simulink model "COMPONENT_MDL_Lag_QUAD_and_PEND_with_spin_rotors"  (R2021b)
settings: Solver=ode23t  StartTime=0.0  StopTime=200  FixedStep=0.001  RelTol=1e-5  EnableMultiTasking=on
undefined symbols (not defined in the file or in its folder): P_pend, P_rot, P_veh_no_props
(part 2 of 10)

== matlab function COMPONENT_MDL_Lag_QUAD_and_PEND_with_spin_rotors/bh_6DOF_and_pend/MCKGQ ==
  data: I_xx input; M output; I_xy input; I_xz input; I_yy input; I_yz input; I_zz input; Iprop_xx input; Iprop_xy input; Iprop_xz input; Iprop_yy input; Iprop_yz input; Iprop_zz input; Lx_pend input; Ly_pend input; Lz_pend input; Mbz_1 input; Mbz_2 input; Mbz_3 input; Mbz_4 input; THE_Phi input; THE_Psi input; THE_Phi_D input; THE_Psi_D input; THE_Theta input; THE_Theta_D input; THE_Phi_pend input; THE_Psi_pend input; THE_Phi_pend_D input; THE_Psi_pend_D input; THE_Theta_pend input; THE_Theta_pend_D input; Tbz_1 input; Tbz_2 input; Tbz_3 input; Tbz_4 input; Tv_Z_pend input; cg_to_mot_H input; cg_to_mot_L input; g input; m input; m_pend input; mprop input; wMOT_1 input; wMOT_2 input; wMOT_3 input; wMOT_4 input; C output; K output; G output; Q output
function [M,C,K,G,Q] = MCKGQ(I_xx,I_xy,I_xz,I_yy,I_yz,I_zz,Iprop_xx,Iprop_xy,Iprop_xz,Iprop_yy,Iprop_yz,Iprop_zz,Lx_pend,Ly_pend,Lz_pend,Mbz_1,Mbz_2,Mbz_3,Mbz_4,THE_Phi,THE_Psi,THE_Phi_D,THE_Psi_D,THE_Theta,THE_Theta_D,THE_Phi_pend,THE_Psi_pend,THE_Phi_pend_D,THE_Psi_pend_D,THE_Theta_pend,THE_Theta_pend_D,Tbz_1,Tbz_2,Tbz_3,Tbz_4,Tv_Z_pend,cg_to_mot_H,cg_to_mot_L,g,m,m_pend,mprop,wMOT_1,wMOT_2,wMOT_3,wMOT_4)
%#codegen

%    This function was generated by the Symbolic Math Toolbox version 9.0.
%    29-Sep-2021 14:44:32

et1 = (Lx_pend.^2.*m_pend.*sin(THE_Theta).*sin(THE_Phi_pend))./1.2e+1+(Ly_pend.^2.*m_pend.*sin(THE_Theta).*sin(THE_Phi_pend))./1.2e+1-(Ly_pend.^2.*m_pend.*cos(THE_Psi_pend).^2.*sin(THE_Theta).*sin(THE_Phi_pend))./1.2e+1+(Lz_pend.^2.*m_pend.*cos(THE_Psi_pend).^2.*sin(THE_Theta).*sin(THE_Phi_pend))./3.0+(Lx_pend.^2.*m_pend.*cos(THE_Theta).*cos(THE_Phi_pend).*sin(THE_Psi))./1.2e+1+(Ly_pend.^2.*m_pend.*cos(THE_Theta).*cos(THE_Phi_pend).*sin(THE_Psi))./1.2e+1-(Ly_pend.^2.*m_pend.*cos(THE_Theta).*cos(THE_Phi_pend).*cos(THE_Psi_pend).^2.*sin(THE_Psi))./1.2e+1+(Lz_pend.^2.*m_pend.*cos(THE_Theta).*cos(THE_Phi_pend).*cos(THE_Psi_pend).^2.*sin(THE_Psi))./3.0-(Ly_pend.^2.*m_pend.*cos(THE_Psi).*cos(THE_Theta).*cos(THE_Psi_pend).*cos(THE_Theta_pend).*sin(THE_Psi_pend))./1.2e+1+(Lz_pend.^2.*m_pend.*cos(THE_Psi).*cos(THE_Theta).*cos(THE_Psi_pend).*cos(THE_Theta_pend).*sin(THE_Psi_pend))./3.0+(Ly_pend.^2.*m_pend.*cos(THE_Phi_pend).*cos(THE_Psi_pend).*sin(THE_Theta).*sin(THE_Psi_pend).*sin(THE_Theta_pend))./1.2e+1;
et2 = Lz_pend.^2.*m_pend.*cos(THE_Phi_pend).*cos(THE_Psi_pend).*sin(THE_Theta).*sin(THE_Psi_pend).*sin(THE_Theta_pend).*(-1.0./3.0)+(Lz_pend.*Tv_Z_pend.*m_pend.*cos(THE_Psi_pend).*cos(THE_Theta_pend).*sin(THE_Theta).*sin(THE_Phi_pend))./2.0-(Ly_pend.^2.*m_pend.*cos(THE_Theta).*cos(THE_Psi_pend).*sin(THE_Psi).*sin(THE_Phi_pend).*sin(THE_Psi_pend).*sin(THE_Theta_pend))./1.2e+1+(Lz_pend.^2.*m_pend.*cos(THE_Theta).*cos(THE_Psi_pend).*sin(THE_Psi).*sin(THE_Phi_pend).*sin(THE_Psi_pend).*sin(THE_Theta_pend))./3.0+(Lz_pend.*Tv_Z_pend.*m_pend.*cos(THE_Theta).*cos(THE_Phi_pend).*cos(THE_Psi_pend).*cos(THE_Theta_pend).*sin(THE_Psi))./2.0;
et3 = (Ly_pend.^2.*m_pend.*cos(THE_Psi).*cos(THE_Theta))./1.2e+1+(Lz_pend.^2.*m_pend.*cos(THE_Psi).*cos(THE_Theta))./3.0+(Lx_pend.^2.*m_pend.*cos(THE_Psi).*cos(THE_Theta).*cos(THE_Theta_pend).^2)./1.2e+1-(Ly_pend.^2.*m_pend.*cos(THE_Psi).*cos(THE_Theta).*cos(THE_Theta_pend).^2)./1.2e+1+(Ly_pend.^2.*m_pend.*cos(THE_Psi).*cos(THE_Theta).*cos(THE_Psi_pend).^2.*cos(THE_Theta_pend).^2)./1.2e+1-(Lz_pend.^2.*m_pend.*cos(THE_Psi).*cos(THE_Theta).*cos(THE_Psi_pend).^2.*cos(THE_Theta_pend).^2)./3.0-(Lx_pend.^2.*m_pend.*cos(THE_Phi_pend).*cos(THE_Theta_pend).*sin(THE_Theta).*sin(THE_Theta_pend))./1.2e+1+(Ly_pend.^2.*m_pend.*cos(THE_Phi_pend).*cos(THE_Theta_pend).*sin(THE_Theta).*sin(THE_Theta_pend))./1.2e+1+(Lz_pend.*Tv_Z_pend.*m_pend.*sin(THE_Theta).*sin(THE_Phi_pend).*sin(THE_Psi_pend))./2.0+(Lx_pend.^2.*m_pend.*cos(THE_Theta).*cos(THE_Theta_pend).*sin(THE_Psi).*sin(THE_Phi_pend).*sin(THE_Theta_pend))./1.2e+1-(Ly_pend.^2.*m_pend.*cos(THE_Theta).*cos(THE_Theta_pend).*sin(THE_Psi).*sin(THE_Phi_pend).*sin(THE_Theta_pend))./1.2e+1;
et4 = Ly_pend.^2.*m_pend.*cos(THE_Psi_pend).*cos(THE_Theta_pend).*sin(THE_Theta).*sin(THE_Phi_pend).*sin(THE_Psi_pend).*(-1.0./1.2e+1)+(Lz_pend.^2.*m_pend.*cos(THE_Psi_pend).*cos(THE_Theta_pend).*sin(THE_Theta).*sin(THE_Phi_pend).*sin(THE_Psi_pend))./3.0+(Lz_pend.*Tv_Z_pend.*m_pend.*cos(THE_Theta).*cos(THE_Phi_pend).*sin(THE_Psi).*sin(THE_Psi_pend))./2.0+(Lz_pend.*Tv_Z_pend.*m_pend.*cos(THE_Phi_pend).*cos(THE_Psi_pend).*sin(THE_Theta).*sin(THE_Theta_pend))./2.0-(Ly_pend.^2.*m_pend.*cos(THE_Phi_pend).*cos(THE_Psi_pend).^2.*cos(THE_Theta_pend).*sin(THE_Theta).*sin(THE_Theta_pend))./1.2e+1+(Lz_pend.^2.*m_pend.*cos(THE_Phi_pend).*cos(THE_Psi_pend).^2.*cos(THE_Theta_pend).*sin(THE_Theta).*sin(THE_Theta_pend))./3.0-(Lz_pend.*Tv_Z_pend.*m_pend.*cos(THE_Theta).*cos(THE_Psi_pend).*sin(THE_Psi).*sin(THE_Phi_pend).*sin(THE_Theta_pend))./2.0+(Ly_pend.^2.*m_pend.*cos(THE_Theta).*cos(THE_Psi_pend).^2.*cos(THE_Theta_pend).*sin(THE_Psi).*sin(THE_Phi_pend).*sin(THE_Theta_pend))./1.2e+1-(Lz_pend.^2.*m_pend.*cos(THE_Theta).*cos(THE_Psi_pend).^2.*cos(THE_Theta_pend).*sin(THE_Psi).*sin(THE_Phi_pend).*sin(THE_Theta_pend))./3.0-(Ly_pend.^2.*m_pend.*cos(THE_Theta).*cos(THE_Phi_pend).*cos(THE_Psi_pend).*cos(THE_Theta_pend).*sin(THE_Psi).*sin(THE_Psi_pend))./1.2e+1;
et5 = (Lz_pend.^2.*m_pend.*cos(THE_Theta).*cos(THE_Phi_pend).*cos(THE_Psi_pend).*cos(THE_Theta_pend).*sin(THE_Psi).*sin(THE_Psi_pend))./3.0;
et6 = -I_xx.*sin(THE_Theta)-Iprop_xx.*sin(THE_Theta).*4.0+I_xz.*cos(THE_Psi).*cos(THE_Theta)+Iprop_xz.*cos(THE_Psi).*cos(THE_Theta).*4.0+I_xy.*cos(THE_Theta).*sin(THE_Psi)+Iprop_xy.*cos(THE_Theta).*sin(THE_Psi).*4.0-(Lx_pend.^2.*m_pend.*sin(THE_Theta))./1.2e+1-(Ly_pend.^2.*m_pend.*sin(THE_Theta))./1.2e+1-Tv_Z_pend.^2.*m_pend.*sin(THE_Theta)-cg_to_mot_H.^2.*mprop.*sin(THE_Theta).*4.0-cg_to_mot_L.^2.*mprop.*sin(THE_Theta).*2.0+(Ly_pend.^2.*m_pend.*cos(THE_Phi_pend).^2.*sin(THE_Theta))./1.2e+1+(Ly_pend.^2.*m_pend.*cos(THE_Psi_pend).^2.*sin(THE_Theta))./1.2e+1-(Lz_pend.^2.*m_pend.*cos(THE_Phi_pend).^2.*sin(THE_Theta))./3.0-(Lz_pend.^2.*m_pend.*cos(THE_Psi_pend).^2.*sin(THE_Theta))./3.0+(Lx_pend.^2.*m_pend.*cos(THE_Phi_pend).^2.*cos(THE_Theta_pend).^2.*sin(THE_Theta))./1.2e+1-(Ly_pend.^2.*m_pend.*cos(THE_Phi_pend).^2.*cos(THE_Psi_pend).^2.*sin(THE_Theta))./6.0;
et7 = Ly_pend.^2.*m_pend.*cos(THE_Phi_pend).^2.*cos(THE_Theta_pend).^2.*sin(THE_Theta).*(-1.0./1.2e+1)+Lz_pend.^2.*m_pend.*cos(THE_Phi_pend).^2.*cos(THE_Psi_pend).^2.*sin(THE_Theta).*(2.0./3.0)-(Ly_pend.^2.*m_pend.*cos(THE_Theta).*cos(THE_Phi_pend).*sin(THE_Psi).*sin(THE_Phi_pend))./1.2e+1+(Lz_pend.^2.*m_pend.*cos(THE_Theta).*cos(THE_Phi_pend).*sin(THE_Psi).*sin(THE_Phi_pend))./3.0+(Ly_pend.^2.*m_pend.*cos(THE_Phi_pend).^2.*cos(THE_Psi_pend).^2.*cos(THE_Theta_pend).^2.*sin(THE_Theta))./1.2e+1-(Lz_pend.^2.*m_pend.*cos(THE_Phi_pend).^2.*cos(THE_Psi_pend).^2.*cos(THE_Theta_pend).^2.*sin(THE_Theta))./3.0-Lz_pend.*Tv_Z_pend.*m_pend.*cos(THE_Psi_pend).*cos(THE_Theta_pend).*sin(THE_Theta)+(Lx_pend.^2.*m_pend.*cos(THE_Psi).*cos(THE_Theta).*cos(THE_Phi_pend).*cos(THE_Theta_pend).*sin(THE_Theta_pend))./1.2e+1-(Ly_pend.^2.*m_pend.*cos(THE_Psi).*cos(THE_Theta).*cos(THE_Phi_pend).*cos(THE_Theta_pend).*sin(THE_Theta_pend))./1.2e+1+(Ly_pend.^2.*m_pend.*cos(THE_Theta).*cos(THE_Psi_pend).*sin(THE_Psi).*sin(THE_Psi_pend).*sin(THE_Theta_pend))./1.2e+1;
et8 = Lz_pend.^2.*m_pend.*cos(THE_Theta).*cos(THE_Psi_pend).*sin(THE_Psi).*sin(THE_Psi_pend).*sin(THE_Theta_pend).*(-1.0./3.0)-(Lz_pend.*Tv_Z_pend.*m_pend.*cos(THE_Psi).*cos(THE_Theta).*sin(THE_Phi_pend).*sin(THE_Psi_pend))./2.0-(Lx_pend.^2.*m_pend.*cos(THE_Theta).*cos(THE_Phi_pend).*cos(THE_Theta_pend).^2.*sin(THE_Psi).*sin(THE_Phi_pend))./1.2e+1+(Ly_pend.^2.*m_pend.*cos(THE_Theta).*cos(THE_Phi_pend).*cos(THE_Psi_pend).^2.*sin(THE_Psi).*sin(THE_Phi_pend))./6.0+(Ly_pend.^2.*m_pend.*cos(THE_Theta).*cos(THE_Phi_pend).*cos(THE_Theta_pend).^2.*sin(THE_Psi).*sin(THE_Phi_pend))./1.2e+1-Lz_pend.^2.*m_pend.*cos(THE_Theta).*cos(THE_Phi_pend).*cos(THE_Psi_pend).^2.*sin(THE_Psi).*sin(THE_Phi_pend).*(2.0./3.0)-(Ly_pend.^2.*m_pend.*cos(THE_Phi_pend).*cos(THE_Psi_pend).*sin(THE_Theta).*sin(THE_Phi_pend).*sin(THE_Psi_pend).*sin(THE_Theta_pend))./6.0+Lz_pend.^2.*m_pend.*cos(THE_Phi_pend).*cos(THE_Psi_pend).*sin(THE_Theta).*sin(THE_Phi_pend).*sin(THE_Psi_pend).*sin(THE_Theta_pend).*(2.0./3.0)-(Lz_pend.*Tv_Z_pend.*m_pend.*cos(THE_Psi).*cos(THE_Theta).*cos(THE_Phi_pend).*cos(THE_Psi_pend).*sin(THE_Theta_pend))./2.0;
et9 = (Ly_pend.^2.*m_pend.*cos(THE_Psi).*cos(THE_Theta).*cos(THE_Phi_pend).*cos(THE_Psi_pend).^2.*cos(THE_Theta_pend).*sin(THE_Theta_pend))./1.2e+1-(Lz_pend.^2.*m_pend.*cos(THE_Psi).*cos(THE_Theta).*cos(THE_Phi_pend).*cos(THE_Psi_pend).^2.*cos(THE_Theta_pend).*sin(THE_Theta_pend))./3.0-(Ly_pend.^2.*m_pend.*cos(THE_Theta).*cos(THE_Phi_pend).^2.*cos(THE_Psi_pend).*sin(THE_Psi).*sin(THE_Psi_pend).*sin(THE_Theta_pend))./6.0+Lz_pend.^2.*m_pend.*cos(THE_Theta).*cos(THE_Phi_pend).^2.*cos(THE_Psi_pend).*sin(THE_Psi).*sin(THE_Psi_pend).*sin(THE_Theta_pend).*(2.0./3.0)-(Ly_pend.^2.*m_pend.*cos(THE_Theta).*cos(THE_Phi_pend).*cos(THE_Psi_pend).^2.*cos(THE_Theta_pend).^2.*sin(THE_Psi).*sin(THE_Phi_pend))./1.2e+1+(Lz_pend.^2.*m_pend.*cos(THE_Theta).*cos(THE_Phi_pend).*cos(THE_Psi_pend).^2.*cos(THE_Theta_pend).^2.*sin(THE_Psi).*sin(THE_Phi_pend))./3.0+(Ly_pend.^2.*m_pend.*cos(THE_Psi).*cos(THE_Theta).*cos(THE_Psi_pend).*cos(THE_Theta_pend).*sin(THE_Phi_pend).*sin(THE_Psi_pend))./1.2e+1-(Lz_pend.^2.*m_pend.*cos(THE_Psi).*cos(THE_Theta).*cos(THE_Psi_pend).*cos(THE_Theta_pend).*sin(THE_Phi_pend).*sin(THE_Psi_pend))./3.0;
et10 = -I_yz.*cos(THE_Theta)-Iprop_yz.*cos(THE_Theta).*4.0-I_xy.*cos(THE_Psi).*sin(THE_Theta)-Iprop_xy.*cos(THE_Psi).*sin(THE_Theta).*4.0+I_xz.*sin(THE_Psi).*sin(THE_Theta)+Iprop_xz.*sin(THE_Psi).*sin(THE_Theta).*4.0+I_yz.*cos(THE_Psi).^2.*cos(THE_Theta).*2.0+Iprop_yz.*cos(THE_Psi).^2.*cos(THE_Theta).*8.0+I_yy.*cos(THE_Psi).*cos(THE_Theta).*sin(THE_Psi)-I_zz.*cos(THE_Psi).*cos(THE_Theta).*sin(THE_Psi)+Iprop_yy.*cos(THE_Psi).*cos(THE_Theta).*sin(THE_Psi).*4.0-Iprop_zz.*cos(THE_Psi).*cos(THE_Theta).*sin(THE_Psi).*4.0+(Lx_pend.^2.*m_pend.*cos(THE_Psi).*cos(THE_Theta).*sin(THE_Psi))./1.2e+1-(Ly_pend.^2.*m_pend.*cos(THE_Psi).*cos(THE_Theta).*sin(THE_Psi))./1.2e+1+Tv_Z_pend.^2.*m_pend.*cos(THE_Psi).*cos(THE_Theta).*sin(THE_Psi)+cg_to_mot_H.^2.*mprop.*cos(THE_Psi).*cos(THE_Theta).*sin(THE_Psi).*4.0-cg_to_mot_L.^2.*mprop.*cos(THE_Psi).*cos(THE_Theta).*sin(THE_Psi).*2.0-(Lx_pend.^2.*m_pend.*cos(THE_Theta).*cos(THE_Theta_pend).*sin(THE_Phi_pend).*sin(THE_Theta_pend))./1.2e+1+(Ly_pend.^2.*m_pend.*cos(THE_Psi).*cos(THE_Phi_pend).*sin(THE_Theta).*sin(THE_Phi_pend))./1.2e+1;
et11 = (Ly_pend.^2.*m_pend.*cos(THE_Theta).*cos(THE_Theta_pend).*sin(THE_Phi_pend).*sin(THE_Theta_pend))./1.2e+1-(Lz_pend.^2.*m_pend.*cos(THE_Psi).*cos(THE_Phi_pend).*sin(THE_Theta).*sin(THE_Phi_pend))./3.0-(Lz_pend.*Tv_Z_pend.*m_pend.*cos(THE_Theta).*cos(THE_Phi_pend).*sin(THE_Psi_pend))./2.0-(Lx_pend.^2.*m_pend.*cos(THE_Psi).*cos(THE_Theta).*cos(THE_Theta_pend).^2.*sin(THE_Psi))./6.0+(Ly_pend.^2.*m_pend.*cos(THE_Psi).*cos(THE_Theta).*cos(THE_Phi_pend).^2.*sin(THE_Psi))./1.2e+1+(Ly_pend.^2.*m_pend.*cos(THE_Psi).*cos(THE_Theta).*cos(THE_Psi_pend).^2.*sin(THE_Psi))./1.2e+1+(Ly_pend.^2.*m_pend.*cos(THE_Psi).*cos(THE_Theta).*cos(THE_Theta_pend).^2.*sin(THE_Psi))./6.0-(Lz_pend.^2.*m_pend.*cos(THE_Psi).*cos(THE_Theta).*cos(THE_Phi_pend).^2.*sin(THE_Psi))./3.0-(Lz_pend.^2.*m_pend.*cos(THE_Psi).*cos(THE_Theta).*cos(THE_Psi_pend).^2.*sin(THE_Psi))./3.0+(Ly_pend.^2.*m_pend.*cos(THE_Theta).*cos(THE_Phi_pend).*cos(THE_Psi_pend).*cos(THE_Theta_pend).*sin(THE_Psi_pend))./1.2e+1-(Lz_pend.^2.*m_pend.*cos(THE_Theta).*cos(THE_Phi_pend).*cos(THE_Psi_pend).*cos(THE_Theta_pend).*sin(THE_Psi_pend))./3.0;
et12 = (Lx_pend.^2.*m_pend.*cos(THE_Phi_pend).*cos(THE_Theta_pend).*sin(THE_Psi).*sin(THE_Theta).*sin(THE_Theta_pend))./1.2e+1-(Ly_pend.^2.*m_pend.*cos(THE_Psi).*cos(THE_Psi_pend).*sin(THE_Theta).*sin(THE_Psi_pend).*sin(THE_Theta_pend))./1.2e+1-(Ly_pend.^2.*m_pend.*cos(THE_Phi_pend).*cos(THE_Theta_pend).*sin(THE_Psi).*sin(THE_Theta).*sin(THE_Theta_pend))./1.2e+1+(Lz_pend.^2.*m_pend.*cos(THE_Psi).*cos(THE_Psi_pend).*sin(THE_Theta).*sin(THE_Psi_pend).*sin(THE_Theta_pend))./3.0+(Lz_pend.*Tv_Z_pend.*m_pend.*cos(THE_Theta).*cos(THE_Psi_pend).*sin(THE_Phi_pend).*sin(THE_Theta_pend))./2.0-(Lz_pend.*Tv_Z_pend.*m_pend.*sin(THE_Psi).*sin(THE_Theta).*sin(THE_Phi_pend).*sin(THE_Psi_pend))./2.0+(Lx_pend.^2.*m_pend.*cos(THE_Psi).*cos(THE_Phi_pend).*cos(THE_Theta_pend).^2.*sin(THE_Theta).*sin(THE_Phi_pend))./1.2e+1+(Lx_pend.^2.*m_pend.*cos(THE_Psi).^2.*cos(THE_Theta).*cos(THE_Theta_pend).*sin(THE_Phi_pend).*sin(THE_Theta_pend))./6.0-(Ly_pend.^2.*m_pend.*cos(THE_Psi).*cos(THE_Phi_pend).*cos(THE_Psi_pend).^2.*sin(THE_Theta).*sin(THE_Phi_pend))./6.0-(Ly_pend.^2.*m_pend.*cos(THE_Psi).*cos(THE_Phi_pend).*cos(THE_Theta_pend).^2.*sin(THE_Theta).*sin(THE_Phi_pend))./1.2e+1;
et13 = Ly_pend.^2.*m_pend.*cos(THE_Psi).^2.*cos(THE_Theta).*cos(THE_Theta_pend).*sin(THE_Phi_pend).*sin(THE_Theta_pend).*(-1.0./6.0)-(Ly_pend.^2.*m_pend.*cos(THE_Theta).*cos(THE_Psi_pend).^2.*cos(THE_Theta_pend).*sin(THE_Phi_pend).*sin(THE_Theta_pend))./1.2e+1+Lz_pend.^2.*m_pend.*cos(THE_Psi).*cos(THE_Phi_pend).*cos(THE_Psi_pend).^2.*sin(THE_Theta).*sin(THE_Phi_pend).*(2.0./3.0)+(Lz_pend.^2.*m_pend.*cos(THE_Theta).*cos(THE_Psi_pend).^2.*cos(THE_Theta_pend).*sin(THE_Phi_pend).*sin(THE_Theta_pend))./3.0+Lz_pend.*Tv_Z_pend.*m_pend.*cos(THE_Psi).^2.*cos(THE_Theta).*cos(THE_Phi_pend).*sin(THE_Psi_pend)+(Lx_pend.^2.*m_pend.*cos(THE_Psi).*cos(THE_Theta).*cos(THE_Phi_pend).^2.*cos(THE_Theta_pend).^2.*sin(THE_Psi))./1.2e+1-(Ly_pend.^2.*m_pend.*cos(THE_Psi).*cos(THE_Theta).*cos(THE_Phi_pend).^2.*cos(THE_Psi_pend).^2.*sin(THE_Psi))./6.0-(Ly_pend.^2.*m_pend.*cos(THE_Psi).*cos(THE_Theta).*cos(THE_Phi_pend).^2.*cos(THE_Theta_pend).^2.*sin(THE_Psi))./1.2e+1-(Ly_pend.^2.*m_pend.*cos(THE_Psi).*cos(THE_Theta).*cos(THE_Psi_pend).^2.*cos(THE_Theta_pend).^2.*sin(THE_Psi))./6.0;
et14 = Lz_pend.^2.*m_pend.*cos(THE_Psi).*cos(THE_Theta).*cos(THE_Phi_pend).^2.*cos(THE_Psi_pend).^2.*sin(THE_Psi).*(2.0./3.0)+Lz_pend.^2.*m_pend.*cos(THE_Psi).*cos(THE_Theta).*cos(THE_Psi_pend).^2.*cos(THE_Theta_pend).^2.*sin(THE_Psi).*(2.0./3.0)+(Ly_pend.^2.*m_pend.*cos(THE_Psi_pend).*cos(THE_Theta_pend).*sin(THE_Psi).*sin(THE_Theta).*sin(THE_Phi_pend).*sin(THE_Psi_pend))./1.2e+1-(Lz_pend.^2.*m_pend.*cos(THE_Psi_pend).*cos(THE_Theta_pend).*sin(THE_Psi).*sin(THE_Theta).*sin(THE_Phi_pend).*sin(THE_Psi_pend))./3.0+Lz_pend.*Tv_Z_pend.*m_pend.*cos(THE_Psi).*cos(THE_Theta).*cos(THE_Psi_pend).*cos(THE_Theta_pend).*sin(THE_Psi)-(Lz_pend.*Tv_Z_pend.*m_pend.*cos(THE_Phi_pend).*cos(THE_Psi_pend).*sin(THE_Psi).*sin(THE_Theta).*sin(THE_Theta_pend))./2.0-(Ly_pend.^2.*m_pend.*cos(THE_Psi).^2.*cos(THE_Theta).*cos(THE_Phi_pend).*cos(THE_Psi_pend).*cos(THE_Theta_pend).*sin(THE_Psi_pend))./6.0+Lz_pend.^2.*m_pend.*cos(THE_Psi).^2.*cos(THE_Theta).*cos(THE_Phi_pend).*cos(THE_Psi_pend).*cos(THE_Theta_pend).*sin(THE_Psi_pend).*(2.0./3.0)+(Ly_pend.^2.*m_pend.*cos(THE_Psi).*cos(THE_Phi_pend).^2.*cos(THE_Psi_pend).*sin(THE_Theta).*sin(THE_Psi_pend).*sin(THE_Theta_pend))./6.0;
et15 = (Ly_pend.^2.*m_pend.*cos(THE_Phi_pend).*cos(THE_Psi_pend).^2.*cos(THE_Theta_pend).*sin(THE_Psi).*sin(THE_Theta).*sin(THE_Theta_pend))./1.2e+1-Lz_pend.^2.*m_pend.*cos(THE_Psi).*cos(THE_Phi_pend).^2.*cos(THE_Psi_pend).*sin(THE_Theta).*sin(THE_Psi_pend).*sin(THE_Theta_pend).*(2.0./3.0)-(Lz_pend.^2.*m_pend.*cos(THE_Phi_pend).*cos(THE_Psi_pend).^2.*cos(THE_Theta_pend).*sin(THE_Psi).*sin(THE_Theta).*sin(THE_Theta_pend))./3.0-Lz_pend.*Tv_Z_pend.*m_pend.*cos(THE_Psi).^2.*cos(THE_Theta).*cos(THE_Psi_pend).*sin(THE_Phi_pend).*sin(THE_Theta_pend)+(Ly_pend.^2.*m_pend.*cos(THE_Psi).*cos(THE_Phi_pend).*cos(THE_Psi_pend).^2.*cos(THE_Theta_pend).^2.*sin(THE_Theta).*sin(THE_Phi_pend))./1.2e+1+(Ly_pend.^2.*m_pend.*cos(THE_Psi).^2.*cos(THE_Theta).*cos(THE_Psi_pend).^2.*cos(THE_Theta_pend).*sin(THE_Phi_pend).*sin(THE_Theta_pend))./6.0-(Lz_pend.^2.*m_pend.*cos(THE_Psi).*cos(THE_Phi_pend).*cos(THE_Psi_pend).^2.*cos(THE_Theta_pend).^2.*sin(THE_Theta).*sin(THE_Phi_pend))./3.0-Lz_pend.^2.*m_pend.*cos(THE_Psi).^2.*cos(THE_Theta).*cos(THE_Psi_pend).^2.*cos(THE_Theta_pend).*sin(THE_Phi_pend).*sin(THE_Theta_pend).*(2.0./3.0);
et16 = (Ly_pend.^2.*m_pend.*cos(THE_Psi).*cos(THE_Theta).*cos(THE_Phi_pend).^2.*cos(THE_Psi_pend).^2.*cos(THE_Theta_pend).^2.*sin(THE_Psi))./1.2e+1-(Lz_pend.^2.*m_pend.*cos(THE_Psi).*cos(THE_Theta).*cos(THE_Phi_pend).^2.*cos(THE_Psi_pend).^2.*cos(THE_Theta_pend).^2.*sin(THE_Psi))./3.0-(Ly_pend.^2.*m_pend.*cos(THE_Psi).*cos(THE_Theta).*cos(THE_Phi_pend).*cos(THE_Psi_pend).*sin(THE_Psi).*sin(THE_Phi_pend).*sin(THE_Psi_pend).*sin(THE_Theta_pend))./6.0+Lz_pend.^2.*m_pend.*cos(THE_Psi).*cos(THE_Theta).*cos(THE_Phi_pend).*cos(THE_Psi_pend).*sin(THE_Psi).*sin(THE_Phi_pend).*sin(THE_Psi_pend).*sin(THE_Theta_pend).*(2.0./3.0);
et17 = I_xx+Iprop_xx.*4.0+(Lx_pend.^2.*m_pend)./1.2e+1+(Ly_pend.^2.*m_pend)./1.2e+1+Tv_Z_pend.^2.*m_pend+cg_to_mot_H.^2.*mprop.*4.0+cg_to_mot_L.^2.*mprop.*2.0-I_xx.*cos(THE_Theta).^2+I_yy.*cos(THE_Theta).^2-Iprop_xx.*cos(THE_Theta).^2.*4.0+Iprop_yy.*cos(THE_Theta).^2.*4.0-(Ly_pend.^2.*m_pend.*cos(THE_Theta).^2)./1.2e+1-(Ly_pend.^2.*m_pend.*cos(THE_Phi_pend).^2)./1.2e+1-(Ly_pend.^2.*m_pend.*cos(THE_Psi_pend).^2)./1.2e+1+(Lz_pend.^2.*m_pend.*cos(THE_Theta).^2)./3.0+(Lz_pend.^2.*m_pend.*cos(THE_Phi_pend).^2)./3.0+(Lz_pend.^2.*m_pend.*cos(THE_Psi_pend).^2)./3.0-I_yy.*cos(THE_Psi).^2.*cos(THE_Theta).^2+I_zz.*cos(THE_Psi).^2.*cos(THE_Theta).^2-Iprop_yy.*cos(THE_Psi).^2.*cos(THE_Theta).^2.*4.0+Iprop_zz.*cos(THE_Psi).^2.*cos(THE_Theta).^2.*4.0;
et18 = I_yz.*cos(THE_Psi).*cos(THE_Theta).^2.*sin(THE_Psi).*2.0+Iprop_yz.*cos(THE_Psi).*cos(THE_Theta).^2.*sin(THE_Psi).*8.0-(Lx_pend.^2.*m_pend.*cos(THE_Psi).^2.*cos(THE_Theta).^2)./1.2e+1-(Lx_pend.^2.*m_pend.*cos(THE_Theta).^2.*cos(THE_Theta_pend).^2)./1.2e+1-(Lx_pend.^2.*m_pend.*cos(THE_Phi_pend).^2.*cos(THE_Theta_pend).^2)./1.2e+1+(Ly_pend.^2.*m_pend.*cos(THE_Psi).^2.*cos(THE_Theta).^2)./1.2e+1+(Ly_pend.^2.*m_pend.*cos(THE_Theta).^2.*cos(THE_Phi_pend).^2)./6.0+(Ly_pend.^2.*m_pend.*cos(THE_Theta).^2.*cos(THE_Psi_pend).^2)./6.0+(Ly_pend.^2.*m_pend.*cos(THE_Theta).^2.*cos(THE_Theta_pend).^2)./1.2e+1+(Ly_pend.^2.*m_pend.*cos(THE_Phi_pend).^2.*cos(THE_Psi_pend).^2)./6.0+(Ly_pend.^2.*m_pend.*cos(THE_Phi_pend).^2.*cos(THE_Theta_pend).^2)./1.2e+1-Lz_pend.^2.*m_pend.*cos(THE_Theta).^2.*cos(THE_Phi_pend).^2.*(2.0./3.0);
et19 = Lz_pend.^2.*m_pend.*cos(THE_Theta).^2.*cos(THE_Psi_pend).^2.*(-2.0./3.0)-Lz_pend.^2.*m_pend.*cos(THE_Phi_pend).^2.*cos(THE_Psi_pend).^2.*(2.0./3.0)-Tv_Z_pend.^2.*m_pend.*cos(THE_Psi).^2.*cos(THE_Theta).^2-cg_to_mot_H.^2.*mprop.*cos(THE_Psi).^2.*cos(THE_Theta).^2.*4.0+cg_to_mot_L.^2.*mprop.*cos(THE_Psi).^2.*cos(THE_Theta).^2.*2.0-I_xz.*cos(THE_Psi).*cos(THE_Theta).*sin(THE_Theta).*2.0-Iprop_xz.*cos(THE_Psi).*cos(THE_Theta).*sin(THE_Theta).*8.0-I_xy.*cos(THE_Theta).*sin(THE_Psi).*sin(THE_Theta).*2.0-Iprop_xy.*cos(THE_Theta).*sin(THE_Psi).*sin(THE_Theta).*8.0+(Lx_pend.^2.*m_pend.*cos(THE_Psi).^2.*cos(THE_Theta).^2.*cos(THE_Theta_pend).^2)./6.0+(Lx_pend.^2.*m_pend.*cos(THE_Theta).^2.*cos(THE_Phi_pend).^2.*cos(THE_Theta_pend).^2)./6.0-(Ly_pend.^2.*m_pend.*cos(THE_Psi).^2.*cos(THE_Theta).^2.*cos(THE_Phi_pend).^2)./1.2e+1;
et20 = Ly_pend.^2.*m_pend.*cos(THE_Psi).^2.*cos(THE_Theta).^2.*cos(THE_Psi_pend).^2.*(-1.0./1.2e+1)-(Ly_pend.^2.*m_pend.*cos(THE_Psi).^2.*cos(THE_Theta).^2.*cos(THE_Theta_pend).^2)./6.0-(Ly_pend.^2.*m_pend.*cos(THE_Theta).^2.*cos(THE_Phi_pend).^2.*cos(THE_Psi_pend).^2)./3.0-(Ly_pend.^2.*m_pend.*cos(THE_Theta).^2.*cos(THE_Phi_pend).^2.*cos(THE_Theta_pend).^2)./6.0-(Ly_pend.^2.*m_pend.*cos(THE_Theta).^2.*cos(THE_Psi_pend).^2.*cos(THE_Theta_pend).^2)./1.2e+1-(Ly_pend.^2.*m_pend.*cos(THE_Phi_pend).^2.*cos(THE_Psi_pend).^2.*cos(THE_Theta_pend).^2)./1.2e+1+(Lz_pend.^2.*m_pend.*cos(THE_Psi).^2.*cos(THE_Theta).^2.*cos(THE_Phi_pend).^2)./3.0+(Lz_pend.^2.*m_pend.*cos(THE_Psi).^2.*cos(THE_Theta).^2.*cos(THE_Psi_pend).^2)./3.0+Lz_pend.^2.*m_pend.*cos(THE_Theta).^2.*cos(THE_Phi_pend).^2.*cos(THE_Psi_pend).^2.*(4.0./3.0);
et21 = (Lz_pend.^2.*m_pend.*cos(THE_Theta).^2.*cos(THE_Psi_pend).^2.*cos(THE_Theta_pend).^2)./3.0+(Lz_pend.^2.*m_pend.*cos(THE_Phi_pend).^2.*cos(THE_Psi_pend).^2.*cos(THE_Theta_pend).^2)./3.0+Lz_pend.*Tv_Z_pend.*m_pend.*cos(THE_Psi_pend).*cos(THE_Theta_pend)-(Lx_pend.^2.*m_pend.*cos(THE_Psi).^2.*cos(THE_Theta).^2.*cos(THE_Phi_pend).^2.*cos(THE_Theta_pend).^2)./1.2e+1+(Ly_pend.^2.*m_pend.*cos(THE_Psi).^2.*cos(THE_Theta).^2.*cos(THE_Phi_pend).^2.*cos(THE_Psi_pend).^2)./6.0+(Ly_pend.^2.*m_pend.*cos(THE_Psi).^2.*cos(THE_Theta).^2.*cos(THE_Phi_pend).^2.*cos(THE_Theta_pend).^2)./1.2e+1+(Ly_pend.^2.*m_pend.*cos(THE_Psi).^2.*cos(THE_Theta).^2.*cos(THE_Psi_pend).^2.*cos(THE_Theta_pend).^2)./6.0+(Ly_pend.^2.*m_pend.*cos(THE_Theta).^2.*cos(THE_Phi_pend).^2.*cos(THE_Psi_pend).^2.*cos(THE_Theta_pend).^2)./6.0-Lz_pend.^2.*m_pend.*cos(THE_Psi).^2.*cos(THE_Theta).^2.*cos(THE_Phi_pend).^2.*cos(THE_Psi_pend).^2.*(2.0./3.0);
et22 = Lz_pend.^2.*m_pend.*cos(THE_Psi).^2.*cos(THE_Theta).^2.*cos(THE_Psi_pend).^2.*cos(THE_Theta_pend).^2.*(-2.0./3.0)-Lz_pend.^2.*m_pend.*cos(THE_Theta).^2.*cos(THE_Phi_pend).^2.*cos(THE_Psi_pend).^2.*cos(THE_Theta_pend).^2.*(2.0./3.0)-Lz_pend.*Tv_Z_pend.*m_pend.*cos(THE_Psi).^2.*cos(THE_Theta).^2.*cos(THE_Psi_pend).*cos(THE_Theta_pend)+(Ly_pend.^2.*m_pend.*cos(THE_Theta).*cos(THE_Phi_pend).*sin(THE_Psi).*sin(THE_Theta).*sin(THE_Phi_pend))./6.0+(Ly_pend.^2.*m_pend.*cos(THE_Phi_pend).*cos(THE_Psi_pend).*sin(THE_Phi_pend).*sin(THE_Psi_pend).*sin(THE_Theta_pend))./6.0-Lz_pend.^2.*m_pend.*cos(THE_Theta).*cos(THE_Phi_pend).*sin(THE_Psi).*sin(THE_Theta).*sin(THE_Phi_pend).*(2.0./3.0)-Lz_pend.^2.*m_pend.*cos(THE_Phi_pend).*cos(THE_Psi_pend).*sin(THE_Phi_pend).*sin(THE_Psi_pend).*sin(THE_Theta_pend).*(2.0./3.0)-(Ly_pend.^2.*m_pend.*cos(THE_Psi).^2.*cos(THE_Theta).^2.*cos(THE_Phi_pend).^2.*cos(THE_Psi_pend).^2.*cos(THE_Theta_pend).^2)./1.2e+1+(Lz_pend.^2.*m_pend.*cos(THE_Psi).^2.*cos(THE_Theta).^2.*cos(THE_Phi_pend).^2.*cos(THE_Psi_pend).^2.*cos(THE_Theta_pend).^2)./3.0;
et23 = Ly_pend.^2.*m_pend.*cos(THE_Theta).*cos(THE_Psi_pend).*sin(THE_Psi).*sin(THE_Theta).*sin(THE_Psi_pend).*sin(THE_Theta_pend).*(-1.0./6.0)+Lz_pend.^2.*m_pend.*cos(THE_Theta).*cos(THE_Psi_pend).*sin(THE_Psi).*sin(THE_Theta).*sin(THE_Psi_pend).*sin(THE_Theta_pend).*(2.0./3.0)+Lz_pend.*Tv_Z_pend.*m_pend.*cos(THE_Psi).*cos(THE_Theta).*sin(THE_Theta).*sin(THE_Phi_pend).*sin(THE_Psi_pend)+(Lx_pend.^2.*m_pend.*cos(THE_Theta).*cos(THE_Phi_pend).*cos(THE_Theta_pend).^2.*sin(THE_Psi).*sin(THE_Theta).*sin(THE_Phi_pend))./6.0+(Lx_pend.^2.*m_pend.*cos(THE_Psi).*cos(THE_Theta).^2.*cos(THE_Theta_pend).*sin(THE_Psi).*sin(THE_Phi_pend).*sin(THE_Theta_pend))./6.0-(Ly_pend.^2.*m_pend.*cos(THE_Theta).*cos(THE_Phi_pend).*cos(THE_Psi_pend).^2.*sin(THE_Psi).*sin(THE_Theta).*sin(THE_Phi_pend))./3.0-(Ly_pend.^2.*m_pend.*cos(THE_Theta).*cos(THE_Phi_pend).*cos(THE_Theta_pend).^2.*sin(THE_Psi).*sin(THE_Theta).*sin(THE_Phi_pend))./6.0-(Ly_pend.^2.*m_pend.*cos(THE_Psi).*cos(THE_Theta).^2.*cos(THE_Theta_pend).*sin(THE_Psi).*sin(THE_Phi_pend).*sin(THE_Theta_pend))./6.0-(Ly_pend.^2.*m_pend.*cos(THE_Theta).^2.*cos(THE_Phi_pend).*cos(THE_Psi_pend).*sin(THE_Phi_pend).*sin(THE_Psi_pend).*sin(THE_Theta_pend))./3.0;
et24 = Lz_pend.^2.*m_pend.*cos(THE_Theta).*cos(THE_Phi_pend).*cos(THE_Psi_pend).^2.*sin(THE_Psi).*sin(THE_Theta).*sin(THE_Phi_pend).*(4.0./3.0)+Lz_pend.^2.*m_pend.*cos(THE_Theta).^2.*cos(THE_Phi_pend).*cos(THE_Psi_pend).*sin(THE_Phi_pend).*sin(THE_Psi_pend).*sin(THE_Theta_pend).*(4.0./3.0)+Lz_pend.*Tv_Z_pend.*m_pend.*cos(THE_Psi).*cos(THE_Theta).^2.*cos(THE_Phi_pend).*sin(THE_Psi).*sin(THE_Psi_pend)-(Lx_pend.^2.*m_pend.*cos(THE_Psi).*cos(THE_Theta).*cos(THE_Phi_pend).*cos(THE_Theta_pend).*sin(THE_Theta).*sin(THE_Theta_pend))./6.0+(Ly_pend.^2.*m_pend.*cos(THE_Psi).*cos(THE_Theta).*cos(THE_Phi_pend).*cos(THE_Theta_pend).*sin(THE_Theta).*sin(THE_Theta_pend))./6.0+(Ly_pend.^2.*m_pend.*cos(THE_Theta).*cos(THE_Phi_pend).^2.*cos(THE_Psi_pend).*sin(THE_Psi).*sin(THE_Theta).*sin(THE_Psi_pend).*sin(THE_Theta_pend))./3.0-Lz_pend.^2.*m_pend.*cos(THE_Theta).*cos(THE_Phi_pend).^2.*cos(THE_Psi_pend).*sin(THE_Psi).*sin(THE_Theta).*sin(THE_Psi_pend).*sin(THE_Theta_pend).*(4.0./3.0)-Lz_pend.*Tv_Z_pend.*m_pend.*cos(THE_Psi).*cos(THE_Theta).^2.*cos(THE_Psi_pend).*sin(THE_Psi).*sin(THE_Phi_pend).*sin(THE_Theta_pend)+(Ly_pend.^2.*m_pend.*cos(THE_Theta).*cos(THE_Phi_pend).*cos(THE_Psi_pend).^2.*cos(THE_Theta_pend).^2.*sin(THE_Psi).*sin(THE_Theta).*sin(THE_Phi_pend))./6.0;
et25 = (Ly_pend.^2.*m_pend.*cos(THE_Psi).*cos(THE_Theta).^2.*cos(THE_Psi_pend).^2.*cos(THE_Theta_pend).*sin(THE_Psi).*sin(THE_Phi_pend).*sin(THE_Theta_pend))./6.0+(Ly_pend.^2.*m_pend.*cos(THE_Psi).^2.*cos(THE_Theta).^2.*cos(THE_Phi_pend).*cos(THE_Psi_pend).*sin(THE_Phi_pend).*sin(THE_Psi_pend).*sin(THE_Theta_pend))./6.0-Lz_pend.^2.*m_pend.*cos(THE_Theta).*cos(THE_Phi_pend).*cos(THE_Psi_pend).^2.*cos(THE_Theta_pend).^2.*sin(THE_Psi).*sin(THE_Theta).*sin(THE_Phi_pend).*(2.0./3.0)-Lz_pend.^2.*m_pend.*cos(THE_Psi).*cos(THE_Theta).^2.*cos(THE_Psi_pend).^2.*cos(THE_Theta_pend).*sin(THE_Psi).*sin(THE_Phi_pend).*sin(THE_Theta_pend).*(2.0./3.0)-Lz_pend.^2.*m_pend.*cos(THE_Psi).^2.*cos(THE_Theta).^2.*cos(THE_Phi_pend).*cos(THE_Psi_pend).*sin(THE_Phi_pend).*sin(THE_Psi_pend).*sin(THE_Theta_pend).*(2.0./3.0)-(Ly_pend.^2.*m_pend.*cos(THE_Psi).*cos(THE_Theta).*cos(THE_Psi_pend).*cos(THE_Theta_pend).*sin(THE_Theta).*sin(THE_Phi_pend).*sin(THE_Psi_pend))./6.0+Lz_pend.^2.*m_pend.*cos(THE_Psi).*cos(THE_Theta).*cos(THE_Psi_pend).*cos(THE_Theta_pend).*sin(THE_Theta).*sin(THE_Phi_pend).*sin(THE_Psi_pend).*(2.0./3.0)+Lz_pend.*Tv_Z_pend.*m_pend.*cos(THE_Psi).*cos(THE_Theta).*cos(THE_Phi_pend).*cos(THE_Psi_pend).*sin(THE_Theta).*sin(THE_Theta_pend);
et26 = Ly_pend.^2.*m_pend.*cos(THE_Psi).*cos(THE_Theta).^2.*cos(THE_Phi_pend).*cos(THE_Psi_pend).*cos(THE_Theta_pend).*sin(THE_Psi).*sin(THE_Psi_pend).*(-1.0./6.0)-(Ly_pend.^2.*m_pend.*cos(THE_Psi).*cos(THE_Theta).*cos(THE_Phi_pend).*cos(THE_Psi_pend).^2.*cos(THE_Theta_pend).*sin(THE_Theta).*sin(THE_Theta_pend))./6.0+Lz_pend.^2.*m_pend.*cos(THE_Psi).*cos(THE_Theta).^2.*cos(THE_Phi_pend).*cos(THE_Psi_pend).*cos(THE_Theta_pend).*sin(THE_Psi).*sin(THE_Psi_pend).*(2.0./3.0)+Lz_pend.^2.*m_pend.*cos(THE_Psi).*cos(THE_Theta).*cos(THE_Phi_pend).*cos(THE_Psi_pend).^2.*cos(THE_Theta_pend).*sin(THE_Theta).*sin(THE_Theta_pend).*(2.0./3.0);
et27 = Ly_pend.^2.*m_pend.*sin(THE_Psi).*(-1.0./1.2e+1)-(Lz_pend.^2.*m_pend.*sin(THE_Psi))./3.0-(Lx_pend.^2.*m_pend.*cos(THE_Theta_pend).^2.*sin(THE_Psi))./1.2e+1+(Ly_pend.^2.*m_pend.*cos(THE_Theta_pend).^2.*sin(THE_Psi))./1.2e+1-(Ly_pend.^2.*m_pend.*cos(THE_Psi_pend).^2.*cos(THE_Theta_pend).^2.*sin(THE_Psi))./1.2e+1+(Lz_pend.^2.*m_pend.*cos(THE_Psi_pend).^2.*cos(THE_Theta_pend).^2.*sin(THE_Psi))./3.0+(Lx_pend.^2.*m_pend.*cos(THE_Psi).*cos(THE_Theta_pend).*sin(THE_Phi_pend).*sin(THE_Theta_pend))./1.2e+1-(Ly_pend.^2.*m_pend.*cos(THE_Psi).*cos(THE_Theta_pend).*sin(THE_Phi_pend).*sin(THE_Theta_pend))./1.2e+1+(Lz_pend.*Tv_Z_pend.*m_pend.*cos(THE_Psi).*cos(THE_Phi_pend).*sin(THE_Psi_pend))./2.0-(Ly_pend.^2.*m_pend.*cos(THE_Psi).*cos(THE_Phi_pend).*cos(THE_Psi_pend).*cos(THE_Theta_pend).*sin(THE_Psi_pend))./1.2e+1+(Lz_pend.^2.*m_pend.*cos(THE_Psi).*cos(THE_Phi_pend).*cos(THE_Psi_pend).*cos(THE_Theta_pend).*sin(THE_Psi_pend))./3.0-(Lz_pend.*Tv_Z_pend.*m_pend.*cos(THE_Psi).*cos(THE_Psi_pend).*sin(THE_Phi_pend).*sin(THE_Theta_pend))./2.0;
et28 = (Ly_pend.^2.*m_pend.*cos(THE_Psi).*cos(THE_Psi_pend).^2.*cos(THE_Theta_pend).*sin(THE_Phi_pend).*sin(THE_Theta_pend))./1.2e+1-(Lz_pend.^2.*m_pend.*cos(THE_Psi).*cos(THE_Psi_pend).^2.*cos(THE_Theta_pend).*sin(THE_Phi_pend).*sin(THE_Theta_pend))./3.0;
et29 = I_xy.*cos(THE_Psi)+Iprop_xy.*cos(THE_Psi).*4.0-I_xz.*sin(THE_Psi)-Iprop_xz.*sin(THE_Psi).*4.0-(Ly_pend.^2.*m_pend.*cos(THE_Psi).*cos(THE_Phi_pend).*sin(THE_Phi_pend))./1.2e+1+(Lz_pend.^2.*m_pend.*cos(THE_Psi).*cos(THE_Phi_pend).*sin(THE_Phi_pend))./3.0-(Lx_pend.^2.*m_pend.*cos(THE_Phi_pend).*cos(THE_Theta_pend).*sin(THE_Psi).*sin(THE_Theta_pend))./1.2e+1+(Ly_pend.^2.*m_pend.*cos(THE_Psi).*cos(THE_Psi_pend).*sin(THE_Psi_pend).*sin(THE_Theta_pend))./1.2e+1+(Ly_pend.^2.*m_pend.*cos(THE_Phi_pend).*cos(THE_Theta_pend).*sin(THE_Psi).*sin(THE_Theta_pend))./1.2e+1-(Lz_pend.^2.*m_pend.*cos(THE_Psi).*cos(THE_Psi_pend).*sin(THE_Psi_pend).*sin(THE_Theta_pend))./3.0+(Lz_pend.*Tv_Z_pend.*m_pend.*sin(THE_Psi).*sin(THE_Phi_pend).*sin(THE_Psi_pend))./2.0-(Lx_pend.^2.*m_pend.*cos(THE_Psi).*cos(THE_Phi_pend).*cos(THE_Theta_pend).^2.*sin(THE_Phi_pend))./1.2e+1+(Ly_pend.^2.*m_pend.*cos(THE_Psi).*cos(THE_Phi_pend).*cos(THE_Psi_pend).^2.*sin(THE_Phi_pend))./6.0+(Ly_pend.^2.*m_pend.*cos(THE_Psi).*cos(THE_Phi_pend).*cos(THE_Theta_pend).^2.*sin(THE_Phi_pend))./1.2e+1;
et30 = Lz_pend.^2.*m_pend.*cos(THE_Psi).*cos(THE_Phi_pend).*cos(THE_Psi_pend).^2.*sin(THE_Phi_pend).*(-2.0./3.0)-(Ly_pend.^2.*m_pend.*cos(THE_Psi_pend).*cos(THE_Theta_pend).*sin(THE_Psi).*sin(THE_Phi_pend).*sin(THE_Psi_pend))./1.2e+1+(Lz_pend.^2.*m_pend.*cos(THE_Psi_pend).*cos(THE_Theta_pend).*sin(THE_Psi).*sin(THE_Phi_pend).*sin(THE_Psi_pend))./3.0+(Lz_pend.*Tv_Z_pend.*m_pend.*cos(THE_Phi_pend).*cos(THE_Psi_pend).*sin(THE_Psi).*sin(THE_Theta_pend))./2.0-(Ly_pend.^2.*m_pend.*cos(THE_Psi).*cos(THE_Phi_pend).^2.*cos(THE_Psi_pend).*sin(THE_Psi_pend).*sin(THE_Theta_pend))./6.0-(Ly_pend.^2.*m_pend.*cos(THE_Phi_pend).*cos(THE_Psi_pend).^2.*cos(THE_Theta_pend).*sin(THE_Psi).*sin(THE_Theta_pend))./1.2e+1+Lz_pend.^2.*m_pend.*cos(THE_Psi).*cos(THE_Phi_pend).^2.*cos(THE_Psi_pend).*sin(THE_Psi_pend).*sin(THE_Theta_pend).*(2.0./3.0)+(Lz_pend.^2.*m_pend.*cos(THE_Phi_pend).*cos(THE_Psi_pend).^2.*cos(THE_Theta_pend).*sin(THE_Psi).*sin(THE_Theta_pend))./3.0-(Ly_pend.^2.*m_pend.*cos(THE_Psi).*cos(THE_Phi_pend).*cos(THE_Psi_pend).^2.*cos(THE_Theta_pend).^2.*sin(THE_Phi_pend))./1.2e+1;
et31 = (Lz_pend.^2.*m_pend.*cos(THE_Psi).*cos(THE_Phi_pend).*cos(THE_Psi_pend).^2.*cos(THE_Theta_pend).^2.*sin(THE_Phi_pend))./3.0;
et32 = I_zz+Iprop_zz.*4.0+(Ly_pend.^2.*m_pend)./1.2e+1+(Lz_pend.^2.*m_pend)./3.0+cg_to_mot_L.^2.*mprop.*4.0+I_yy.*cos(THE_Psi).^2-I_zz.*cos(THE_Psi).^2+Iprop_yy.*cos(THE_Psi).^2.*4.0-Iprop_zz.*cos(THE_Psi).^2.*4.0-I_yz.*sin(THE_Psi.*2.0)-Iprop_yz.*sin(THE_Psi.*2.0).*4.0+(Lx_pend.^2.*m_pend.*cos(THE_Psi).^2)./1.2e+1+(Lx_pend.^2.*m_pend.*cos(THE_Theta_pend).^2)./1.2e+1-(Ly_pend.^2.*m_pend.*cos(THE_Psi).^2)./1.2e+1-(Ly_pend.^2.*m_pend.*cos(THE_Theta_pend).^2)./1.2e+1+Tv_Z_pend.^2.*m_pend.*cos(THE_Psi).^2+cg_to_mot_H.^2.*mprop.*cos(THE_Psi).^2.*4.0-cg_to_mot_L.^2.*mprop.*cos(THE_Psi).^2.*2.0-(Lx_pend.^2.*m_pend.*cos(THE_Psi).^2.*cos(THE_Theta_pend).^2)./6.0+(Ly_pend.^2.*m_pend.*cos(THE_Psi).^2.*cos(THE_Phi_pend).^2)./1.2e+1;
et33 = (Ly_pend.^2.*m_pend.*cos(THE_Psi).^2.*cos(THE_Psi_pend).^2)./1.2e+1+(Ly_pend.^2.*m_pend.*cos(THE_Psi).^2.*cos(THE_Theta_pend).^2)./6.0+(Ly_pend.^2.*m_pend.*cos(THE_Psi_pend).^2.*cos(THE_Theta_pend).^2)./1.2e+1-(Lz_pend.^2.*m_pend.*cos(THE_Psi).^2.*cos(THE_Phi_pend).^2)./3.0-(Lz_pend.^2.*m_pend.*cos(THE_Psi).^2.*cos(THE_Psi_pend).^2)./3.0-(Lz_pend.^2.*m_pend.*cos(THE_Psi_pend).^2.*cos(THE_Theta_pend).^2)./3.0+(Lx_pend.^2.*m_pend.*cos(THE_Psi).^2.*cos(THE_Phi_pend).^2.*cos(THE_Theta_pend).^2)./1.2e+1-(Ly_pend.^2.*m_pend.*cos(THE_Psi).^2.*cos(THE_Phi_pend).^2.*cos(THE_Psi_pend).^2)./6.0-(Ly_pend.^2.*m_pend.*cos(THE_Psi).^2.*cos(THE_Phi_pend).^2.*cos(THE_Theta_pend).^2)./1.2e+1-(Ly_pend.^2.*m_pend.*cos(THE_Psi).^2.*cos(THE_Psi_pend).^2.*cos(THE_Theta_pend).^2)./6.0;
et34 = Lz_pend.^2.*m_pend.*cos(THE_Psi).^2.*cos(THE_Phi_pend).^2.*cos(THE_Psi_pend).^2.*(2.0./3.0)+Lz_pend.^2.*m_pend.*cos(THE_Psi).^2.*cos(THE_Psi_pend).^2.*cos(THE_Theta_pend).^2.*(2.0./3.0)+(Ly_pend.^2.*m_pend.*cos(THE_Psi).^2.*cos(THE_Phi_pend).^2.*cos(THE_Psi_pend).^2.*cos(THE_Theta_pend).^2)./1.2e+1-(Lz_pend.^2.*m_pend.*cos(THE_Psi).^2.*cos(THE_Phi_pend).^2.*cos(THE_Psi_pend).^2.*cos(THE_Theta_pend).^2)./3.0+Lz_pend.*Tv_Z_pend.*m_pend.*cos(THE_Psi).^2.*cos(THE_Psi_pend).*cos(THE_Theta_pend)-(Lx_pend.^2.*m_pend.*cos(THE_Psi).*cos(THE_Theta_pend).*sin(THE_Psi).*sin(THE_Phi_pend).*sin(THE_Theta_pend))./6.0+(Ly_pend.^2.*m_pend.*cos(THE_Psi).*cos(THE_Theta_pend).*sin(THE_Psi).*sin(THE_Phi_pend).*sin(THE_Theta_pend))./6.0-Lz_pend.*Tv_Z_pend.*m_pend.*cos(THE_Psi).*cos(THE_Phi_pend).*sin(THE_Psi).*sin(THE_Psi_pend)+Lz_pend.*Tv_Z_pend.*m_pend.*cos(THE_Psi).*cos(THE_Psi_pend).*sin(THE_Psi).*sin(THE_Phi_pend).*sin(THE_Theta_pend)-(Ly_pend.^2.*m_pend.*cos(THE_Psi).*cos(THE_Psi_pend).^2.*cos(THE_Theta_pend).*sin(THE_Psi).*sin(THE_Phi_pend).*sin(THE_Theta_pend))./6.0;
et35 = Ly_pend.^2.*m_pend.*cos(THE_Psi).^2.*cos(THE_Phi_pend).*cos(THE_Psi_pend).*sin(THE_Phi_pend).*sin(THE_Psi_pend).*sin(THE_Theta_pend).*(-1.0./6.0)+Lz_pend.^2.*m_pend.*cos(THE_Psi).*cos(THE_Psi_pend).^2.*cos(THE_Theta_pend).*sin(THE_Psi).*sin(THE_Phi_pend).*sin(THE_Theta_pend).*(2.0./3.0)+Lz_pend.^2.*m_pend.*cos(THE_Psi).^2.*cos(THE_Phi_pend).*cos(THE_Psi_pend).*sin(THE_Phi_pend).*sin(THE_Psi_pend).*sin(THE_Theta_pend).*(2.0./3.0)+(Ly_pend.^2.*m_pend.*cos(THE_Psi).*cos(THE_Phi_pend).*cos(THE_Psi_pend).*cos(THE_Theta_pend).*sin(THE_Psi).*sin(THE_Psi_pend))./6.0-Lz_pend.^2.*m_pend.*cos(THE_Psi).*cos(THE_Phi_pend).*cos(THE_Psi_pend).*cos(THE_Theta_pend).*sin(THE_Psi).*sin(THE_Psi_pend).*(2.0./3.0);
et36 = -I_yz.*cos(THE_Theta)-Iprop_yz.*cos(THE_Theta).*4.0-I_xy.*cos(THE_Psi).*sin(THE_Theta)-Iprop_xy.*cos(THE_Psi).*sin(THE_Theta).*4.0+I_xz.*sin(THE_Psi).*sin(THE_Theta)+Iprop_xz.*sin(THE_Psi).*sin(THE_Theta).*4.0+I_yz.*cos(THE_Psi).^2.*cos(THE_Theta).*2.0+Iprop_yz.*cos(THE_Psi).^2.*cos(THE_Theta).*8.0+I_yy.*cos(THE_Psi).*cos(THE_Theta).*sin(THE_Psi)-I_zz.*cos(THE_Psi).*cos(THE_Theta).*sin(THE_Psi)+Iprop_yy.*cos(THE_Psi).*cos(THE_Theta).*sin(THE_Psi).*4.0-Iprop_zz.*cos(THE_Psi).*cos(THE_Theta).*sin(THE_Psi).*4.0+(Lx_pend.^2.*m_pend.*cos(THE_Psi).*cos(THE_Theta).*sin(THE_Psi))./1.2e+1-(Ly_pend.^2.*m_pend.*cos(THE_Psi).*cos(THE_Theta).*sin(THE_Psi))./1.2e+1+Tv_Z_pend.^2.*m_pend.*cos(THE_Psi).*cos(THE_Theta).*sin(THE_Psi)+cg_to_mot_H.^2.*mprop.*cos(THE_Psi).*cos(THE_Theta).*sin(THE_Psi).*4.0-cg_to_mot_L.^2.*mprop.*cos(THE_Psi).*cos(THE_Theta).*sin(THE_Psi).*2.0-(Lx_pend.^2.*m_pend.*cos(THE_Theta).*cos(THE_Theta_pend).*sin(THE_Phi_pend).*sin(THE_Theta_pend))./1.2e+1+(Ly_pend.^2.*m_pend.*cos(THE_Psi).*cos(THE_Phi_pend).*sin(THE_Theta).*sin(THE_Phi_pend))./1.2e+1;
et37 = (Ly_pend.^2.*m_pend.*cos(THE_Theta).*cos(THE_Theta_pend).*sin(THE_Phi_pend).*sin(THE_Theta_pend))./1.2e+1-(Lz_pend.^2.*m_pend.*cos(THE_Psi).*cos(THE_Phi_pend).*sin(THE_Theta).*sin(THE_Phi_pend))./3.0-(Lz_pend.*Tv_Z_pend.*m_pend.*cos(THE_Theta).*cos(THE_Phi_pend).*sin(THE_Psi_pend))./2.0-(Lx_pend.^2.*m_pend.*cos(THE_Psi).*cos(THE_Theta).*cos(THE_Theta_pend).^2.*sin(THE_Psi))./6.0+(Ly_pend.^2.*m_pend.*cos(THE_Psi).*cos(THE_Theta).*cos(THE_Phi_pend).^2.*sin(THE_Psi))./1.2e+1+(Ly_pend.^2.*m_pend.*cos(THE_Psi).*cos(THE_Theta).*cos(THE_Psi_pend).^2.*sin(THE_Psi))./1.2e+1+(Ly_pend.^2.*m_pend.*cos(THE_Psi).*cos(THE_Theta).*cos(THE_Theta_pend).^2.*sin(THE_Psi))./6.0-(Lz_pend.^2.*m_pend.*cos(THE_Psi).*cos(THE_Theta).*cos(THE_Phi_pend).^2.*sin(THE_Psi))./3.0-(Lz_pend.^2.*m_pend.*cos(THE_Psi).*cos(THE_Theta).*cos(THE_Psi_pend).^2.*sin(THE_Psi))./3.0+(Ly_pend.^2.*m_pend.*cos(THE_Theta).*cos(THE_Phi_pend).*cos(THE_Psi_pend).*cos(THE_Theta_pend).*sin(THE_Psi_pend))./1.2e+1-(Lz_pend.^2.*m_pend.*cos(THE_Theta).*cos(THE_Phi_pend).*cos(THE_Psi_pend).*cos(THE_Theta_pend).*sin(THE_Psi_pend))./3.0;
et38 = (Lx_pend.^2.*m_pend.*cos(THE_Phi_pend).*cos(THE_Theta_pend).*sin(THE_Psi).*sin(THE_Theta).*sin(THE_Theta_pend))./1.2e+1-(Ly_pend.^2.*m_pend.*cos(THE_Psi).*cos(THE_Psi_pend).*sin(THE_Theta).*sin(THE_Psi_pend).*sin(THE_Theta_pend))./1.2e+1-(Ly_pend.^2.*m_pend.*cos(THE_Phi_pend).*cos(THE_Theta_pend).*sin(THE_Psi).*sin(THE_Theta).*sin(THE_Theta_pend))./1.2e+1+(Lz_pend.^2.*m_pend.*cos(THE_Psi).*cos(THE_Psi_pend).*sin(THE_Theta).*sin(THE_Psi_pend).*sin(THE_Theta_pend))./3.0+(Lz_pend.*Tv_Z_pend.*m_pend.*cos(THE_Theta).*cos(THE_Psi_pend).*sin(THE_Phi_pend).*sin(THE_Theta_pend))./2.0-(Lz_pend.*Tv_Z_pend.*m_pend.*sin(THE_Psi).*sin(THE_Theta).*sin(THE_Phi_pend).*sin(THE_Psi_pend))./2.0+(Lx_pend.^2.*m_pend.*cos(THE_Psi).*cos(THE_Phi_pend).*cos(THE_Theta_pend).^2.*sin(THE_Theta).*sin(THE_Phi_pend))./1.2e+1+(Lx_pend.^2.*m_pend.*cos(THE_Psi).^2.*cos(THE_Theta).*cos(THE_Theta_pend).*sin(THE_Phi_pend).*sin(THE_Theta_pend))./6.0-(Ly_pend.^2.*m_pend.*cos(THE_Psi).*cos(THE_Phi_pend).*cos(THE_Psi_pend).^2.*sin(THE_Theta).*sin(THE_Phi_pend))./6.0-(Ly_pend.^2.*m_pend.*cos(THE_Psi).*cos(THE_Phi_pend).*cos(THE_Theta_pend).^2.*sin(THE_Theta).*sin(THE_Phi_pend))./1.2e+1;
et39 = Ly_pend.^2.*m_pend.*cos(THE_Psi).^2.*cos(THE_Theta).*cos(THE_Theta_pend).*sin(THE_Phi_pend).*sin(THE_Theta_pend).*(-1.0./6.0)-(Ly_pend.^2.*m_pend.*cos(THE_Theta).*cos(THE_Psi_pend).^2.*cos(THE_Theta_pend).*sin(THE_Phi_pend).*sin(THE_Theta_pend))./1.2e+1+Lz_pend.^2.*m_pend.*cos(THE_Psi).*cos(THE_Phi_pend).*cos(THE_Psi_pend).^2.*sin(THE_Theta).*sin(THE_Phi_pend).*(2.0./3.0)+(Lz_pend.^2.*m_pend.*cos(THE_Theta).*cos(THE_Psi_pend).^2.*cos(THE_Theta_pend).*sin(THE_Phi_pend).*sin(THE_Theta_pend))./3.0+Lz_pend.*Tv_Z_pend.*m_pend.*cos(THE_Psi).^2.*cos(THE_Theta).*cos(THE_Phi_pend).*sin(THE_Psi_pend)+(Lx_pend.^2.*m_pend.*cos(THE_Psi).*cos(THE_Theta).*cos(THE_Phi_pend).^2.*cos(THE_Theta_pend).^2.*sin(THE_Psi))./1.2e+1-(Ly_pend.^2.*m_pend.*cos(THE_Psi).*cos(THE_Theta).*cos(THE_Phi_pend).^2.*cos(THE_Psi_pend).^2.*sin(THE_Psi))./6.0-(Ly_pend.^2.*m_pend.*cos(THE_Psi).*cos(THE_Theta).*cos(THE_Phi_pend).^2.*cos(THE_Theta_pend).^2.*sin(THE_Psi))./1.2e+1-(Ly_pend.^2.*m_pend.*cos(THE_Psi).*cos(THE_Theta).*cos(THE_Psi_pend).^2.*cos(THE_Theta_pend).^2.*sin(THE_Psi))./6.0;
et40 = Lz_pend.^2.*m_pend.*cos(THE_Psi).*cos(THE_Theta).*cos(THE_Phi_pend).^2.*cos(THE_Psi_pend).^2.*sin(THE_Psi).*(2.0./3.0)+Lz_pend.^2.*m_pend.*cos(THE_Psi).*cos(THE_Theta).*cos(THE_Psi_pend).^2.*cos(THE_Theta_pend).^2.*sin(THE_Psi).*(2.0./3.0)+(Ly_pend.^2.*m_pend.*cos(THE_Psi_pend).*cos(THE_Theta_pend).*sin(THE_Psi).*sin(THE_Theta).*sin(THE_Phi_pend).*sin(THE_Psi_pend))./1.2e+1-(Lz_pend.^2.*m_pend.*cos(THE_Psi_pend).*cos(THE_Theta_pend).*sin(THE_Psi).*sin(THE_Theta).*sin(THE_Phi_pend).*sin(THE_Psi_pend))./3.0+Lz_pend.*Tv_Z_pend.*m_pend.*cos(THE_Psi).*cos(THE_Theta).*cos(THE_Psi_pend).*cos(THE_Theta_pend).*sin(THE_Psi)-(Lz_pend.*Tv_Z_pend.*m_pend.*cos(THE_Phi_pend).*cos(THE_Psi_pend).*sin(THE_Psi).*sin(THE_Theta).*sin(THE_Theta_pend))./2.0-(Ly_pend.^2.*m_pend.*cos(THE_Psi).^2.*cos(THE_Theta).*cos(THE_Phi_pend).*cos(THE_Psi_pend).*cos(THE_Theta_pend).*sin(THE_Psi_pend))./6.0+Lz_pend.^2.*m_pend.*cos(THE_Psi).^2.*cos(THE_Theta).*cos(THE_Phi_pend).*cos(THE_Psi_pend).*cos(THE_Theta_pend).*sin(THE_Psi_pend).*(2.0./3.0)+(Ly_pend.^2.*m_pend.*cos(THE_Psi).*cos(THE_Phi_pend).^2.*cos(THE_Psi_pend).*sin(THE_Theta).*sin(THE_Psi_pend).*sin(THE_Theta_pend))./6.0;
et41 = (Ly_pend.^2.*m_pend.*cos(THE_Phi_pend).*cos(THE_Psi_pend).^2.*cos(THE_Theta_pend).*sin(THE_Psi).*sin(THE_Theta).*sin(THE_Theta_pend))./1.2e+1-Lz_pend.^2.*m_pend.*cos(THE_Psi).*cos(THE_Phi_pend).^2.*cos(THE_Psi_pend).*sin(THE_Theta).*sin(THE_Psi_pend).*sin(THE_Theta_pend).*(2.0./3.0)-(Lz_pend.^2.*m_pend.*cos(THE_Phi_pend).*cos(THE_Psi_pend).^2.*cos(THE_Theta_pend).*sin(THE_Psi).*sin(THE_Theta).*sin(THE_Theta_pend))./3.0-Lz_pend.*Tv_Z_pend.*m_pend.*cos(THE_Psi).^2.*cos(THE_Theta).*cos(THE_Psi_pend).*sin(THE_Phi_pend).*sin(THE_Theta_pend)+(Ly_pend.^2.*m_pend.*cos(THE_Psi).*cos(THE_Phi_pend).*cos(THE_Psi_pend).^2.*cos(THE_Theta_pend).^2.*sin(THE_Theta).*sin(THE_Phi_pend))./1.2e+1+(Ly_pend.^2.*m_pend.*cos(THE_Psi).^2.*cos(THE_Theta).*cos(THE_Psi_pend).^2.*cos(THE_Theta_pend).*sin(THE_Phi_pend).*sin(THE_Theta_pend))./6.0-(Lz_pend.^2.*m_pend.*cos(THE_Psi).*cos(THE_Phi_pend).*cos(THE_Psi_pend).^2.*cos(THE_Theta_pend).^2.*sin(THE_Theta).*sin(THE_Phi_pend))./3.0-Lz_pend.^2.*m_pend.*cos(THE_Psi).^2.*cos(THE_Theta).*cos(THE_Psi_pend).^2.*cos(THE_Theta_pend).*sin(THE_Phi_pend).*sin(THE_Theta_pend).*(2.0./3.0);
et42 = (Ly_pend.^2.*m_pend.*cos(THE_Psi).*cos(THE_Theta).*cos(THE_Phi_pend).^2.*cos(THE_Psi_pend).^2.*cos(THE_Theta_pend).^2.*sin(THE_Psi))./1.2e+1-(Lz_pend.^2.*m_pend.*cos(THE_Psi).*cos(THE_Theta).*cos(THE_Phi_pend).^2.*cos(THE_Psi_pend).^2.*cos(THE_Theta_pend).^2.*sin(THE_Psi))./3.0-(Ly_pend.^2.*m_pend.*cos(THE_Psi).*cos(THE_Theta).*cos(THE_Phi_pend).*cos(THE_Psi_pend).*sin(THE_Psi).*sin(THE_Phi_pend).*sin(THE_Psi_pend).*sin(THE_Theta_pend))./6.0+Lz_pend.^2.*m_pend.*cos(THE_Psi).*cos(THE_Theta).*cos(THE_Phi_pend).*cos(THE_Psi_pend).*sin(THE_Psi).*sin(THE_Phi_pend).*sin(THE_Psi_pend).*sin(THE_Theta_pend).*(2.0./3.0);
et43 = I_xx+Iprop_xx.*4.0+(Lx_pend.^2.*m_pend)./1.2e+1+(Ly_pend.^2.*m_pend)./1.2e+1+Tv_Z_pend.^2.*m_pend+cg_to_mot_H.^2.*mprop.*4.0+cg_to_mot_L.^2.*mprop.*2.0-(Ly_pend.^2.*m_pend.*cos(THE_Phi_pend).^2)./1.2e+1-(Ly_pend.^2.*m_pend.*cos(THE_Psi_pend).^2)./1.2e+1+(Lz_pend.^2.*m_pend.*cos(THE_Phi_pend).^2)./3.0+(Lz_pend.^2.*m_pend.*cos(THE_Psi_pend).^2)./3.0-(Lx_pend.^2.*m_pend.*cos(THE_Phi_pend).^2.*cos(THE_Theta_pend).^2)./1.2e+1+(Ly_pend.^2.*m_pend.*cos(THE_Phi_pend).^2.*cos(THE_Psi_pend).^2)./6.0+(Ly_pend.^2.*m_pend.*cos(THE_Phi_pend).^2.*cos(THE_Theta_pend).^2)./1.2e+1-Lz_pend.^2.*m_pend.*cos(THE_Phi_pend).^2.*cos(THE_Psi_pend).^2.*(2.0./3.0)-(Ly_pend.^2.*m_pend.*cos(THE_Phi_pend).^2.*cos(THE_Psi_pend).^2.*cos(THE_Theta_pend).^2)./1.2e+1;
et44 = (Lz_pend.^2.*m_pend.*cos(THE_Phi_pend).^2.*cos(THE_Psi_pend).^2.*cos(THE_Theta_pend).^2)./3.0+Lz_pend.*Tv_Z_pend.*m_pend.*cos(THE_Psi_pend).*cos(THE_Theta_pend)+(Ly_pend.^2.*m_pend.*cos(THE_Phi_pend).*cos(THE_Psi_pend).*sin(THE_Phi_pend).*sin(THE_Psi_pend).*sin(THE_Theta_pend))./6.0-Lz_pend.^2.*m_pend.*cos(THE_Phi_pend).*cos(THE_Psi_pend).*sin(THE_Phi_pend).*sin(THE_Psi_pend).*sin(THE_Theta_pend).*(2.0./3.0);
et45 = I_xy.*cos(THE_Psi)+Iprop_xy.*cos(THE_Psi).*4.0-I_xz.*sin(THE_Psi)-Iprop_xz.*sin(THE_Psi).*4.0-(Ly_pend.^2.*m_pend.*cos(THE_Psi).*cos(THE_Phi_pend).*sin(THE_Phi_pend))./1.2e+1+(Lz_pend.^2.*m_pend.*cos(THE_Psi).*cos(THE_Phi_pend).*sin(THE_Phi_pend))./3.0-(Lx_pend.^2.*m_pend.*cos(THE_Phi_pend).*cos(THE_Theta_pend).*sin(THE_Psi).*sin(THE_Theta_pend))./1.2e+1+(Ly_pend.^2.*m_pend.*cos(THE_Psi).*cos(THE_Psi_pend).*sin(THE_Psi_pend).*sin(THE_Theta_pend))./1.2e+1+(Ly_pend.^2.*m_pend.*cos(THE_Phi_pend).*cos(THE_Theta_pend).*sin(THE_Psi).*sin(THE_Theta_pend))./1.2e+1-(Lz_pend.^2.*m_pend.*cos(THE_Psi).*cos(THE_Psi_pend).*sin(THE_Psi_pend).*sin(THE_Theta_pend))./3.0+(Lz_pend.*Tv_Z_pend.*m_pend.*sin(THE_Psi).*sin(THE_Phi_pend).*sin(THE_Psi_pend))./2.0-(Lx_pend.^2.*m_pend.*cos(THE_Psi).*cos(THE_Phi_pend).*cos(THE_Theta_pend).^2.*sin(THE_Phi_pend))./1.2e+1+(Ly_pend.^2.*m_pend.*cos(THE_Psi).*cos(THE_Phi_pend).*cos(THE_Psi_pend).^2.*sin(THE_Phi_pend))./6.0+(Ly_pend.^2.*m_pend.*cos(THE_Psi).*cos(THE_Phi_pend).*cos(THE_Theta_pend).^2.*sin(THE_Phi_pend))./1.2e+1;
et46 = Lz_pend.^2.*m_pend.*cos(THE_Psi).*cos(THE_Phi_pend).*cos(THE_Psi_pend).^2.*sin(THE_Phi_pend).*(-2.0./3.0)-(Ly_pend.^2.*m_pend.*cos(THE_Psi_pend).*cos(THE_Theta_pend).*sin(THE_Psi).*sin(THE_Phi_pend).*sin(THE_Psi_pend))./1.2e+1+(Lz_pend.^2.*m_pend.*cos(THE_Psi_pend).*cos(THE_Theta_pend).*sin(THE_Psi).*sin(THE_Phi_pend).*sin(THE_Psi_pend))./3.0+(Lz_pend.*Tv_Z_pend.*m_pend.*cos(THE_Phi_pend).*cos(THE_Psi_pend).*sin(THE_Psi).*sin(THE_Theta_pend))./2.0-(Ly_pend.^2.*m_pend.*cos(THE_Psi).*cos(THE_Phi_pend).^2.*cos(THE_Psi_pend).*sin(THE_Psi_pend).*sin(THE_Theta_pend))./6.0-(Ly_pend.^2.*m_pend.*cos(THE_Phi_pend).*cos(THE_Psi_pend).^2.*cos(THE_Theta_pend).*sin(THE_Psi).*sin(THE_Theta_pend))./1.2e+1+Lz_pend.^2.*m_pend.*cos(THE_Psi).*cos(THE_Phi_pend).^2.*cos(THE_Psi_pend).*sin(THE_Psi_pend).*sin(THE_Theta_pend).*(2.0./3.0)+(Lz_pend.^2.*m_pend.*cos(THE_Phi_pend).*cos(THE_Psi_pend).^2.*cos(THE_Theta_pend).*sin(THE_Psi).*sin(THE_Theta_pend))./3.0-(Ly_pend.^2.*m_pend.*cos(THE_Psi).*cos(THE_Phi_pend).*cos(THE_Psi_pend).^2.*cos(THE_Theta_pend).^2.*sin(THE_Phi_pend))./1.2e+1;
et47 = (Lz_pend.^2.*m_pend.*cos(THE_Psi).*cos(THE_Phi_pend).*cos(THE_Psi_pend).^2.*cos(THE_Theta_pend).^2.*sin(THE_Phi_pend))./3.0;
et48 = -I_xx.*sin(THE_Theta)-Iprop_xx.*sin(THE_Theta).*4.0+I_xz.*cos(THE_Psi).*cos(THE_Theta)+Iprop_xz.*cos(THE_Psi).*cos(THE_Theta).*4.0+I_xy.*cos(THE_Theta).*sin(THE_Psi)+Iprop_xy.*cos(THE_Theta).*sin(THE_Psi).*4.0-(Lx_pend.^2.*m_pend.*sin(THE_Theta))./1.2e+1-(Ly_pend.^2.*m_pend.*sin(THE_Theta))./1.2e+1-Tv_Z_pend.^2.*m_pend.*sin(THE_Theta)-cg_to_mot_H.^2.*mprop.*sin(THE_Theta).*4.0-cg_to_mot_L.^2.*mprop.*sin(THE_Theta).*2.0+(Ly_pend.^2.*m_pend.*cos(THE_Phi_pend).^2.*sin(THE_Theta))./1.2e+1+(Ly_pend.^2.*m_pend.*cos(THE_Psi_pend).^2.*sin(THE_Theta))./1.2e+1-(Lz_pend.^2.*m_pend.*cos(THE_Phi_pend).^2.*sin(THE_Theta))./3.0-(Lz_pend.^2.*m_pend.*cos(THE_Psi_pend).^2.*sin(THE_Theta))./3.0+(Lx_pend.^2.*m_pend.*cos(THE_Phi_pend).^2.*cos(THE_Theta_pend).^2.*sin(THE_Theta))./1.2e+1-(Ly_pend.^2.*m_pend.*cos(THE_Phi_pend).^2.*cos(THE_Psi_pend).^2.*sin(THE_Theta))./6.0;
et49 = Ly_pend.^2.*m_pend.*cos(THE_Phi_pend).^2.*cos(THE_Theta_pend).^2.*sin(THE_Theta).*(-1.0./1.2e+1)+Lz_pend.^2.*m_pend.*cos(THE_Phi_pend).^2.*cos(THE_Psi_pend).^2.*sin(THE_Theta).*(2.0./3.0)-(Ly_pend.^2.*m_pend.*cos(THE_Theta).*cos(THE_Phi_pend).*sin(THE_Psi).*sin(THE_Phi_pend))./1.2e+1+(Lz_pend.^2.*m_pend.*cos(THE_Theta).*cos(THE_Phi_pend).*sin(THE_Psi).*sin(THE_Phi_pend))./3.0+(Ly_pend.^2.*m_pend.*cos(THE_Phi_pend).^2.*cos(THE_Psi_pend).^2.*cos(THE_Theta_pend).^2.*sin(THE_Theta))./1.2e+1-(Lz_pend.^2.*m_pend.*cos(THE_Phi_pend).^2.*cos(THE_Psi_pend).^2.*cos(THE_Theta_pend).^2.*sin(THE_Theta))./3.0-Lz_pend.*Tv_Z_pend.*m_pend.*cos(THE_Psi_pend).*cos(THE_Theta_pend).*sin(THE_Theta)+(Lx_pend.^2.*m_pend.*cos(THE_Psi).*cos(THE_Theta).*cos(THE_Phi_pend).*cos(THE_Theta_pend).*sin(THE_Theta_pend))./1.2e+1-(Ly_pend.^2.*m_pend.*cos(THE_Psi).*cos(THE_Theta).*cos(THE_Phi_pend).*cos(THE_Theta_pend).*sin(THE_Theta_pend))./1.2e+1+(Ly_pend.^2.*m_pend.*cos(THE_Theta).*cos(THE_Psi_pend).*sin(THE_Psi).*sin(THE_Psi_pend).*sin(THE_Theta_pend))./1.2e+1;
et50 = Lz_pend.^2.*m_pend.*cos(THE_Theta).*cos(THE_Psi_pend).*sin(THE_Psi).*sin(THE_Psi_pend).*sin(THE_Theta_pend).*(-1.0./3.0)-(Lz_pend.*Tv_Z_pend.*m_pend.*cos(THE_Psi).*cos(THE_Theta).*sin(THE_Phi_pend).*sin(THE_Psi_pend))./2.0-(Lx_pend.^2.*m_pend.*cos(THE_Theta).*cos(THE_Phi_pend).*cos(THE_Theta_pend).^2.*sin(THE_Psi).*sin(THE_Phi_pend))./1.2e+1+(Ly_pend.^2.*m_pend.*cos(THE_Theta).*cos(THE_Phi_pend).*cos(THE_Psi_pend).^2.*sin(THE_Psi).*sin(THE_Phi_pend))./6.0+(Ly_pend.^2.*m_pend.*cos(THE_Theta).*cos(THE_Phi_pend).*cos(THE_Theta_pend).^2.*sin(THE_Psi).*sin(THE_Phi_pend))./1.2e+1-Lz_pend.^2.*m_pend.*cos(THE_Theta).*cos(THE_Phi_pend).*cos(THE_Psi_pend).^2.*sin(THE_Psi).*sin(THE_Phi_pend).*(2.0./3.0)-(Ly_pend.^2.*m_pend.*cos(THE_Phi_pend).*cos(THE_Psi_pend).*sin(THE_Theta).*sin(THE_Phi_pend).*sin(THE_Psi_pend).*sin(THE_Theta_pend))./6.0+Lz_pend.^2.*m_pend.*cos(THE_Phi_pend).*cos(THE_Psi_pend).*sin(THE_Theta).*sin(THE_Phi_pend).*sin(THE_Psi_pend).*sin(THE_Theta_pend).*(2.0./3.0)-(Lz_pend.*Tv_Z_pend.*m_pend.*cos(THE_Psi).*cos(THE_Theta).*cos(THE_Phi_pend).*cos(THE_Psi_pend).*sin(THE_Theta_pend))./2.0;
et51 = (Ly_pend.^2.*m_pend.*cos(THE_Psi).*cos(THE_Theta).*cos(THE_Phi_pend).*cos(THE_Psi_pend).^2.*cos(THE_Theta_pend).*sin(THE_Theta_pend))./1.2e+1-(Lz_pend.^2.*m_pend.*cos(THE_Psi).*cos(THE_Theta).*cos(THE_Phi_pend).*cos(THE_Psi_pend).^2.*cos(THE_Theta_pend).*sin(THE_Theta_pend))./3.0-(Ly_pend.^2.*m_pend.*cos(THE_Theta).*cos(THE_Phi_pend).^2.*cos(THE_Psi_pend).*sin(THE_Psi).*sin(THE_Psi_pend).*sin(THE_Theta_pend))./6.0+Lz_pend.^2.*m_pend.*cos(THE_Theta).*cos(THE_Phi_pend).^2.*cos(THE_Psi_pend).*sin(THE_Psi).*sin(THE_Psi_pend).*sin(THE_Theta_pend).*(2.0./3.0)-(Ly_pend.^2.*m_pend.*cos(THE_Theta).*cos(THE_Phi_pend).*cos(THE_Psi_pend).^2.*cos(THE_Theta_pend).^2.*sin(THE_Psi).*sin(THE_Phi_pend))./1.2e+1+(Lz_pend.^2.*m_pend.*cos(THE_Theta).*cos(THE_Phi_pend).*cos(THE_Psi_pend).^2.*cos(THE_Theta_pend).^2.*sin(THE_Psi).*sin(THE_Phi_pend))./3.0+(Ly_pend.^2.*m_pend.*cos(THE_Psi).*cos(THE_Theta).*cos(THE_Psi_pend).*cos(THE_Theta_pend).*sin(THE_Phi_pend).*sin(THE_Psi_pend))./1.2e+1-(Lz_pend.^2.*m_pend.*cos(THE_Psi).*cos(THE_Theta).*cos(THE_Psi_pend).*cos(THE_Theta_pend).*sin(THE_Phi_pend).*sin(THE_Psi_pend))./3.0;
et52 = Ly_pend.^2.*m_pend.*sin(THE_Psi).*(-1.0./1.2e+1)-(Lz_pend.^2.*m_pend.*sin(THE_Psi))./3.0-(Lx_pend.^2.*m_pend.*cos(THE_Theta_pend).^2.*sin(THE_Psi))./1.2e+1+(Ly_pend.^2.*m_pend.*cos(THE_Theta_pend).^2.*sin(THE_Psi))./1.2e+1-(Ly_pend.^2.*m_pend.*cos(THE_Psi_pend).^2.*cos(THE_Theta_pend).^2.*sin(THE_Psi))./1.2e+1+(Lz_pend.^2.*m_pend.*cos(THE_Psi_pend).^2.*cos(THE_Theta_pend).^2.*sin(THE_Psi))./3.0+(Lx_pend.^2.*m_pend.*cos(THE_Psi).*cos(THE_Theta_pend).*sin(THE_Phi_pend).*sin(THE_Theta_pend))./1.2e+1-(Ly_pend.^2.*m_pend.*cos(THE_Psi).*cos(THE_Theta_pend).*sin(THE_Phi_pend).*sin(THE_Theta_pend))./1.2e+1+(Lz_pend.*Tv_Z_pend.*m_pend.*cos(THE_Psi).*cos(THE_Phi_pend).*sin(THE_Psi_pend))./2.0-(Ly_pend.^2.*m_pend.*cos(THE_Psi).*cos(THE_Phi_pend).*cos(THE_Psi_pend).*cos(THE_Theta_pend).*sin(THE_Psi_pend))./1.2e+1+(Lz_pend.^2.*m_pend.*cos(THE_Psi).*cos(THE_Phi_pend).*cos(THE_Psi_pend).*cos(THE_Theta_pend).*sin(THE_Psi_pend))./3.0-(Lz_pend.*Tv_Z_pend.*m_pend.*cos(THE_Psi).*cos(THE_Psi_pend).*sin(THE_Phi_pend).*sin(THE_Theta_pend))./2.0;
et53 = (Ly_pend.^2.*m_pend.*cos(THE_Psi).*cos(THE_Psi_pend).^2.*cos(THE_Theta_pend).*sin(THE_Phi_pend).*sin(THE_Theta_pend))./1.2e+1-(Lz_pend.^2.*m_pend.*cos(THE_Psi).*cos(THE_Psi_pend).^2.*cos(THE_Theta_pend).*sin(THE_Phi_pend).*sin(THE_Theta_pend))./3.0;
et54 = (Ly_pend.^2.*m_pend.*cos(THE_Psi).*cos(THE_Theta))./1.2e+1+(Lz_pend.^2.*m_pend.*cos(THE_Psi).*cos(THE_Theta))./3.0+(Lx_pend.^2.*m_pend.*cos(THE_Psi).*cos(THE_Theta).*cos(THE_Theta_pend).^2)./1.2e+1-(Ly_pend.^2.*m_pend.*cos(THE_Psi).*cos(THE_Theta).*cos(THE_Theta_pend).^2)./1.2e+1+(Ly_pend.^2.*m_pend.*cos(THE_Psi).*cos(THE_Theta).*cos(THE_Psi_pend).^2.*cos(THE_Theta_pend).^2)./1.2e+1-(Lz_pend.^2.*m_pend.*cos(THE_Psi).*cos(THE_Theta).*cos(THE_Psi_pend).^2.*cos(THE_Theta_pend).^2)./3.0-(Lx_pend.^2.*m_pend.*cos(THE_Phi_pend).*cos(THE_Theta_pend).*sin(THE_Theta).*sin(THE_Theta_pend))./1.2e+1+(Ly_pend.^2.*m_pend.*cos(THE_Phi_pend).*cos(THE_Theta_pend).*sin(THE_Theta).*sin(THE_Theta_pend))./1.2e+1+(Lz_pend.*Tv_Z_pend.*m_pend.*sin(THE_Theta).*sin(THE_Phi_pend).*sin(THE_Psi_pend))./2.0+(Lx_pend.^2.*m_pend.*cos(THE_Theta).*cos(THE_Theta_pend).*sin(THE_Psi).*sin(THE_Phi_pend).*sin(THE_Theta_pend))./1.2e+1-(Ly_pend.^2.*m_pend.*cos(THE_Theta).*cos(THE_Theta_pend).*sin(THE_Psi).*sin(THE_Phi_pend).*sin(THE_Theta_pend))./1.2e+1;
et55 = Ly_pend.^2.*m_pend.*cos(THE_Psi_pend).*cos(THE_Theta_pend).*sin(THE_Theta).*sin(THE_Phi_pend).*sin(THE_Psi_pend).*(-1.0./1.2e+1)+(Lz_pend.^2.*m_pend.*cos(THE_Psi_pend).*cos(THE_Theta_pend).*sin(THE_Theta).*sin(THE_Phi_pend).*sin(THE_Psi_pend))./3.0+(Lz_pend.*Tv_Z_pend.*m_pend.*cos(THE_Theta).*cos(THE_Phi_pend).*sin(THE_Psi).*sin(THE_Psi_pend))./2.0+(Lz_pend.*Tv_Z_pend.*m_pend.*cos(THE_Phi_pend).*cos(THE_Psi_pend).*sin(THE_Theta).*sin(THE_Theta_pend))./2.0-(Ly_pend.^2.*m_pend.*cos(THE_Phi_pend).*cos(THE_Psi_pend).^2.*cos(THE_Theta_pend).*sin(THE_Theta).*sin(THE_Theta_pend))./1.2e+1+(Lz_pend.^2.*m_pend.*cos(THE_Phi_pend).*cos(THE_Psi_pend).^2.*cos(THE_Theta_pend).*sin(THE_Theta).*sin(THE_Theta_pend))./3.0-(Lz_pend.*Tv_Z_pend.*m_pend.*cos(THE_Theta).*cos(THE_Psi_pend).*sin(THE_Psi).*sin(THE_Phi_pend).*sin(THE_Theta_pend))./2.0+(Ly_pend.^2.*m_pend.*cos(THE_Theta).*cos(THE_Psi_pend).^2.*cos(THE_Theta_pend).*sin(THE_Psi).*sin(THE_Phi_pend).*sin(THE_Theta_pend))./1.2e+1-(Lz_pend.^2.*m_pend.*cos(THE_Theta).*cos(THE_Psi_pend).^2.*cos(THE_Theta_pend).*sin(THE_Psi).*sin(THE_Phi_pend).*sin(THE_Theta_pend))./3.0-(Ly_pend.^2.*m_pend.*cos(THE_Theta).*cos(THE_Phi_pend).*cos(THE_Psi_pend).*cos(THE_Theta_pend).*sin(THE_Psi).*sin(THE_Psi_pend))./1.2e+1;
et56 = (Lz_pend.^2.*m_pend.*cos(THE_Theta).*cos(THE_Phi_pend).*cos(THE_Psi_pend).*cos(THE_Theta_pend).*sin(THE_Psi).*sin(THE_Psi_pend))./3.0;
et57 = (Lx_pend.^2.*m_pend.*sin(THE_Theta).*sin(THE_Phi_pend))./1.2e+1+(Ly_pend.^2.*m_pend.*sin(THE_Theta).*sin(THE_Phi_pend))./1.2e+1-(Ly_pend.^2.*m_pend.*cos(THE_Psi_pend).^2.*sin(THE_Theta).*sin(THE_Phi_pend))./1.2e+1+(Lz_pend.^2.*m_pend.*cos(THE_Psi_pend).^2.*sin(THE_Theta).*sin(THE_Phi_pend))./3.0+(Lx_pend.^2.*m_pend.*cos(THE_Theta).*cos(THE_Phi_pend).*sin(THE_Psi))./1.2e+1+(Ly_pend.^2.*m_pend.*cos(THE_Theta).*cos(THE_Phi_pend).*sin(THE_Psi))./1.2e+1-(Ly_pend.^2.*m_pend.*cos(THE_Theta).*cos(THE_Phi_pend).*cos(THE_Psi_pend).^2.*sin(THE_Psi))./1.2e+1+(Lz_pend.^2.*m_pend.*cos(THE_Theta).*cos(THE_Phi_pend).*cos(THE_Psi_pend).^2.*sin(THE_Psi))./3.0-(Ly_pend.^2.*m_pend.*cos(THE_Psi).*cos(THE_Theta).*cos(THE_Psi_pend).*cos(THE_Theta_pend).*sin(THE_Psi_pend))./1.2e+1+(Lz_pend.^2.*m_pend.*cos(THE_Psi).*cos(THE_Theta).*cos(THE_Psi_pend).*cos(THE_Theta_pend).*sin(THE_Psi_pend))./3.0+(Ly_pend.^2.*m_pend.*cos(THE_Phi_pend).*cos(THE_Psi_pend).*sin(THE_Theta).*sin(THE_Psi_pend).*sin(THE_Theta_pend))./1.2e+1;
et58 = Lz_pend.^2.*m_pend.*cos(THE_Phi_pend).*cos(THE_Psi_pend).*sin(THE_Theta).*sin(THE_Psi_pend).*sin(THE_Theta_pend).*(-1.0./3.0)+(Lz_pend.*Tv_Z_pend.*m_pend.*cos(THE_Psi_pend).*cos(THE_Theta_pend).*sin(THE_Theta).*sin(THE_Phi_pend))./2.0-(Ly_pend.^2.*m_pend.*cos(THE_Theta).*cos(THE_Psi_pend).*sin(THE_Psi).*sin(THE_Phi_pend).*sin(THE_Psi_pend).*sin(THE_Theta_pend))./1.2e+1+(Lz_pend.^2.*m_pend.*cos(THE_Theta).*cos(THE_Psi_pend).*sin(THE_Psi).*sin(THE_Phi_pend).*sin(THE_Psi_pend).*sin(THE_Theta_pend))./3.0+(Lz_pend.*Tv_Z_pend.*m_pend.*cos(THE_Theta).*cos(THE_Phi_pend).*cos(THE_Psi_pend).*cos(THE_Theta_pend).*sin(THE_Psi))./2.0;
mt1 = [et17+et18+et19+et20+et21+et22+et23+et24+et25+et26,et10+et11+et12+et13+et14+et15+et16,et6+et7+et8+et9,Tv_Z_pend.*m_pend.*cos(THE_Phi).*sin(THE_Psi)+cg_to_mot_H.*mprop.*cos(THE_Phi).*sin(THE_Psi).*4.0-Tv_Z_pend.*m_pend.*cos(THE_Psi).*sin(THE_Phi).*sin(THE_Theta)-cg_to_mot_H.*mprop.*cos(THE_Psi).*sin(THE_Phi).*sin(THE_Theta).*4.0+(Lz_pend.*m_pend.*cos(THE_Phi).*cos(THE_Psi).*cos(THE_Phi_pend).*sin(THE_Psi_pend))./2.0+(Lz_pend.*m_pend.*cos(THE_Phi).*cos(THE_Psi_pend).*cos(THE_Theta_pend).*sin(THE_Psi))./2.0-(Lz_pend.*m_pend.*cos(THE_Theta).*sin(THE_Phi).*sin(THE_Phi_pend).*sin(THE_Psi_pend))./2.0-(Lz_pend.*m_pend.*cos(THE_Psi).*cos(THE_Psi_pend).*cos(THE_Theta_pend).*sin(THE_Phi).*sin(THE_Theta))./2.0-(Lz_pend.*m_pend.*cos(THE_Phi).*cos(THE_Psi).*cos(THE_Psi_pend).*sin(THE_Phi_pend).*sin(THE_Theta_pend))./2.0-(Lz_pend.*m_pend.*cos(THE_Theta).*cos(THE_Phi_pend).*cos(THE_Psi_pend).*sin(THE_Phi).*sin(THE_Theta_pend))./2.0+(Lz_pend.*m_pend.*cos(THE_Phi_pend).*sin(THE_Phi).*sin(THE_Psi).*sin(THE_Theta).*sin(THE_Psi_pend))./2.0-(Lz_pend.*m_pend.*cos(THE_Psi_pend).*sin(THE_Phi).*sin(THE_Psi).*sin(THE_Theta).*sin(THE_Phi_pend).*sin(THE_Theta_pend))./2.0];
mt2 = [Tv_Z_pend.*m_pend.*sin(THE_Phi).*sin(THE_Psi)+cg_to_mot_H.*mprop.*sin(THE_Phi).*sin(THE_Psi).*4.0+Tv_Z_pend.*m_pend.*cos(THE_Phi).*cos(THE_Psi).*sin(THE_Theta)+cg_to_mot_H.*mprop.*cos(THE_Phi).*cos(THE_Psi).*sin(THE_Theta).*4.0+(Lz_pend.*m_pend.*cos(THE_Psi).*cos(THE_Phi_pend).*sin(THE_Phi).*sin(THE_Psi_pend))./2.0+(Lz_pend.*m_pend.*cos(THE_Phi).*cos(THE_Theta).*sin(THE_Phi_pend).*sin(THE_Psi_pend))./2.0+(Lz_pend.*m_pend.*cos(THE_Psi_pend).*cos(THE_Theta_pend).*sin(THE_Phi).*sin(THE_Psi))./2.0+(Lz_pend.*m_pend.*cos(THE_Phi).*cos(THE_Psi).*cos(THE_Psi_pend).*cos(THE_Theta_pend).*sin(THE_Theta))./2.0+(Lz_pend.*m_pend.*cos(THE_Phi).*cos(THE_Theta).*cos(THE_Phi_pend).*cos(THE_Psi_pend).*sin(THE_Theta_pend))./2.0-(Lz_pend.*m_pend.*cos(THE_Phi).*cos(THE_Phi_pend).*sin(THE_Psi).*sin(THE_Theta).*sin(THE_Psi_pend))./2.0-(Lz_pend.*m_pend.*cos(THE_Psi).*cos(THE_Psi_pend).*sin(THE_Phi).*sin(THE_Phi_pend).*sin(THE_Theta_pend))./2.0+(Lz_pend.*m_pend.*cos(THE_Phi).*cos(THE_Psi_pend).*sin(THE_Psi).*sin(THE_Theta).*sin(THE_Phi_pend).*sin(THE_Theta_pend))./2.0,0.0,et3+et4+et5,et1+et2];
mt3 = [Ly_pend.^2.*m_pend.*cos(THE_Psi).*cos(THE_Theta).*sin(THE_Theta_pend).*(-1.0./1.2e+1)-(Ly_pend.^2.*m_pend.*cos(THE_Phi_pend).*cos(THE_Theta_pend).*sin(THE_Theta))./1.2e+1-(Lz_pend.^2.*m_pend.*cos(THE_Psi).*cos(THE_Theta).*sin(THE_Theta_pend))./3.0-(Lz_pend.^2.*m_pend.*cos(THE_Phi_pend).*cos(THE_Theta_pend).*sin(THE_Theta))./3.0+(Ly_pend.^2.*m_pend.*cos(THE_Theta).*cos(THE_Theta_pend).*sin(THE_Psi).*sin(THE_Phi_pend))./1.2e+1+(Lz_pend.^2.*m_pend.*cos(THE_Theta).*cos(THE_Theta_pend).*sin(THE_Psi).*sin(THE_Phi_pend))./3.0-(Lz_pend.*Tv_Z_pend.*m_pend.*cos(THE_Phi_pend).*cos(THE_Psi_pend).*sin(THE_Theta))./2.0+(Lz_pend.*Tv_Z_pend.*m_pend.*cos(THE_Theta).*cos(THE_Psi_pend).*sin(THE_Psi).*sin(THE_Phi_pend))./2.0-(Lz_pend.*Tv_Z_pend.*m_pend.*sin(THE_Theta).*sin(THE_Phi_pend).*sin(THE_Psi_pend).*sin(THE_Theta_pend))./2.0-(Lz_pend.*Tv_Z_pend.*m_pend.*cos(THE_Theta).*cos(THE_Phi_pend).*sin(THE_Psi).*sin(THE_Psi_pend).*sin(THE_Theta_pend))./2.0,et36+et37+et38+et39+et40+et41+et42,et32+et33+et34+et35,et29+et30+et31];
mt4 = [(cos(THE_Phi).*(Tv_Z_pend.*m_pend.*cos(THE_Psi).*cos(THE_Theta).*2.0+cg_to_mot_H.*mprop.*cos(THE_Psi).*cos(THE_Theta).*8.0-Lz_pend.*m_pend.*sin(THE_Theta).*sin(THE_Phi_pend).*sin(THE_Psi_pend)-Lz_pend.*m_pend.*cos(THE_Theta).*cos(THE_Phi_pend).*sin(THE_Psi).*sin(THE_Psi_pend)-Lz_pend.*m_pend.*cos(THE_Phi_pend).*cos(THE_Psi_pend).*sin(THE_Theta).*sin(THE_Theta_pend)+Lz_pend.*m_pend.*cos(THE_Psi).*cos(THE_Theta).*cos(THE_Psi_pend).*cos(THE_Theta_pend)+Lz_pend.*m_pend.*cos(THE_Theta).*cos(THE_Psi_pend).*sin(THE_Psi).*sin(THE_Phi_pend).*sin(THE_Theta_pend)))./2.0,(sin(THE_Phi).*(Tv_Z_pend.*m_pend.*cos(THE_Psi).*cos(THE_Theta).*2.0+cg_to_mot_H.*mprop.*cos(THE_Psi).*cos(THE_Theta).*8.0-Lz_pend.*m_pend.*sin(THE_Theta).*sin(THE_Phi_pend).*sin(THE_Psi_pend)-Lz_pend.*m_pend.*cos(THE_Theta).*cos(THE_Phi_pend).*sin(THE_Psi).*sin(THE_Psi_pend)-Lz_pend.*m_pend.*cos(THE_Phi_pend).*cos(THE_Psi_pend).*sin(THE_Theta).*sin(THE_Theta_pend)+Lz_pend.*m_pend.*cos(THE_Psi).*cos(THE_Theta).*cos(THE_Psi_pend).*cos(THE_Theta_pend)+Lz_pend.*m_pend.*cos(THE_Theta).*cos(THE_Psi_pend).*sin(THE_Psi).*sin(THE_Phi_pend).*sin(THE_Theta_pend)))./2.0];
mt5 = [-Tv_Z_pend.*m_pend.*cos(THE_Psi).*sin(THE_Theta)-cg_to_mot_H.*mprop.*cos(THE_Psi).*sin(THE_Theta).*4.0-(Lz_pend.*m_pend.*cos(THE_Theta).*sin(THE_Phi_pend).*sin(THE_Psi_pend))./2.0-(Lz_pend.*m_pend.*cos(THE_Psi).*cos(THE_Psi_pend).*cos(THE_Theta_pend).*sin(THE_Theta))./2.0-(Lz_pend.*m_pend.*cos(THE_Theta).*cos(THE_Phi_pend).*cos(THE_Psi_pend).*sin(THE_Theta_pend))./2.0+(Lz_pend.*m_pend.*cos(THE_Phi_pend).*sin(THE_Psi).*sin(THE_Theta).*sin(THE_Psi_pend))./2.0-(Lz_pend.*m_pend.*cos(THE_Psi_pend).*sin(THE_Psi).*sin(THE_Theta).*sin(THE_Phi_pend).*sin(THE_Theta_pend))./2.0,et27+et28];
mt6 = [(Lx_pend.^2.*m_pend.*cos(THE_Psi).*cos(THE_Phi_pend))./1.2e+1+(Ly_pend.^2.*m_pend.*cos(THE_Psi).*cos(THE_Phi_pend))./1.2e+1-(Ly_pend.^2.*m_pend.*cos(THE_Psi).*cos(THE_Phi_pend).*cos(THE_Psi_pend).^2)./1.2e+1+(Lz_pend.^2.*m_pend.*cos(THE_Psi).*cos(THE_Phi_pend).*cos(THE_Psi_pend).^2)./3.0+(Ly_pend.^2.*m_pend.*cos(THE_Psi_pend).*cos(THE_Theta_pend).*sin(THE_Psi).*sin(THE_Psi_pend))./1.2e+1-(Lz_pend.^2.*m_pend.*cos(THE_Psi_pend).*cos(THE_Theta_pend).*sin(THE_Psi).*sin(THE_Psi_pend))./3.0-(Ly_pend.^2.*m_pend.*cos(THE_Psi).*cos(THE_Psi_pend).*sin(THE_Phi_pend).*sin(THE_Psi_pend).*sin(THE_Theta_pend))./1.2e+1+(Lz_pend.^2.*m_pend.*cos(THE_Psi).*cos(THE_Psi_pend).*sin(THE_Phi_pend).*sin(THE_Psi_pend).*sin(THE_Theta_pend))./3.0+(Lz_pend.*Tv_Z_pend.*m_pend.*cos(THE_Psi).*cos(THE_Phi_pend).*cos(THE_Psi_pend).*cos(THE_Theta_pend))./2.0];
mt7 = [(Ly_pend.^2.*m_pend.*sin(THE_Psi).*sin(THE_Theta_pend))./1.2e+1+(Lz_pend.^2.*m_pend.*sin(THE_Psi).*sin(THE_Theta_pend))./3.0+(Ly_pend.^2.*m_pend.*cos(THE_Psi).*cos(THE_Theta_pend).*sin(THE_Phi_pend))./1.2e+1+(Lz_pend.^2.*m_pend.*cos(THE_Psi).*cos(THE_Theta_pend).*sin(THE_Phi_pend))./3.0+(Lz_pend.*Tv_Z_pend.*m_pend.*cos(THE_Psi).*cos(THE_Psi_pend).*sin(THE_Phi_pend))./2.0-(Lz_pend.*Tv_Z_pend.*m_pend.*cos(THE_Psi).*cos(THE_Phi_pend).*sin(THE_Psi_pend).*sin(THE_Theta_pend))./2.0,et48+et49+et50+et51,et45+et46+et47,et43+et44];
mt8 = [Tv_Z_pend.*m_pend.*cos(THE_Psi).*sin(THE_Phi)+cg_to_mot_H.*mprop.*cos(THE_Psi).*sin(THE_Phi).*4.0-Tv_Z_pend.*m_pend.*cos(THE_Phi).*sin(THE_Psi).*sin(THE_Theta)-cg_to_mot_H.*mprop.*cos(THE_Phi).*sin(THE_Psi).*sin(THE_Theta).*4.0+(Lz_pend.*m_pend.*cos(THE_Psi).*cos(THE_Psi_pend).*cos(THE_Theta_pend).*sin(THE_Phi))./2.0-(Lz_pend.*m_pend.*cos(THE_Phi_pend).*sin(THE_Phi).*sin(THE_Psi).*sin(THE_Psi_pend))./2.0-(Lz_pend.*m_pend.*cos(THE_Phi).*cos(THE_Psi).*cos(THE_Phi_pend).*sin(THE_Theta).*sin(THE_Psi_pend))./2.0-(Lz_pend.*m_pend.*cos(THE_Phi).*cos(THE_Psi_pend).*cos(THE_Theta_pend).*sin(THE_Psi).*sin(THE_Theta))./2.0+(Lz_pend.*m_pend.*cos(THE_Psi_pend).*sin(THE_Phi).*sin(THE_Psi).*sin(THE_Phi_pend).*sin(THE_Theta_pend))./2.0+(Lz_pend.*m_pend.*cos(THE_Phi).*cos(THE_Psi).*cos(THE_Psi_pend).*sin(THE_Theta).*sin(THE_Phi_pend).*sin(THE_Theta_pend))./2.0];
mt9 = [-Tv_Z_pend.*m_pend.*cos(THE_Phi).*cos(THE_Psi)-cg_to_mot_H.*mprop.*cos(THE_Phi).*cos(THE_Psi).*4.0-Tv_Z_pend.*m_pend.*sin(THE_Phi).*sin(THE_Psi).*sin(THE_Theta)-cg_to_mot_H.*mprop.*sin(THE_Phi).*sin(THE_Psi).*sin(THE_Theta).*4.0+(Lz_pend.*m_pend.*cos(THE_Phi).*cos(THE_Phi_pend).*sin(THE_Psi).*sin(THE_Psi_pend))./2.0-(Lz_pend.*m_pend.*cos(THE_Phi).*cos(THE_Psi).*cos(THE_Psi_pend).*cos(THE_Theta_pend))./2.0-(Lz_pend.*m_pend.*cos(THE_Psi).*cos(THE_Phi_pend).*sin(THE_Phi).*sin(THE_Theta).*sin(THE_Psi_pend))./2.0-(Lz_pend.*m_pend.*cos(THE_Psi_pend).*cos(THE_Theta_pend).*sin(THE_Phi).*sin(THE_Psi).*sin(THE_Theta))./2.0-(Lz_pend.*m_pend.*cos(THE_Phi).*cos(THE_Psi_pend).*sin(THE_Psi).*sin(THE_Phi_pend).*sin(THE_Theta_pend))./2.0+(Lz_pend.*m_pend.*cos(THE_Psi).*cos(THE_Psi_pend).*sin(THE_Phi).*sin(THE_Theta).*sin(THE_Phi_pend).*sin(THE_Theta_pend))./2.0,cos(THE_Theta).*(Tv_Z_pend.*m_pend.*sin(THE_Psi).*2.0+cg_to_mot_H.*mprop.*sin(THE_Psi).*8.0+Lz_pend.*m_pend.*cos(THE_Psi).*cos(THE_Phi_pend).*sin(THE_Psi_pend)+Lz_pend.*m_pend.*cos(THE_Psi_pend).*cos(THE_Theta_pend).*sin(THE_Psi)-Lz_pend.*m_pend.*cos(THE_Psi).*cos(THE_Psi_pend).*sin(THE_Phi_pend).*sin(THE_Theta_pend)).*(-1.0./2.0)];
mt10 = [(Lx_pend.^2.*m_pend.*cos(THE_Phi_pend).*cos(THE_Theta_pend).*sin(THE_Theta_pend))./1.2e+1-(Ly_pend.^2.*m_pend.*cos(THE_Phi_pend).*cos(THE_Theta_pend).*sin(THE_Theta_pend))./1.2e+1-(Lz_pend.*Tv_Z_pend.*m_pend.*sin(THE_Phi_pend).*sin(THE_Psi_pend))./2.0+(Ly_pend.^2.*m_pend.*cos(THE_Psi_pend).*cos(THE_Theta_pend).*sin(THE_Phi_pend).*sin(THE_Psi_pend))./1.2e+1-(Lz_pend.^2.*m_pend.*cos(THE_Psi_pend).*cos(THE_Theta_pend).*sin(THE_Phi_pend).*sin(THE_Psi_pend))./3.0-(Lz_pend.*Tv_Z_pend.*m_pend.*cos(THE_Phi_pend).*cos(THE_Psi_pend).*sin(THE_Theta_pend))./2.0+(Ly_pend.^2.*m_pend.*cos(THE_Phi_pend).*cos(THE_Psi_pend).^2.*cos(THE_Theta_pend).*sin(THE_Theta_pend))./1.2e+1-(Lz_pend.^2.*m_pend.*cos(THE_Phi_pend).*cos(THE_Psi_pend).^2.*cos(THE_Theta_pend).*sin(THE_Theta_pend))./3.0];
mt11 = [m_pend.*(Lx_pend.^2.*sin(THE_Phi_pend)+Ly_pend.^2.*sin(THE_Phi_pend)-Ly_pend.^2.*cos(THE_Psi_pend).^2.*sin(THE_Phi_pend)+Lz_pend.^2.*cos(THE_Psi_pend).^2.*sin(THE_Phi_pend).*4.0+Ly_pend.^2.*cos(THE_Phi_pend).*cos(THE_Psi_pend).*sin(THE_Psi_pend).*sin(THE_Theta_pend)-Lz_pend.^2.*cos(THE_Phi_pend).*cos(THE_Psi_pend).*sin(THE_Psi_pend).*sin(THE_Theta_pend).*4.0+Lz_pend.*Tv_Z_pend.*cos(THE_Psi_pend).*cos(THE_Theta_pend).*sin(THE_Phi_pend).*6.0).*(-1.0./1.2e+1),(m_pend.*(Ly_pend.^2.*cos(THE_Phi_pend).*cos(THE_Theta_pend)+Lz_pend.^2.*cos(THE_Phi_pend).*cos(THE_Theta_pend).*4.0+Lz_pend.*Tv_Z_pend.*cos(THE_Phi_pend).*cos(THE_Psi_pend).*6.0+Lz_pend.*Tv_Z_pend.*sin(THE_Phi_pend).*sin(THE_Psi_pend).*sin(THE_Theta_pend).*6.0))./1.2e+1];
mt12 = [Tv_Z_pend.*m_pend.*cos(THE_Phi).*sin(THE_Psi)+cg_to_mot_H.*mprop.*cos(THE_Phi).*sin(THE_Psi).*4.0-Tv_Z_pend.*m_pend.*cos(THE_Psi).*sin(THE_Phi).*sin(THE_Theta)-cg_to_mot_H.*mprop.*cos(THE_Psi).*sin(THE_Phi).*sin(THE_Theta).*4.0+(Lz_pend.*m_pend.*cos(THE_Phi).*cos(THE_Psi).*cos(THE_Phi_pend).*sin(THE_Psi_pend))./2.0+(Lz_pend.*m_pend.*cos(THE_Phi).*cos(THE_Psi_pend).*cos(THE_Theta_pend).*sin(THE_Psi))./2.0-(Lz_pend.*m_pend.*cos(THE_Theta).*sin(THE_Phi).*sin(THE_Phi_pend).*sin(THE_Psi_pend))./2.0-(Lz_pend.*m_pend.*cos(THE_Psi).*cos(THE_Psi_pend).*cos(THE_Theta_pend).*sin(THE_Phi).*sin(THE_Theta))./2.0-(Lz_pend.*m_pend.*cos(THE_Phi).*cos(THE_Psi).*cos(THE_Psi_pend).*sin(THE_Phi_pend).*sin(THE_Theta_pend))./2.0-(Lz_pend.*m_pend.*cos(THE_Theta).*cos(THE_Phi_pend).*cos(THE_Psi_pend).*sin(THE_Phi).*sin(THE_Theta_pend))./2.0+(Lz_pend.*m_pend.*cos(THE_Phi_pend).*sin(THE_Phi).*sin(THE_Psi).*sin(THE_Theta).*sin(THE_Psi_pend))./2.0-(Lz_pend.*m_pend.*cos(THE_Psi_pend).*sin(THE_Phi).*sin(THE_Psi).*sin(THE_Theta).*sin(THE_Phi_pend).*sin(THE_Theta_pend))./2.0];
mt13 = [(cos(THE_Phi).*(Tv_Z_pend.*m_pend.*cos(THE_Psi).*cos(THE_Theta).*2.0+cg_to_mot_H.*mprop.*cos(THE_Psi).*cos(THE_Theta).*8.0-Lz_pend.*m_pend.*sin(THE_Theta).*sin(THE_Phi_pend).*sin(THE_Psi_pend)-Lz_pend.*m_pend.*cos(THE_Theta).*cos(THE_Phi_pend).*sin(THE_Psi).*sin(THE_Psi_pend)-Lz_pend.*m_pend.*cos(THE_Phi_pend).*cos(THE_Psi_pend).*sin(THE_Theta).*sin(THE_Theta_pend)+Lz_pend.*m_pend.*cos(THE_Psi).*cos(THE_Theta).*cos(THE_Psi_pend).*cos(THE_Theta_pend)+Lz_pend.*m_pend.*cos(THE_Theta).*cos(THE_Psi_pend).*sin(THE_Psi).*sin(THE_Phi_pend).*sin(THE_Theta_pend)))./2.0];
mt14 = [Tv_Z_pend.*m_pend.*cos(THE_Psi).*sin(THE_Phi)+cg_to_mot_H.*mprop.*cos(THE_Psi).*sin(THE_Phi).*4.0-Tv_Z_pend.*m_pend.*cos(THE_Phi).*sin(THE_Psi).*sin(THE_Theta)-cg_to_mot_H.*mprop.*cos(THE_Phi).*sin(THE_Psi).*sin(THE_Theta).*4.0+(Lz_pend.*m_pend.*cos(THE_Psi).*cos(THE_Psi_pend).*cos(THE_Theta_pend).*sin(THE_Phi))./2.0-(Lz_pend.*m_pend.*cos(THE_Phi_pend).*sin(THE_Phi).*sin(THE_Psi).*sin(THE_Psi_pend))./2.0-(Lz_pend.*m_pend.*cos(THE_Phi).*cos(THE_Psi).*cos(THE_Phi_pend).*sin(THE_Theta).*sin(THE_Psi_pend))./2.0-(Lz_pend.*m_pend.*cos(THE_Phi).*cos(THE_Psi_pend).*cos(THE_Theta_pend).*sin(THE_Psi).*sin(THE_Theta))./2.0+(Lz_pend.*m_pend.*cos(THE_Psi_pend).*sin(THE_Phi).*sin(THE_Psi).*sin(THE_Phi_pend).*sin(THE_Theta_pend))./2.0+(Lz_pend.*m_pend.*cos(THE_Phi).*cos(THE_Psi).*cos(THE_Psi_pend).*sin(THE_Theta).*sin(THE_Phi_pend).*sin(THE_Theta_pend))./2.0,m+m_pend+mprop.*4.0,0.0,0.0];
mt15 = [(Lz_pend.*m_pend.*(cos(THE_Phi).*cos(THE_Theta).*cos(THE_Phi_pend).*sin(THE_Psi_pend)-cos(THE_Psi).*sin(THE_Phi).*sin(THE_Phi_pend).*sin(THE_Psi_pend)-cos(THE_Psi).*cos(THE_Phi_pend).*cos(THE_Psi_pend).*sin(THE_Phi).*sin(THE_Theta_pend)-cos(THE_Phi).*cos(THE_Theta).*cos(THE_Psi_pend).*sin(THE_Phi_pend).*sin(THE_Theta_pend)+cos(THE_Phi).*sin(THE_Psi).*sin(THE_Theta).*sin(THE_Phi_pend).*sin(THE_Psi_pend)+cos(THE_Phi).*cos(THE_Phi_pend).*cos(THE_Psi_pend).*sin(THE_Psi).*sin(THE_Theta).*sin(THE_Theta_pend)))./2.0,Lz_pend.*m_pend.*cos(THE_Psi_pend).*(sin(THE_Phi).*sin(THE_Psi).*sin(THE_Theta_pend)-cos(THE_Phi).*cos(THE_Theta).*cos(THE_Phi_pend).*cos(THE_Theta_pend)+cos(THE_Phi).*cos(THE_Psi).*sin(THE_Theta).*sin(THE_Theta_pend)+cos(THE_Psi).*cos(THE_Theta_pend).*sin(THE_Phi).*sin(THE_Phi_pend)-cos(THE_Phi).*cos(THE_Theta_pend).*sin(THE_Psi).*sin(THE_Theta).*sin(THE_Phi_pend)).*(-1.0./2.0)];
mt16 = [Lz_pend.*m_pend.*(-cos(THE_Psi).*cos(THE_Phi_pend).*cos(THE_Psi_pend).*sin(THE_Phi)-cos(THE_Phi).*cos(THE_Theta).*cos(THE_Psi_pend).*sin(THE_Phi_pend)+cos(THE_Theta_pend).*sin(THE_Phi).*sin(THE_Psi).*sin(THE_Psi_pend)+cos(THE_Phi).*cos(THE_Phi_pend).*cos(THE_Psi_pend).*sin(THE_Psi).*sin(THE_Theta)+cos(THE_Phi).*cos(THE_Psi).*cos(THE_Theta_pend).*sin(THE_Theta).*sin(THE_Psi_pend)+cos(THE_Phi).*cos(THE_Theta).*cos(THE_Phi_pend).*sin(THE_Psi_pend).*sin(THE_Theta_pend)-cos(THE_Psi).*sin(THE_Phi).*sin(THE_Phi_pend).*sin(THE_Psi_pend).*sin(THE_Theta_pend)+cos(THE_Phi).*sin(THE_Psi).*sin(THE_Theta).*sin(THE_Phi_pend).*sin(THE_Psi_pend).*sin(THE_Theta_pend)).*(-1.0./2.0)];
mt17 = [Tv_Z_pend.*m_pend.*sin(THE_Phi).*sin(THE_Psi)+cg_to_mot_H.*mprop.*sin(THE_Phi).*sin(THE_Psi).*4.0+Tv_Z_pend.*m_pend.*cos(THE_Phi).*cos(THE_Psi).*sin(THE_Theta)+cg_to_mot_H.*mprop.*cos(THE_Phi).*cos(THE_Psi).*sin(THE_Theta).*4.0+(Lz_pend.*m_pend.*cos(THE_Psi).*cos(THE_Phi_pend).*sin(THE_Phi).*sin(THE_Psi_pend))./2.0+(Lz_pend.*m_pend.*cos(THE_Phi).*cos(THE_Theta).*sin(THE_Phi_pend).*sin(THE_Psi_pend))./2.0+(Lz_pend.*m_pend.*cos(THE_Psi_pend).*cos(THE_Theta_pend).*sin(THE_Phi).*sin(THE_Psi))./2.0+(Lz_pend.*m_pend.*cos(THE_Phi).*cos(THE_Psi).*cos(THE_Psi_pend).*cos(THE_Theta_pend).*sin(THE_Theta))./2.0+(Lz_pend.*m_pend.*cos(THE_Phi).*cos(THE_Theta).*cos(THE_Phi_pend).*cos(THE_Psi_pend).*sin(THE_Theta_pend))./2.0-(Lz_pend.*m_pend.*cos(THE_Phi).*cos(THE_Phi_pend).*sin(THE_Psi).*sin(THE_Theta).*sin(THE_Psi_pend))./2.0-(Lz_pend.*m_pend.*cos(THE_Psi).*cos(THE_Psi_pend).*sin(THE_Phi).*sin(THE_Phi_pend).*sin(THE_Theta_pend))./2.0+(Lz_pend.*m_pend.*cos(THE_Phi).*cos(THE_Psi_pend).*sin(THE_Psi).*sin(THE_Theta).*sin(THE_Phi_pend).*sin(THE_Theta_pend))./2.0];
mt18 = [(sin(THE_Phi).*(Tv_Z_pend.*m_pend.*cos(THE_Psi).*cos(THE_Theta).*2.0+cg_to_mot_H.*mprop.*cos(THE_Psi).*cos(THE_Theta).*8.0-Lz_pend.*m_pend.*sin(THE_Theta).*sin(THE_Phi_pend).*sin(THE_Psi_pend)-Lz_pend.*m_pend.*cos(THE_Theta).*cos(THE_Phi_pend).*sin(THE_Psi).*sin(THE_Psi_pend)-Lz_pend.*m_pend.*cos(THE_Phi_pend).*cos(THE_Psi_pend).*sin(THE_Theta).*sin(THE_Theta_pend)+Lz_pend.*m_pend.*cos(THE_Psi).*cos(THE_Theta).*cos(THE_Psi_pend).*cos(THE_Theta_pend)+Lz_pend.*m_pend.*cos(THE_Theta).*cos(THE_Psi_pend).*sin(THE_Psi).*sin(THE_Phi_pend).*sin(THE_Theta_pend)))./2.0];
mt19 = [-Tv_Z_pend.*m_pend.*cos(THE_Phi).*cos(THE_Psi)-cg_to_mot_H.*mprop.*cos(THE_Phi).*cos(THE_Psi).*4.0-Tv_Z_pend.*m_pend.*sin(THE_Phi).*sin(THE_Psi).*sin(THE_Theta)-cg_to_mot_H.*mprop.*sin(THE_Phi).*sin(THE_Psi).*sin(THE_Theta).*4.0+(Lz_pend.*m_pend.*cos(THE_Phi).*cos(THE_Phi_pend).*sin(THE_Psi).*sin(THE_Psi_pend))./2.0-(Lz_pend.*m_pend.*cos(THE_Phi).*cos(THE_Psi).*cos(THE_Psi_pend).*cos(THE_Theta_pend))./2.0-(Lz_pend.*m_pend.*cos(THE_Psi).*cos(THE_Phi_pend).*sin(THE_Phi).*sin(THE_Theta).*sin(THE_Psi_pend))./2.0-(Lz_pend.*m_pend.*cos(THE_Psi_pend).*cos(THE_Theta_pend).*sin(THE_Phi).*sin(THE_Psi).*sin(THE_Theta))./2.0-(Lz_pend.*m_pend.*cos(THE_Phi).*cos(THE_Psi_pend).*sin(THE_Psi).*sin(THE_Phi_pend).*sin(THE_Theta_pend))./2.0+(Lz_pend.*m_pend.*cos(THE_Psi).*cos(THE_Psi_pend).*sin(THE_Phi).*sin(THE_Theta).*sin(THE_Phi_pend).*sin(THE_Theta_pend))./2.0,0.0,m+m_pend+mprop.*4.0,0.0];
mt20 = [(Lz_pend.*m_pend.*(cos(THE_Phi).*cos(THE_Psi).*sin(THE_Phi_pend).*sin(THE_Psi_pend)+cos(THE_Theta).*cos(THE_Phi_pend).*sin(THE_Phi).*sin(THE_Psi_pend)+cos(THE_Phi).*cos(THE_Psi).*cos(THE_Phi_pend).*cos(THE_Psi_pend).*sin(THE_Theta_pend)-cos(THE_Theta).*cos(THE_Psi_pend).*sin(THE_Phi).*sin(THE_Phi_pend).*sin(THE_Theta_pend)+sin(THE_Phi).*sin(THE_Psi).*sin(THE_Theta).*sin(THE_Phi_pend).*sin(THE_Psi_pend)+cos(THE_Phi_pend).*cos(THE_Psi_pend).*sin(THE_Phi).*sin(THE_Psi).*sin(THE_Theta).*sin(THE_Theta_pend)))./2.0,(Lz_pend.*m_pend.*cos(THE_Psi_pend).*(cos(THE_Phi).*sin(THE_Psi).*sin(THE_Theta_pend)+cos(THE_Phi).*cos(THE_Psi).*cos(THE_Theta_pend).*sin(THE_Phi_pend)+cos(THE_Theta).*cos(THE_Phi_pend).*cos(THE_Theta_pend).*sin(THE_Phi)-cos(THE_Psi).*sin(THE_Phi).*sin(THE_Theta).*sin(THE_Theta_pend)+cos(THE_Theta_pend).*sin(THE_Phi).*sin(THE_Psi).*sin(THE_Theta).*sin(THE_Phi_pend)))./2.0];
mt21 = [Lz_pend.*m_pend.*(cos(THE_Phi).*cos(THE_Psi).*cos(THE_Phi_pend).*cos(THE_Psi_pend)-cos(THE_Theta).*cos(THE_Psi_pend).*sin(THE_Phi).*sin(THE_Phi_pend)-cos(THE_Phi).*cos(THE_Theta_pend).*sin(THE_Psi).*sin(THE_Psi_pend)+cos(THE_Phi_pend).*cos(THE_Psi_pend).*sin(THE_Phi).*sin(THE_Psi).*sin(THE_Theta)+cos(THE_Psi).*cos(THE_Theta_pend).*sin(THE_Phi).*sin(THE_Theta).*sin(THE_Psi_pend)+cos(THE_Phi).*cos(THE_Psi).*sin(THE_Phi_pend).*sin(THE_Psi_pend).*sin(THE_Theta_pend)+cos(THE_Theta).*cos(THE_Phi_pend).*sin(THE_Phi).*sin(THE_Psi_pend).*sin(THE_Theta_pend)+sin(THE_Phi).*sin(THE_Psi).*sin(THE_Theta).*sin(THE_Phi_pend).*sin(THE_Psi_pend).*sin(THE_Theta_pend)).*(-1.0./2.0),0.0,-Tv_Z_pend.*m_pend.*cos(THE_Psi).*sin(THE_Theta)-cg_to_mot_H.*mprop.*cos(THE_Psi).*sin(THE_Theta).*4.0-(Lz_pend.*m_pend.*cos(THE_Theta).*sin(THE_Phi_pend).*sin(THE_Psi_pend))./2.0-(Lz_pend.*m_pend.*cos(THE_Psi).*cos(THE_Psi_pend).*cos(THE_Theta_pend).*sin(THE_Theta))./2.0-(Lz_pend.*m_pend.*cos(THE_Theta).*cos(THE_Phi_pend).*cos(THE_Psi_pend).*sin(THE_Theta_pend))./2.0+(Lz_pend.*m_pend.*cos(THE_Phi_pend).*sin(THE_Psi).*sin(THE_Theta).*sin(THE_Psi_pend))./2.0-(Lz_pend.*m_pend.*cos(THE_Psi_pend).*sin(THE_Psi).*sin(THE_Theta).*sin(THE_Phi_pend).*sin(THE_Theta_pend))./2.0];
mt22 = [cos(THE_Theta).*(Tv_Z_pend.*m_pend.*sin(THE_Psi).*2.0+cg_to_mot_H.*mprop.*sin(THE_Psi).*8.0+Lz_pend.*m_pend.*cos(THE_Psi).*cos(THE_Phi_pend).*sin(THE_Psi_pend)+Lz_pend.*m_pend.*cos(THE_Psi_pend).*cos(THE_Theta_pend).*sin(THE_Psi)-Lz_pend.*m_pend.*cos(THE_Psi).*cos(THE_Psi_pend).*sin(THE_Phi_pend).*sin(THE_Theta_pend)).*(-1.0./2.0),0.0,0.0,m+m_pend+mprop.*4.0,(Lz_pend.*m_pend.*(-cos(THE_Phi_pend).*sin(THE_Theta).*sin(THE_Psi_pend)+cos(THE_Theta).*sin(THE_Psi).*sin(THE_Phi_pend).*sin(THE_Psi_pend)+cos(THE_Psi_pend).*sin(THE_Theta).*sin(THE_Phi_pend).*sin(THE_Theta_pend)+cos(THE_Theta).*cos(THE_Phi_pend).*cos(THE_Psi_pend).*sin(THE_Psi).*sin(THE_Theta_pend)))./2.0,Lz_pend.*m_pend.*cos(THE_Psi_pend).*(cos(THE_Psi).*cos(THE_Theta).*sin(THE_Theta_pend)+cos(THE_Phi_pend).*cos(THE_Theta_pend).*sin(THE_Theta)-cos(THE_Theta).*cos(THE_Theta_pend).*sin(THE_Psi).*sin(THE_Phi_pend)).*(-1.0./2.0),Lz_pend.*m_pend.*(cos(THE_Psi_pend).*sin(THE_Theta).*sin(THE_Phi_pend)+cos(THE_Theta).*cos(THE_Phi_pend).*cos(THE_Psi_pend).*sin(THE_Psi)+cos(THE_Psi).*cos(THE_Theta).*cos(THE_Theta_pend).*sin(THE_Psi_pend)-cos(THE_Phi_pend).*sin(THE_Theta).*sin(THE_Psi_pend).*sin(THE_Theta_pend)+cos(THE_Theta).*sin(THE_Psi).*sin(THE_Phi_pend).*sin(THE_Psi_pend).*sin(THE_Theta_pend)).*(-1.0./2.0),et54+et55+et56];
mt23 = [et52+et53,(Lx_pend.^2.*m_pend.*cos(THE_Phi_pend).*cos(THE_Theta_pend).*sin(THE_Theta_pend))./1.2e+1-(Ly_pend.^2.*m_pend.*cos(THE_Phi_pend).*cos(THE_Theta_pend).*sin(THE_Theta_pend))./1.2e+1-(Lz_pend.*Tv_Z_pend.*m_pend.*sin(THE_Phi_pend).*sin(THE_Psi_pend))./2.0+(Ly_pend.^2.*m_pend.*cos(THE_Psi_pend).*cos(THE_Theta_pend).*sin(THE_Phi_pend).*sin(THE_Psi_pend))./1.2e+1-(Lz_pend.^2.*m_pend.*cos(THE_Psi_pend).*cos(THE_Theta_pend).*sin(THE_Phi_pend).*sin(THE_Psi_pend))./3.0-(Lz_pend.*Tv_Z_pend.*m_pend.*cos(THE_Phi_pend).*cos(THE_Psi_pend).*sin(THE_Theta_pend))./2.0+(Ly_pend.^2.*m_pend.*cos(THE_Phi_pend).*cos(THE_Psi_pend).^2.*cos(THE_Theta_pend).*sin(THE_Theta_pend))./1.2e+1-(Lz_pend.^2.*m_pend.*cos(THE_Phi_pend).*cos(THE_Psi_pend).^2.*cos(THE_Theta_pend).*sin(THE_Theta_pend))./3.0];
mt24 = [(Lz_pend.*m_pend.*(cos(THE_Phi).*cos(THE_Theta).*cos(THE_Phi_pend).*sin(THE_Psi_pend)-cos(THE_Psi).*sin(THE_Phi).*sin(THE_Phi_pend).*sin(THE_Psi_pend)-cos(THE_Psi).*cos(THE_Phi_pend).*cos(THE_Psi_pend).*sin(THE_Phi).*sin(THE_Theta_pend)-cos(THE_Phi).*cos(THE_Theta).*cos(THE_Psi_pend).*sin(THE_Phi_pend).*sin(THE_Theta_pend)+cos(THE_Phi).*sin(THE_Psi).*sin(THE_Theta).*sin(THE_Phi_pend).*sin(THE_Psi_pend)+cos(THE_Phi).*cos(THE_Phi_pend).*cos(THE_Psi_pend).*sin(THE_Psi).*sin(THE_Theta).*sin(THE_Theta_pend)))./2.0,(Lz_pend.*m_pend.*(cos(THE_Phi).*cos(THE_Psi).*sin(THE_Phi_pend).*sin(THE_Psi_pend)+cos(THE_Theta).*cos(THE_Phi_pend).*sin(THE_Phi).*sin(THE_Psi_pend)+cos(THE_Phi).*cos(THE_Psi).*cos(THE_Phi_pend).*cos(THE_Psi_pend).*sin(THE_Theta_pend)-cos(THE_Theta).*cos(THE_Psi_pend).*sin(THE_Phi).*sin(THE_Phi_pend).*sin(THE_Theta_pend)+sin(THE_Phi).*sin(THE_Psi).*sin(THE_Theta).*sin(THE_Phi_pend).*sin(THE_Psi_pend)+cos(THE_Phi_pend).*cos(THE_Psi_pend).*sin(THE_Phi).*sin(THE_Psi).*sin(THE_Theta).*sin(THE_Theta_pend)))./2.0,(Lz_pend.*m_pend.*(-cos(THE_Phi_pend).*sin(THE_Theta).*sin(THE_Psi_pend)+cos(THE_Theta).*sin(THE_Psi).*sin(THE_Phi_pend).*sin(THE_Psi_pend)+cos(THE_Psi_pend).*sin(THE_Theta).*sin(THE_Phi_pend).*sin(THE_Theta_pend)+cos(THE_Theta).*cos(THE_Phi_pend).*cos(THE_Psi_pend).*sin(THE_Psi).*sin(THE_Theta_pend)))./2.0];
mt25 = [(m_pend.*(-Lx_pend.^2.*sin(THE_Theta_pend).^2-Ly_pend.^2.*sin(THE_Psi_pend).^2+Lz_pend.^2.*sin(THE_Psi_pend).^2.*4.0+Lz_pend.^2.*sin(THE_Theta_pend).^2.*4.0+Lx_pend.^2+Ly_pend.^2+Ly_pend.^2.*sin(THE_Psi_pend).^2.*sin(THE_Theta_pend).^2-Lz_pend.^2.*sin(THE_Psi_pend).^2.*sin(THE_Theta_pend).^2.*4.0))./1.2e+1,m_pend.*cos(THE_Psi_pend).*cos(THE_Theta_pend).*sin(THE_Psi_pend).*(Ly_pend.^2-Lz_pend.^2.*4.0).*(-1.0./1.2e+1),m_pend.*sin(THE_Theta_pend).*(Ly_pend.^2+Lz_pend.^2.*4.0).*(-1.0./1.2e+1),et57+et58];
mt26 = [(Lx_pend.^2.*m_pend.*cos(THE_Psi).*cos(THE_Phi_pend))./1.2e+1+(Ly_pend.^2.*m_pend.*cos(THE_Psi).*cos(THE_Phi_pend))./1.2e+1-(Ly_pend.^2.*m_pend.*cos(THE_Psi).*cos(THE_Phi_pend).*cos(THE_Psi_pend).^2)./1.2e+1+(Lz_pend.^2.*m_pend.*cos(THE_Psi).*cos(THE_Phi_pend).*cos(THE_Psi_pend).^2)./3.0+(Ly_pend.^2.*m_pend.*cos(THE_Psi_pend).*cos(THE_Theta_pend).*sin(THE_Psi).*sin(THE_Psi_pend))./1.2e+1-(Lz_pend.^2.*m_pend.*cos(THE_Psi_pend).*cos(THE_Theta_pend).*sin(THE_Psi).*sin(THE_Psi_pend))./3.0-(Ly_pend.^2.*m_pend.*cos(THE_Psi).*cos(THE_Psi_pend).*sin(THE_Phi_pend).*sin(THE_Psi_pend).*sin(THE_Theta_pend))./1.2e+1+(Lz_pend.^2.*m_pend.*cos(THE_Psi).*cos(THE_Psi_pend).*sin(THE_Phi_pend).*sin(THE_Psi_pend).*sin(THE_Theta_pend))./3.0+(Lz_pend.*Tv_Z_pend.*m_pend.*cos(THE_Psi).*cos(THE_Phi_pend).*cos(THE_Psi_pend).*cos(THE_Theta_pend))./2.0];
mt27 = [m_pend.*(Lx_pend.^2.*sin(THE_Phi_pend)+Ly_pend.^2.*sin(THE_Phi_pend)-Ly_pend.^2.*cos(THE_Psi_pend).^2.*sin(THE_Phi_pend)+Lz_pend.^2.*cos(THE_Psi_pend).^2.*sin(THE_Phi_pend).*4.0+Ly_pend.^2.*cos(THE_Phi_pend).*cos(THE_Psi_pend).*sin(THE_Psi_pend).*sin(THE_Theta_pend)-Lz_pend.^2.*cos(THE_Phi_pend).*cos(THE_Psi_pend).*sin(THE_Psi_pend).*sin(THE_Theta_pend).*4.0+Lz_pend.*Tv_Z_pend.*cos(THE_Psi_pend).*cos(THE_Theta_pend).*sin(THE_Phi_pend).*6.0).*(-1.0./1.2e+1),Lz_pend.*m_pend.*cos(THE_Psi_pend).*(sin(THE_Phi).*sin(THE_Psi).*sin(THE_Theta_pend)-cos(THE_Phi).*cos(THE_Theta).*cos(THE_Phi_pend).*cos(THE_Theta_pend)+cos(THE_Phi).*cos(THE_Psi).*sin(THE_Theta).*sin(THE_Theta_pend)+cos(THE_Psi).*cos(THE_Theta_pend).*sin(THE_Phi).*sin(THE_Phi_pend)-cos(THE_Phi).*cos(THE_Theta_pend).*sin(THE_Psi).*sin(THE_Theta).*sin(THE_Phi_pend)).*(-1.0./2.0),(Lz_pend.*m_pend.*cos(THE_Psi_pend).*(cos(THE_Phi).*sin(THE_Psi).*sin(THE_Theta_pend)+cos(THE_Phi).*cos(THE_Psi).*cos(THE_Theta_pend).*sin(THE_Phi_pend)+cos(THE_Theta).*cos(THE_Phi_pend).*cos(THE_Theta_pend).*sin(THE_Phi)-cos(THE_Psi).*sin(THE_Phi).*sin(THE_Theta).*sin(THE_Theta_pend)+cos(THE_Theta_pend).*sin(THE_Phi).*sin(THE_Psi).*sin(THE_Theta).*sin(THE_Phi_pend)))./2.0];
mt28 = [Lz_pend.*m_pend.*cos(THE_Psi_pend).*(cos(THE_Psi).*cos(THE_Theta).*sin(THE_Theta_pend)+cos(THE_Phi_pend).*cos(THE_Theta_pend).*sin(THE_Theta)-cos(THE_Theta).*cos(THE_Theta_pend).*sin(THE_Psi).*sin(THE_Phi_pend)).*(-1.0./2.0),m_pend.*cos(THE_Psi_pend).*cos(THE_Theta_pend).*sin(THE_Psi_pend).*(Ly_pend.^2-Lz_pend.^2.*4.0).*(-1.0./1.2e+1),(m_pend.*(Ly_pend.^2.*sin(THE_Psi_pend).^2-Lz_pend.^2.*sin(THE_Psi_pend).^2.*4.0+Lx_pend.^2+Lz_pend.^2.*4.0))./1.2e+1,0.0];
mt29 = [Ly_pend.^2.*m_pend.*cos(THE_Psi).*cos(THE_Theta).*sin(THE_Theta_pend).*(-1.0./1.2e+1)-(Ly_pend.^2.*m_pend.*cos(THE_Phi_pend).*cos(THE_Theta_pend).*sin(THE_Theta))./1.2e+1-(Lz_pend.^2.*m_pend.*cos(THE_Psi).*cos(THE_Theta).*sin(THE_Theta_pend))./3.0-(Lz_pend.^2.*m_pend.*cos(THE_Phi_pend).*cos(THE_Theta_pend).*sin(THE_Theta))./3.0+(Ly_pend.^2.*m_pend.*cos(THE_Theta).*cos(THE_Theta_pend).*sin(THE_Psi).*sin(THE_Phi_pend))./1.2e+1+(Lz_pend.^2.*m_pend.*cos(THE_Theta).*cos(THE_Theta_pend).*sin(THE_Psi).*sin(THE_Phi_pend))./3.0-(Lz_pend.*Tv_Z_pend.*m_pend.*cos(THE_Phi_pend).*cos(THE_Psi_pend).*sin(THE_Theta))./2.0+(Lz_pend.*Tv_Z_pend.*m_pend.*cos(THE_Theta).*cos(THE_Psi_pend).*sin(THE_Psi).*sin(THE_Phi_pend))./2.0-(Lz_pend.*Tv_Z_pend.*m_pend.*sin(THE_Theta).*sin(THE_Phi_pend).*sin(THE_Psi_pend).*sin(THE_Theta_pend))./2.0-(Lz_pend.*Tv_Z_pend.*m_pend.*cos(THE_Theta).*cos(THE_Phi_pend).*sin(THE_Psi).*sin(THE_Psi_pend).*sin(THE_Theta_pend))./2.0];
mt30 = [(Ly_pend.^2.*m_pend.*sin(THE_Psi).*sin(THE_Theta_pend))./1.2e+1+(Lz_pend.^2.*m_pend.*sin(THE_Psi).*sin(THE_Theta_pend))./3.0+(Ly_pend.^2.*m_pend.*cos(THE_Psi).*cos(THE_Theta_pend).*sin(THE_Phi_pend))./1.2e+1+(Lz_pend.^2.*m_pend.*cos(THE_Psi).*cos(THE_Theta_pend).*sin(THE_Phi_pend))./3.0+(Lz_pend.*Tv_Z_pend.*m_pend.*cos(THE_Psi).*cos(THE_Psi_pend).*sin(THE_Phi_pend))./2.0-(Lz_pend.*Tv_Z_pend.*m_pend.*cos(THE_Psi).*cos(THE_Phi_pend).*sin(THE_Psi_pend).*sin(THE_Theta_pend))./2.0,(m_pend.*(Ly_pend.^2.*cos(THE_Phi_pend).*cos(THE_Theta_pend)+Lz_pend.^2.*cos(THE_Phi_pend).*cos(THE_Theta_pend).*4.0+Lz_pend.*Tv_Z_pend.*cos(THE_Phi_pend).*cos(THE_Psi_pend).*6.0+Lz_pend.*Tv_Z_pend.*sin(THE_Phi_pend).*sin(THE_Psi_pend).*sin(THE_Theta_pend).*6.0))./1.2e+1];
mt31 = [Lz_pend.*m_pend.*(-cos(THE_Psi).*cos(THE_Phi_pend).*cos(THE_Psi_pend).*sin(THE_Phi)-cos(THE_Phi).*cos(THE_Theta).*cos(THE_Psi_pend).*sin(THE_Phi_pend)+cos(THE_Theta_pend).*sin(THE_Phi).*sin(THE_Psi).*sin(THE_Psi_pend)+cos(THE_Phi).*cos(THE_Phi_pend).*cos(THE_Psi_pend).*sin(THE_Psi).*sin(THE_Theta)+cos(THE_Phi).*cos(THE_Psi).*cos(THE_Theta_pend).*sin(THE_Theta).*sin(THE_Psi_pend)+cos(THE_Phi).*cos(THE_Theta).*cos(THE_Phi_pend).*sin(THE_Psi_pend).*sin(THE_Theta_pend)-cos(THE_Psi).*sin(THE_Phi).*sin(THE_Phi_pend).*sin(THE_Psi_pend).*sin(THE_Theta_pend)+cos(THE_Phi).*sin(THE_Psi).*sin(THE_Theta).*sin(THE_Phi_pend).*sin(THE_Psi_pend).*sin(THE_Theta_pend)).*(-1.0./2.0),Lz_pend.*m_pend.*(cos(THE_Phi).*cos(THE_Psi).*cos(THE_Phi_pend).*cos(THE_Psi_pend)-cos(THE_Theta).*cos(THE_Psi_pend).*sin(THE_Phi).*sin(THE_Phi_pend)-cos(THE_Phi).*cos(THE_Theta_pend).*sin(THE_Psi).*sin(THE_Psi_pend)+cos(THE_Phi_pend).*cos(THE_Psi_pend).*sin(THE_Phi).*sin(THE_Psi).*sin(THE_Theta)+cos(THE_Psi).*cos(THE_Theta_pend).*sin(THE_Phi).*sin(THE_Theta).*sin(THE_Psi_pend)+cos(THE_Phi).*cos(THE_Psi).*sin(THE_Phi_pend).*sin(THE_Psi_pend).*sin(THE_Theta_pend)+cos(THE_Theta).*cos(THE_Phi_pend).*sin(THE_Phi).*sin(THE_Psi_pend).*sin(THE_Theta_pend)+sin(THE_Phi).*sin(THE_Psi).*sin(THE_Theta).*sin(THE_Phi_pend).*sin(THE_Psi_pend).*sin(THE_Theta_pend)).*(-1.0./2.0)];
mt32 = [Lz_pend.*m_pend.*(cos(THE_Psi_pend).*sin(THE_Theta).*sin(THE_Phi_pend)+cos(THE_Theta).*cos(THE_Phi_pend).*cos(THE_Psi_pend).*sin(THE_Psi)+cos(THE_Psi).*cos(THE_Theta).*cos(THE_Theta_pend).*sin(THE_Psi_pend)-cos(THE_Phi_pend).*sin(THE_Theta).*sin(THE_Psi_pend).*sin(THE_Theta_pend)+cos(THE_Theta).*sin(THE_Psi).*sin(THE_Phi_pend).*sin(THE_Psi_pend).*sin(THE_Theta_pend)).*(-1.0./2.0),m_pend.*sin(THE_Theta_pend).*(Ly_pend.^2+Lz_pend.^2.*4.0).*(-1.0./1.2e+1),0.0,(m_pend.*(Ly_pend.^2+Lz_pend.^2.*4.0))./1.2e+1];
M = reshape([mt1,mt2,mt3,mt4,mt5,mt6,mt7,mt8,mt9,mt10,mt11,mt12,mt13,mt14,mt15,mt16,mt17,mt18,mt19,mt20,mt21,mt22,mt23,mt24,mt25,mt26,mt27,mt28,mt29,mt30,mt31,mt32],9,9);
if nargout > 1
    et59 = Ly_pend.^2.*THE_Phi_D.*m_pend.*sin(THE_Psi_pend.*2.0).*(-1.0./2.4e+1)+(Lz_pend.^2.*THE_Phi_D.*m_pend.*sin(THE_Psi_pend.*2.0))./6.0+(Ly_pend.^2.*THE_Psi_D.*m_pend.*cos(THE_Theta).*sin(THE_Psi).*sin(THE_Theta_pend))./6.0+(Ly_pend.^2.*THE_Psi_D.*m_pend.*cos(THE_Psi_pend).*sin(THE_Theta).*sin(THE_Psi_pend))./6.0+(Ly_pend.^2.*THE_Phi_D.*m_pend.*cos(THE_Phi_pend).*sin(THE_Phi_pend).*sin(THE_Theta_pend))./1.2e+1+(Ly_pend.^2.*THE_Theta_pend_D.*m_pend.*cos(THE_Phi_pend).*sin(THE_Theta).*sin(THE_Theta_pend))./6.0+Lz_pend.^2.*THE_Theta_D.*m_pend.*cos(THE_Psi).*sin(THE_Theta).*sin(THE_Theta_pend).*(2.0./3.0)-Lz_pend.^2.*THE_Psi_D.*m_pend.*cos(THE_Psi_pend).*sin(THE_Theta).*sin(THE_Psi_pend).*(2.0./3.0)-(Lz_pend.^2.*THE_Phi_D.*m_pend.*cos(THE_Phi_pend).*sin(THE_Phi_pend).*sin(THE_Theta_pend))./3.0+Lz_pend.^2.*THE_Phi_pend_D.*m_pend.*cos(THE_Theta_pend).*sin(THE_Theta).*sin(THE_Phi_pend).*(2.0./3.0)+(Lz_pend.*THE_Phi_D.*Tv_Z_pend.*m_pend.*cos(THE_Theta_pend).*sin(THE_Psi_pend))./2.0+(Ly_pend.^2.*THE_Phi_D.*m_pend.*cos(THE_Theta).^2.*cos(THE_Psi_pend).*sin(THE_Psi_pend))./6.0+(Ly_pend.^2.*THE_Phi_D.*m_pend.*cos(THE_Phi_pend).^2.*cos(THE_Psi_pend).*sin(THE_Psi_pend))./6.0;
    et60 = Lz_pend.^2.*THE_Phi_D.*m_pend.*cos(THE_Theta).^2.*cos(THE_Psi_pend).*sin(THE_Psi_pend).*(-2.0./3.0)-Lz_pend.^2.*THE_Phi_D.*m_pend.*cos(THE_Phi_pend).^2.*cos(THE_Psi_pend).*sin(THE_Psi_pend).*(2.0./3.0)-(Ly_pend.^2.*THE_Theta_pend_D.*m_pend.*cos(THE_Psi).*cos(THE_Theta).*cos(THE_Theta_pend))./6.0-Lz_pend.^2.*THE_Theta_D.*m_pend.*cos(THE_Theta).*cos(THE_Phi_pend).*cos(THE_Theta_pend).*(2.0./3.0)-Lz_pend.*THE_Psi_D.*Tv_Z_pend.*m_pend.*cos(THE_Theta_pend).*sin(THE_Theta).*sin(THE_Psi_pend)-(Ly_pend.^2.*THE_Theta_D.*m_pend.*cos(THE_Psi).^2.*cos(THE_Theta).*cos(THE_Phi_pend).*cos(THE_Theta_pend))./6.0-(Ly_pend.^2.*THE_Theta_D.*m_pend.*cos(THE_Theta).*cos(THE_Phi_pend).*cos(THE_Psi_pend).^2.*cos(THE_Theta_pend))./6.0+(Ly_pend.^2.*THE_Theta_pend_D.*m_pend.*cos(THE_Psi).*cos(THE_Theta).*cos(THE_Psi_pend).^2.*cos(THE_Theta_pend))./6.0+Lz_pend.^2.*THE_Theta_D.*m_pend.*cos(THE_Psi).^2.*cos(THE_Theta).*cos(THE_Phi_pend).*cos(THE_Theta_pend).*(2.0./3.0)+Lz_pend.^2.*THE_Theta_D.*m_pend.*cos(THE_Theta).*cos(THE_Phi_pend).*cos(THE_Psi_pend).^2.*cos(THE_Theta_pend).*(2.0./3.0)-Lz_pend.^2.*THE_Theta_pend_D.*m_pend.*cos(THE_Psi).*cos(THE_Theta).*cos(THE_Psi_pend).^2.*cos(THE_Theta_pend).*(2.0./3.0);
    et61 = Ly_pend.^2.*THE_Psi_D.*m_pend.*cos(THE_Theta).*cos(THE_Phi_pend).^2.*sin(THE_Psi).*sin(THE_Theta_pend).*(-1.0./6.0)-(Ly_pend.^2.*THE_Psi_D.*m_pend.*cos(THE_Theta).*cos(THE_Psi_pend).^2.*sin(THE_Psi).*sin(THE_Theta_pend))./6.0+(Ly_pend.^2.*THE_Theta_D.*m_pend.*cos(THE_Psi).*cos(THE_Phi_pend).^2.*sin(THE_Theta).*sin(THE_Theta_pend))./6.0+(Ly_pend.^2.*THE_Theta_D.*m_pend.*cos(THE_Psi).*cos(THE_Psi_pend).^2.*sin(THE_Theta).*sin(THE_Theta_pend))./6.0-(Ly_pend.^2.*THE_Psi_D.*m_pend.*cos(THE_Phi_pend).^2.*cos(THE_Psi_pend).*sin(THE_Theta).*sin(THE_Psi_pend))./3.0-(Ly_pend.^2.*THE_Phi_D.*m_pend.*cos(THE_Theta).^2.*cos(THE_Phi_pend).*sin(THE_Phi_pend).*sin(THE_Theta_pend))./6.0-(Ly_pend.^2.*THE_Phi_D.*m_pend.*cos(THE_Phi_pend).*cos(THE_Psi_pend).^2.*sin(THE_Phi_pend).*sin(THE_Theta_pend))./6.0+(Ly_pend.^2.*THE_Phi_pend_D.*m_pend.*cos(THE_Psi_pend).^2.*cos(THE_Theta_pend).*sin(THE_Theta).*sin(THE_Phi_pend))./6.0-(Ly_pend.^2.*THE_Theta_pend_D.*m_pend.*cos(THE_Phi_pend).*cos(THE_Psi_pend).^2.*sin(THE_Theta).*sin(THE_Theta_pend))./6.0+Lz_pend.^2.*THE_Psi_D.*m_pend.*cos(THE_Theta).*cos(THE_Phi_pend).^2.*sin(THE_Psi).*sin(THE_Theta_pend).*(2.0./3.0);
    et62 = Lz_pend.^2.*THE_Psi_D.*m_pend.*cos(THE_Theta).*cos(THE_Psi_pend).^2.*sin(THE_Psi).*sin(THE_Theta_pend).*(2.0./3.0)-Lz_pend.^2.*THE_Theta_D.*m_pend.*cos(THE_Psi).*cos(THE_Phi_pend).^2.*sin(THE_Theta).*sin(THE_Theta_pend).*(2.0./3.0)-Lz_pend.^2.*THE_Theta_D.*m_pend.*cos(THE_Psi).*cos(THE_Psi_pend).^2.*sin(THE_Theta).*sin(THE_Theta_pend).*(2.0./3.0)+Lz_pend.^2.*THE_Psi_D.*m_pend.*cos(THE_Phi_pend).^2.*cos(THE_Psi_pend).*sin(THE_Theta).*sin(THE_Psi_pend).*(4.0./3.0)+Lz_pend.^2.*THE_Phi_D.*m_pend.*cos(THE_Theta).^2.*cos(THE_Phi_pend).*sin(THE_Phi_pend).*sin(THE_Theta_pend).*(2.0./3.0)+Lz_pend.^2.*THE_Phi_D.*m_pend.*cos(THE_Phi_pend).*cos(THE_Psi_pend).^2.*sin(THE_Phi_pend).*sin(THE_Theta_pend).*(2.0./3.0)-Lz_pend.^2.*THE_Phi_pend_D.*m_pend.*cos(THE_Psi_pend).^2.*cos(THE_Theta_pend).*sin(THE_Theta).*sin(THE_Phi_pend).*(2.0./3.0)+Lz_pend.^2.*THE_Theta_pend_D.*m_pend.*cos(THE_Phi_pend).*cos(THE_Psi_pend).^2.*sin(THE_Theta).*sin(THE_Theta_pend).*(2.0./3.0)-(Ly_pend.^2.*THE_Phi_D.*m_pend.*cos(THE_Psi).^2.*cos(THE_Theta).^2.*cos(THE_Psi_pend).*sin(THE_Psi_pend))./1.2e+1-(Ly_pend.^2.*THE_Phi_D.*m_pend.*cos(THE_Theta).^2.*cos(THE_Phi_pend).^2.*cos(THE_Psi_pend).*sin(THE_Psi_pend))./3.0;
    et63 = Ly_pend.^2.*THE_Phi_D.*m_pend.*cos(THE_Theta).^2.*cos(THE_Psi_pend).*cos(THE_Theta_pend).^2.*sin(THE_Psi_pend).*(-1.0./1.2e+1)-(Ly_pend.^2.*THE_Phi_D.*m_pend.*cos(THE_Phi_pend).^2.*cos(THE_Psi_pend).*cos(THE_Theta_pend).^2.*sin(THE_Psi_pend))./1.2e+1+(Lz_pend.^2.*THE_Phi_D.*m_pend.*cos(THE_Psi).^2.*cos(THE_Theta).^2.*cos(THE_Psi_pend).*sin(THE_Psi_pend))./3.0+Lz_pend.^2.*THE_Phi_D.*m_pend.*cos(THE_Theta).^2.*cos(THE_Phi_pend).^2.*cos(THE_Psi_pend).*sin(THE_Psi_pend).*(4.0./3.0)+(Lz_pend.^2.*THE_Phi_D.*m_pend.*cos(THE_Theta).^2.*cos(THE_Psi_pend).*cos(THE_Theta_pend).^2.*sin(THE_Psi_pend))./3.0+(Lz_pend.^2.*THE_Phi_D.*m_pend.*cos(THE_Phi_pend).^2.*cos(THE_Psi_pend).*cos(THE_Theta_pend).^2.*sin(THE_Psi_pend))./3.0+(Ly_pend.^2.*THE_Psi_D.*m_pend.*cos(THE_Psi).*cos(THE_Theta).*cos(THE_Theta_pend).*sin(THE_Phi_pend))./6.0+Lz_pend.^2.*THE_Phi_pend_D.*m_pend.*cos(THE_Theta).*cos(THE_Phi_pend).*cos(THE_Theta_pend).*sin(THE_Psi).*(2.0./3.0)-(Ly_pend.^2.*THE_Phi_D.*m_pend.*cos(THE_Theta).*sin(THE_Psi).*sin(THE_Theta).*sin(THE_Theta_pend))./1.2e+1;
    et64 = Ly_pend.^2.*THE_Psi_D.*m_pend.*cos(THE_Phi_pend).*sin(THE_Theta).*sin(THE_Phi_pend).*sin(THE_Theta_pend).*(-1.0./6.0)-(Ly_pend.^2.*THE_Theta_pend_D.*m_pend.*cos(THE_Theta).*sin(THE_Psi).*sin(THE_Phi_pend).*sin(THE_Theta_pend))./6.0-(Ly_pend.^2.*THE_Theta_pend_D.*m_pend.*cos(THE_Psi_pend).*sin(THE_Theta).*sin(THE_Phi_pend).*sin(THE_Psi_pend))./6.0+(Lz_pend.^2.*THE_Phi_D.*m_pend.*cos(THE_Theta).*sin(THE_Psi).*sin(THE_Theta).*sin(THE_Theta_pend))./3.0-Lz_pend.^2.*THE_Theta_D.*m_pend.*cos(THE_Theta_pend).*sin(THE_Psi).*sin(THE_Theta).*sin(THE_Phi_pend).*(2.0./3.0)+Lz_pend.^2.*THE_Psi_D.*m_pend.*cos(THE_Phi_pend).*sin(THE_Theta).*sin(THE_Phi_pend).*sin(THE_Theta_pend).*(2.0./3.0)+Lz_pend.^2.*THE_Theta_pend_D.*m_pend.*cos(THE_Psi_pend).*sin(THE_Theta).*sin(THE_Phi_pend).*sin(THE_Psi_pend).*(2.0./3.0)-Lz_pend.*THE_Theta_D.*Tv_Z_pend.*m_pend.*cos(THE_Psi).^2.*cos(THE_Theta).*cos(THE_Phi_pend).*cos(THE_Psi_pend)+(Ly_pend.^2.*THE_Theta_D.*m_pend.*cos(THE_Psi).^2.*cos(THE_Theta).*cos(THE_Phi_pend).*cos(THE_Psi_pend).^2.*cos(THE_Theta_pend))./3.0-Lz_pend.^2.*THE_Theta_D.*m_pend.*cos(THE_Psi).^2.*cos(THE_Theta).*cos(THE_Phi_pend).*cos(THE_Psi_pend).^2.*cos(THE_Theta_pend).*(4.0./3.0);
    et65 = (Ly_pend.^2.*THE_Phi_D.*m_pend.*cos(THE_Psi).^2.*cos(THE_Theta).^2.*cos(THE_Phi_pend).*sin(THE_Phi_pend).*sin(THE_Theta_pend))./1.2e+1+(Ly_pend.^2.*THE_Psi_D.*m_pend.*cos(THE_Theta).*cos(THE_Phi_pend).^2.*cos(THE_Psi_pend).^2.*sin(THE_Psi).*sin(THE_Theta_pend))./3.0-(Ly_pend.^2.*THE_Theta_D.*m_pend.*cos(THE_Psi).*cos(THE_Phi_pend).^2.*cos(THE_Psi_pend).^2.*sin(THE_Theta).*sin(THE_Theta_pend))./3.0+(Ly_pend.^2.*THE_Phi_D.*m_pend.*cos(THE_Theta).^2.*cos(THE_Phi_pend).*cos(THE_Psi_pend).^2.*sin(THE_Phi_pend).*sin(THE_Theta_pend))./3.0+(Ly_pend.^2.*THE_Psi_D.*m_pend.*cos(THE_Phi_pend).^2.*cos(THE_Psi_pend).*cos(THE_Theta_pend).^2.*sin(THE_Theta).*sin(THE_Psi_pend))./6.0-(Lz_pend.^2.*THE_Phi_D.*m_pend.*cos(THE_Psi).^2.*cos(THE_Theta).^2.*cos(THE_Phi_pend).*sin(THE_Phi_pend).*sin(THE_Theta_pend))./3.0-Lz_pend.^2.*THE_Psi_D.*m_pend.*cos(THE_Theta).*cos(THE_Phi_pend).^2.*cos(THE_Psi_pend).^2.*sin(THE_Psi).*sin(THE_Theta_pend).*(4.0./3.0)+Lz_pend.^2.*THE_Theta_D.*m_pend.*cos(THE_Psi).*cos(THE_Phi_pend).^2.*cos(THE_Psi_pend).^2.*sin(THE_Theta).*sin(THE_Theta_pend).*(4.0./3.0);
    et66 = Lz_pend.^2.*THE_Phi_D.*m_pend.*cos(THE_Theta).^2.*cos(THE_Phi_pend).*cos(THE_Psi_pend).^2.*sin(THE_Phi_pend).*sin(THE_Theta_pend).*(-4.0./3.0)-Lz_pend.^2.*THE_Psi_D.*m_pend.*cos(THE_Phi_pend).^2.*cos(THE_Psi_pend).*cos(THE_Theta_pend).^2.*sin(THE_Theta).*sin(THE_Psi_pend).*(2.0./3.0)-(Lz_pend.*THE_Phi_D.*Tv_Z_pend.*m_pend.*cos(THE_Psi).^2.*cos(THE_Theta).^2.*cos(THE_Theta_pend).*sin(THE_Psi_pend))./2.0+(Ly_pend.^2.*THE_Theta_D.*m_pend.*cos(THE_Psi).*cos(THE_Theta).*cos(THE_Psi_pend).*sin(THE_Psi).*sin(THE_Psi_pend))./6.0-(Ly_pend.^2.*THE_Phi_D.*m_pend.*cos(THE_Psi).*cos(THE_Theta).*cos(THE_Theta_pend).*sin(THE_Theta).*sin(THE_Phi_pend))./1.2e+1-(Ly_pend.^2.*THE_Theta_pend_D.*m_pend.*cos(THE_Theta).*cos(THE_Phi_pend).*cos(THE_Psi_pend).*sin(THE_Psi).*sin(THE_Psi_pend))./6.0-Lz_pend.^2.*THE_Theta_D.*m_pend.*cos(THE_Psi).*cos(THE_Theta).*cos(THE_Psi_pend).*sin(THE_Psi).*sin(THE_Psi_pend).*(2.0./3.0)+(Lz_pend.^2.*THE_Phi_D.*m_pend.*cos(THE_Psi).*cos(THE_Theta).*cos(THE_Theta_pend).*sin(THE_Theta).*sin(THE_Phi_pend))./3.0+Lz_pend.^2.*THE_Theta_pend_D.*m_pend.*cos(THE_Theta).*cos(THE_Phi_pend).*cos(THE_Psi_pend).*sin(THE_Psi).*sin(THE_Psi_pend).*(2.0./3.0);
    et67 = (Ly_pend.^2.*THE_Phi_D.*m_pend.*cos(THE_Psi).^2.*cos(THE_Theta).^2.*cos(THE_Phi_pend).^2.*cos(THE_Psi_pend).*sin(THE_Psi_pend))./6.0+(Ly_pend.^2.*THE_Phi_D.*m_pend.*cos(THE_Psi).^2.*cos(THE_Theta).^2.*cos(THE_Psi_pend).*cos(THE_Theta_pend).^2.*sin(THE_Psi_pend))./6.0+(Ly_pend.^2.*THE_Phi_D.*m_pend.*cos(THE_Theta).^2.*cos(THE_Phi_pend).^2.*cos(THE_Psi_pend).*cos(THE_Theta_pend).^2.*sin(THE_Psi_pend))./6.0-Lz_pend.^2.*THE_Phi_D.*m_pend.*cos(THE_Psi).^2.*cos(THE_Theta).^2.*cos(THE_Phi_pend).^2.*cos(THE_Psi_pend).*sin(THE_Psi_pend).*(2.0./3.0)-Lz_pend.^2.*THE_Phi_D.*m_pend.*cos(THE_Psi).^2.*cos(THE_Theta).^2.*cos(THE_Psi_pend).*cos(THE_Theta_pend).^2.*sin(THE_Psi_pend).*(2.0./3.0)-Lz_pend.^2.*THE_Phi_D.*m_pend.*cos(THE_Theta).^2.*cos(THE_Phi_pend).^2.*cos(THE_Psi_pend).*cos(THE_Theta_pend).^2.*sin(THE_Psi_pend).*(2.0./3.0)+Lz_pend.*THE_Psi_D.*Tv_Z_pend.*m_pend.*cos(THE_Psi).*cos(THE_Theta).*cos(THE_Psi_pend).*sin(THE_Phi_pend)-(Ly_pend.^2.*THE_Phi_D.*m_pend.*cos(THE_Psi).*cos(THE_Theta).^2.*cos(THE_Phi_pend).*cos(THE_Theta_pend).*sin(THE_Psi))./1.2e+1;
    et68 = Ly_pend.^2.*THE_Psi_D.*m_pend.*cos(THE_Psi).*cos(THE_Theta).*cos(THE_Psi_pend).^2.*cos(THE_Theta_pend).*sin(THE_Phi_pend).*(-1.0./6.0)+(Ly_pend.^2.*THE_Phi_pend_D.*m_pend.*cos(THE_Theta).*cos(THE_Phi_pend).*cos(THE_Psi_pend).^2.*cos(THE_Theta_pend).*sin(THE_Psi))./6.0+(Ly_pend.^2.*THE_Phi_pend_D.*m_pend.*cos(THE_Psi).*cos(THE_Theta).*cos(THE_Psi_pend).*cos(THE_Theta_pend).^2.*sin(THE_Psi_pend))./6.0+(Lz_pend.^2.*THE_Phi_D.*m_pend.*cos(THE_Psi).*cos(THE_Theta).^2.*cos(THE_Phi_pend).*cos(THE_Theta_pend).*sin(THE_Psi))./3.0+Lz_pend.^2.*THE_Psi_D.*m_pend.*cos(THE_Psi).*cos(THE_Theta).*cos(THE_Psi_pend).^2.*cos(THE_Theta_pend).*sin(THE_Phi_pend).*(2.0./3.0)-Lz_pend.^2.*THE_Phi_pend_D.*m_pend.*cos(THE_Theta).*cos(THE_Phi_pend).*cos(THE_Psi_pend).^2.*cos(THE_Theta_pend).*sin(THE_Psi).*(2.0./3.0)-Lz_pend.^2.*THE_Phi_pend_D.*m_pend.*cos(THE_Psi).*cos(THE_Theta).*cos(THE_Psi_pend).*cos(THE_Theta_pend).^2.*sin(THE_Psi_pend).*(2.0./3.0)+(Ly_pend.^2.*THE_Phi_D.*m_pend.*cos(THE_Theta).*cos(THE_Phi_pend).^2.*sin(THE_Psi).*sin(THE_Theta).*sin(THE_Theta_pend))./6.0+(Ly_pend.^2.*THE_Phi_D.*m_pend.*cos(THE_Theta).*cos(THE_Psi_pend).^2.*sin(THE_Psi).*sin(THE_Theta).*sin(THE_Theta_pend))./6.0;
    et69 = Ly_pend.^2.*THE_Theta_D.*m_pend.*cos(THE_Psi_pend).^2.*cos(THE_Theta_pend).*sin(THE_Psi).*sin(THE_Theta).*sin(THE_Phi_pend).*(-1.0./6.0)+(Ly_pend.^2.*THE_Psi_D.*m_pend.*cos(THE_Phi_pend).*cos(THE_Psi_pend).^2.*sin(THE_Theta).*sin(THE_Phi_pend).*sin(THE_Theta_pend))./3.0+(Ly_pend.^2.*THE_Theta_pend_D.*m_pend.*cos(THE_Theta).*cos(THE_Psi_pend).^2.*sin(THE_Psi).*sin(THE_Phi_pend).*sin(THE_Theta_pend))./6.0-Lz_pend.^2.*THE_Phi_D.*m_pend.*cos(THE_Theta).*cos(THE_Phi_pend).^2.*sin(THE_Psi).*sin(THE_Theta).*sin(THE_Theta_pend).*(2.0./3.0)-Lz_pend.^2.*THE_Phi_D.*m_pend.*cos(THE_Theta).*cos(THE_Psi_pend).^2.*sin(THE_Psi).*sin(THE_Theta).*sin(THE_Theta_pend).*(2.0./3.0)+Lz_pend.^2.*THE_Theta_D.*m_pend.*cos(THE_Psi_pend).^2.*cos(THE_Theta_pend).*sin(THE_Psi).*sin(THE_Theta).*sin(THE_Phi_pend).*(2.0./3.0)-Lz_pend.^2.*THE_Psi_D.*m_pend.*cos(THE_Phi_pend).*cos(THE_Psi_pend).^2.*sin(THE_Theta).*sin(THE_Phi_pend).*sin(THE_Theta_pend).*(4.0./3.0)-Lz_pend.^2.*THE_Theta_pend_D.*m_pend.*cos(THE_Theta).*cos(THE_Psi_pend).^2.*sin(THE_Psi).*sin(THE_Phi_pend).*sin(THE_Theta_pend).*(2.0./3.0)-(Ly_pend.^2.*THE_Phi_D.*m_pend.*cos(THE_Theta).*cos(THE_Phi_pend).^2.*cos(THE_Psi_pend).^2.*sin(THE_Psi).*sin(THE_Theta).*sin(THE_Theta_pend))./3.0;
    et70 = Lz_pend.^2.*THE_Phi_D.*m_pend.*cos(THE_Theta).*cos(THE_Phi_pend).^2.*cos(THE_Psi_pend).^2.*sin(THE_Psi).*sin(THE_Theta).*sin(THE_Theta_pend).*(4.0./3.0)-(Ly_pend.^2.*THE_Theta_D.*m_pend.*cos(THE_Psi).*cos(THE_Theta).*cos(THE_Phi_pend).*sin(THE_Psi).*sin(THE_Phi_pend).*sin(THE_Theta_pend))./6.0+(Ly_pend.^2.*THE_Psi_D.*m_pend.*cos(THE_Theta).*cos(THE_Phi_pend).*cos(THE_Psi_pend).*sin(THE_Psi).*sin(THE_Phi_pend).*sin(THE_Psi_pend))./3.0-(Ly_pend.^2.*THE_Theta_D.*m_pend.*cos(THE_Psi).*cos(THE_Phi_pend).*cos(THE_Psi_pend).*sin(THE_Theta).*sin(THE_Phi_pend).*sin(THE_Psi_pend))./3.0-(Ly_pend.^2.*THE_Theta_D.*m_pend.*cos(THE_Theta).*cos(THE_Psi_pend).*cos(THE_Theta_pend).*sin(THE_Phi_pend).*sin(THE_Psi_pend).*sin(THE_Theta_pend))./6.0-(Ly_pend.^2.*THE_Phi_pend_D.*m_pend.*cos(THE_Phi_pend).*cos(THE_Psi_pend).*cos(THE_Theta_pend).*sin(THE_Theta).*sin(THE_Psi_pend).*sin(THE_Theta_pend))./6.0+Lz_pend.^2.*THE_Theta_D.*m_pend.*cos(THE_Psi).*cos(THE_Theta).*cos(THE_Phi_pend).*sin(THE_Psi).*sin(THE_Phi_pend).*sin(THE_Theta_pend).*(2.0./3.0)-Lz_pend.^2.*THE_Psi_D.*m_pend.*cos(THE_Theta).*cos(THE_Phi_pend).*cos(THE_Psi_pend).*sin(THE_Psi).*sin(THE_Phi_pend).*sin(THE_Psi_pend).*(4.0./3.0)+Lz_pend.^2.*THE_Theta_D.*m_pend.*cos(THE_Psi).*cos(THE_Phi_pend).*cos(THE_Psi_pend).*sin(THE_Theta).*sin(THE_Phi_pend).*sin(THE_Psi_pend).*(4.0./3.0);
    et71 = Lz_pend.^2.*THE_Theta_D.*m_pend.*cos(THE_Theta).*cos(THE_Psi_pend).*cos(THE_Theta_pend).*sin(THE_Phi_pend).*sin(THE_Psi_pend).*sin(THE_Theta_pend).*(2.0./3.0)+Lz_pend.^2.*THE_Phi_pend_D.*m_pend.*cos(THE_Phi_pend).*cos(THE_Psi_pend).*cos(THE_Theta_pend).*sin(THE_Theta).*sin(THE_Psi_pend).*sin(THE_Theta_pend).*(2.0./3.0)-(Ly_pend.^2.*THE_Phi_D.*m_pend.*cos(THE_Psi).^2.*cos(THE_Theta).^2.*cos(THE_Phi_pend).*cos(THE_Psi_pend).^2.*sin(THE_Phi_pend).*sin(THE_Theta_pend))./6.0+Lz_pend.^2.*THE_Phi_D.*m_pend.*cos(THE_Psi).^2.*cos(THE_Theta).^2.*cos(THE_Phi_pend).*cos(THE_Psi_pend).^2.*sin(THE_Phi_pend).*sin(THE_Theta_pend).*(2.0./3.0)-(Lz_pend.*THE_Phi_D.*Tv_Z_pend.*m_pend.*cos(THE_Psi).*cos(THE_Theta).*cos(THE_Psi_pend).*sin(THE_Theta).*sin(THE_Phi_pend))./2.0+Lz_pend.*THE_Theta_D.*Tv_Z_pend.*m_pend.*cos(THE_Psi).*cos(THE_Theta).*cos(THE_Theta_pend).*sin(THE_Psi).*sin(THE_Psi_pend)-Lz_pend.*THE_Psi_D.*Tv_Z_pend.*m_pend.*cos(THE_Psi).*cos(THE_Theta).*cos(THE_Phi_pend).*sin(THE_Psi_pend).*sin(THE_Theta_pend)-(Ly_pend.^2.*THE_Theta_D.*m_pend.*cos(THE_Psi).*cos(THE_Theta).*cos(THE_Phi_pend).^2.*cos(THE_Psi_pend).*sin(THE_Psi).*sin(THE_Psi_pend))./3.0+(Ly_pend.^2.*THE_Phi_D.*m_pend.*cos(THE_Psi).*cos(THE_Theta).*cos(THE_Psi_pend).^2.*cos(THE_Theta_pend).*sin(THE_Theta).*sin(THE_Phi_pend))./6.0;
    et72 = Ly_pend.^2.*THE_Theta_D.*m_pend.*cos(THE_Psi).*cos(THE_Theta).*cos(THE_Psi_pend).*cos(THE_Theta_pend).^2.*sin(THE_Psi).*sin(THE_Psi_pend).*(-1.0./3.0)+Lz_pend.^2.*THE_Theta_D.*m_pend.*cos(THE_Psi).*cos(THE_Theta).*cos(THE_Phi_pend).^2.*cos(THE_Psi_pend).*sin(THE_Psi).*sin(THE_Psi_pend).*(4.0./3.0)-Lz_pend.^2.*THE_Phi_D.*m_pend.*cos(THE_Psi).*cos(THE_Theta).*cos(THE_Psi_pend).^2.*cos(THE_Theta_pend).*sin(THE_Theta).*sin(THE_Phi_pend).*(2.0./3.0)+Lz_pend.^2.*THE_Theta_D.*m_pend.*cos(THE_Psi).*cos(THE_Theta).*cos(THE_Psi_pend).*cos(THE_Theta_pend).^2.*sin(THE_Psi).*sin(THE_Psi_pend).*(4.0./3.0)-(Ly_pend.^2.*THE_Phi_D.*m_pend.*cos(THE_Psi).^2.*cos(THE_Theta).^2.*cos(THE_Phi_pend).^2.*cos(THE_Psi_pend).*cos(THE_Theta_pend).^2.*sin(THE_Psi_pend))./1.2e+1+(Lz_pend.^2.*THE_Phi_D.*m_pend.*cos(THE_Psi).^2.*cos(THE_Theta).^2.*cos(THE_Phi_pend).^2.*cos(THE_Psi_pend).*cos(THE_Theta_pend).^2.*sin(THE_Psi_pend))./3.0-(Lz_pend.*THE_Phi_D.*Tv_Z_pend.*m_pend.*cos(THE_Psi).*cos(THE_Theta).^2.*cos(THE_Phi_pend).*cos(THE_Psi_pend).*sin(THE_Psi))./2.0-Lz_pend.*THE_Theta_D.*Tv_Z_pend.*m_pend.*cos(THE_Psi).^2.*cos(THE_Theta).*sin(THE_Phi_pend).*sin(THE_Psi_pend).*sin(THE_Theta_pend);
    et73 = (Ly_pend.^2.*THE_Phi_D.*m_pend.*cos(THE_Psi).*cos(THE_Theta).^2.*cos(THE_Phi_pend).*cos(THE_Psi_pend).^2.*cos(THE_Theta_pend).*sin(THE_Psi))./6.0-Lz_pend.^2.*THE_Phi_D.*m_pend.*cos(THE_Psi).*cos(THE_Theta).^2.*cos(THE_Phi_pend).*cos(THE_Psi_pend).^2.*cos(THE_Theta_pend).*sin(THE_Psi).*(2.0./3.0)-(Ly_pend.^2.*THE_Phi_D.*m_pend.*cos(THE_Theta).*cos(THE_Phi_pend).*cos(THE_Psi_pend).*sin(THE_Psi).*sin(THE_Theta).*sin(THE_Phi_pend).*sin(THE_Psi_pend))./3.0+(Ly_pend.^2.*THE_Theta_D.*m_pend.*cos(THE_Phi_pend).*cos(THE_Psi_pend).*cos(THE_Theta_pend).*sin(THE_Psi).*sin(THE_Theta).*sin(THE_Psi_pend).*sin(THE_Theta_pend))./6.0+(Ly_pend.^2.*THE_Phi_pend_D.*m_pend.*cos(THE_Theta).*cos(THE_Psi_pend).*cos(THE_Theta_pend).*sin(THE_Psi).*sin(THE_Phi_pend).*sin(THE_Psi_pend).*sin(THE_Theta_pend))./6.0+Lz_pend.^2.*THE_Phi_D.*m_pend.*cos(THE_Theta).*cos(THE_Phi_pend).*cos(THE_Psi_pend).*sin(THE_Psi).*sin(THE_Theta).*sin(THE_Phi_pend).*sin(THE_Psi_pend).*(4.0./3.0)-Lz_pend.^2.*THE_Theta_D.*m_pend.*cos(THE_Phi_pend).*cos(THE_Psi_pend).*cos(THE_Theta_pend).*sin(THE_Psi).*sin(THE_Theta).*sin(THE_Psi_pend).*sin(THE_Theta_pend).*(2.0./3.0)-Lz_pend.^2.*THE_Phi_pend_D.*m_pend.*cos(THE_Theta).*cos(THE_Psi_pend).*cos(THE_Theta_pend).*sin(THE_Psi).*sin(THE_Phi_pend).*sin(THE_Psi_pend).*sin(THE_Theta_pend).*(2.0./3.0);
    et74 = (Lz_pend.*THE_Phi_D.*Tv_Z_pend.*m_pend.*cos(THE_Psi).*cos(THE_Theta).*cos(THE_Phi_pend).*sin(THE_Theta).*sin(THE_Psi_pend).*sin(THE_Theta_pend))./2.0+(Ly_pend.^2.*THE_Theta_D.*m_pend.*cos(THE_Psi).*cos(THE_Theta).*cos(THE_Phi_pend).*cos(THE_Psi_pend).^2.*sin(THE_Psi).*sin(THE_Phi_pend).*sin(THE_Theta_pend))./3.0-(Ly_pend.^2.*THE_Psi_D.*m_pend.*cos(THE_Theta).*cos(THE_Phi_pend).*cos(THE_Psi_pend).*cos(THE_Theta_pend).^2.*sin(THE_Psi).*sin(THE_Phi_pend).*sin(THE_Psi_pend))./6.0+(Ly_pend.^2.*THE_Theta_D.*m_pend.*cos(THE_Psi).*cos(THE_Phi_pend).*cos(THE_Psi_pend).*cos(THE_Theta_pend).^2.*sin(THE_Theta).*sin(THE_Phi_pend).*sin(THE_Psi_pend))./6.0+(Ly_pend.^2.*THE_Theta_D.*m_pend.*cos(THE_Psi).^2.*cos(THE_Theta).*cos(THE_Psi_pend).*cos(THE_Theta_pend).*sin(THE_Phi_pend).*sin(THE_Psi_pend).*sin(THE_Theta_pend))./3.0-Lz_pend.^2.*THE_Theta_D.*m_pend.*cos(THE_Psi).*cos(THE_Theta).*cos(THE_Phi_pend).*cos(THE_Psi_pend).^2.*sin(THE_Psi).*sin(THE_Phi_pend).*sin(THE_Theta_pend).*(4.0./3.0)+Lz_pend.^2.*THE_Psi_D.*m_pend.*cos(THE_Theta).*cos(THE_Phi_pend).*cos(THE_Psi_pend).*cos(THE_Theta_pend).^2.*sin(THE_Psi).*sin(THE_Phi_pend).*sin(THE_Psi_pend).*(2.0./3.0)-Lz_pend.^2.*THE_Theta_D.*m_pend.*cos(THE_Psi).*cos(THE_Phi_pend).*cos(THE_Psi_pend).*cos(THE_Theta_pend).^2.*sin(THE_Theta).*sin(THE_Phi_pend).*sin(THE_Psi_pend).*(2.0./3.0);
    et75 = Lz_pend.^2.*THE_Theta_D.*m_pend.*cos(THE_Psi).^2.*cos(THE_Theta).*cos(THE_Psi_pend).*cos(THE_Theta_pend).*sin(THE_Phi_pend).*sin(THE_Psi_pend).*sin(THE_Theta_pend).*(-4.0./3.0)-(Lz_pend.*THE_Phi_D.*Tv_Z_pend.*m_pend.*cos(THE_Psi).*cos(THE_Theta).^2.*sin(THE_Psi).*sin(THE_Phi_pend).*sin(THE_Psi_pend).*sin(THE_Theta_pend))./2.0+(Ly_pend.^2.*THE_Theta_D.*m_pend.*cos(THE_Psi).*cos(THE_Theta).*cos(THE_Phi_pend).^2.*cos(THE_Psi_pend).*cos(THE_Theta_pend).^2.*sin(THE_Psi).*sin(THE_Psi_pend))./6.0-Lz_pend.^2.*THE_Theta_D.*m_pend.*cos(THE_Psi).*cos(THE_Theta).*cos(THE_Phi_pend).^2.*cos(THE_Psi_pend).*cos(THE_Theta_pend).^2.*sin(THE_Psi).*sin(THE_Psi_pend).*(2.0./3.0)+(Ly_pend.^2.*THE_Psi_D.*m_pend.*cos(THE_Psi).*cos(THE_Theta).*cos(THE_Phi_pend).*cos(THE_Psi_pend).*cos(THE_Theta_pend).*sin(THE_Psi_pend).*sin(THE_Theta_pend))./6.0-Lz_pend.^2.*THE_Psi_D.*m_pend.*cos(THE_Psi).*cos(THE_Theta).*cos(THE_Phi_pend).*cos(THE_Psi_pend).*cos(THE_Theta_pend).*sin(THE_Psi_pend).*sin(THE_Theta_pend).*(2.0./3.0)+(Ly_pend.^2.*THE_Phi_D.*m_pend.*cos(THE_Theta).*cos(THE_Phi_pend).*cos(THE_Psi_pend).*cos(THE_Theta_pend).^2.*sin(THE_Psi).*sin(THE_Theta).*sin(THE_Phi_pend).*sin(THE_Psi_pend))./6.0;
    et76 = (Ly_pend.^2.*THE_Phi_D.*m_pend.*cos(THE_Psi).*cos(THE_Theta).^2.*cos(THE_Psi_pend).*cos(THE_Theta_pend).*sin(THE_Psi).*sin(THE_Phi_pend).*sin(THE_Psi_pend).*sin(THE_Theta_pend))./6.0-Lz_pend.^2.*THE_Phi_D.*m_pend.*cos(THE_Theta).*cos(THE_Phi_pend).*cos(THE_Psi_pend).*cos(THE_Theta_pend).^2.*sin(THE_Psi).*sin(THE_Theta).*sin(THE_Phi_pend).*sin(THE_Psi_pend).*(2.0./3.0)-Lz_pend.^2.*THE_Phi_D.*m_pend.*cos(THE_Psi).*cos(THE_Theta).^2.*cos(THE_Psi_pend).*cos(THE_Theta_pend).*sin(THE_Psi).*sin(THE_Phi_pend).*sin(THE_Psi_pend).*sin(THE_Theta_pend).*(2.0./3.0)-(Ly_pend.^2.*THE_Phi_D.*m_pend.*cos(THE_Psi).*cos(THE_Theta).*cos(THE_Phi_pend).*cos(THE_Psi_pend).*cos(THE_Theta_pend).*sin(THE_Theta).*sin(THE_Psi_pend).*sin(THE_Theta_pend))./6.0+Lz_pend.^2.*THE_Phi_D.*m_pend.*cos(THE_Psi).*cos(THE_Theta).*cos(THE_Phi_pend).*cos(THE_Psi_pend).*cos(THE_Theta_pend).*sin(THE_Theta).*sin(THE_Psi_pend).*sin(THE_Theta_pend).*(2.0./3.0);
    et77 = (Ly_pend.^2.*THE_Theta_D.*m_pend.*cos(THE_Theta).*sin(THE_Phi_pend))./6.0+(Ly_pend.^2.*THE_Phi_pend_D.*m_pend.*cos(THE_Phi_pend).*sin(THE_Theta))./6.0-(Ly_pend.^2.*THE_Theta_D.*m_pend.*cos(THE_Phi_pend).*sin(THE_Psi).*sin(THE_Theta))./6.0-(Ly_pend.^2.*THE_Phi_pend_D.*m_pend.*cos(THE_Theta).*sin(THE_Psi).*sin(THE_Phi_pend))./6.0-(Ly_pend.^2.*THE_Psi_pend_D.*m_pend.*cos(THE_Phi_pend).*sin(THE_Theta).*sin(THE_Theta_pend))./6.0+(Lz_pend.*THE_Phi_D.*Tv_Z_pend.*m_pend.*cos(THE_Psi_pend).*sin(THE_Theta_pend))./2.0+(Lx_pend.^2.*THE_Theta_D.*m_pend.*cos(THE_Psi).^2.*cos(THE_Theta).*sin(THE_Phi_pend))./6.0-(Lx_pend.^2.*THE_Phi_D.*m_pend.*cos(THE_Theta).^2.*cos(THE_Theta_pend).*sin(THE_Theta_pend))./1.2e+1+(Lx_pend.^2.*THE_Theta_D.*m_pend.*cos(THE_Theta).*cos(THE_Theta_pend).^2.*sin(THE_Phi_pend))./6.0-(Lx_pend.^2.*THE_Phi_D.*m_pend.*cos(THE_Phi_pend).^2.*cos(THE_Theta_pend).*sin(THE_Theta_pend))./1.2e+1+(Lx_pend.^2.*THE_Phi_pend_D.*m_pend.*cos(THE_Phi_pend).*cos(THE_Theta_pend).^2.*sin(THE_Theta))./6.0-(Ly_pend.^2.*THE_Theta_D.*m_pend.*cos(THE_Psi).^2.*cos(THE_Theta).*sin(THE_Phi_pend))./6.0;
    et78 = Ly_pend.^2.*THE_Theta_D.*m_pend.*cos(THE_Theta).*cos(THE_Psi_pend).^2.*sin(THE_Phi_pend).*(-1.0./6.0)+(Ly_pend.^2.*THE_Phi_D.*m_pend.*cos(THE_Theta).^2.*cos(THE_Theta_pend).*sin(THE_Theta_pend))./1.2e+1-(Ly_pend.^2.*THE_Theta_D.*m_pend.*cos(THE_Theta).*cos(THE_Theta_pend).^2.*sin(THE_Phi_pend))./6.0-(Ly_pend.^2.*THE_Phi_pend_D.*m_pend.*cos(THE_Phi_pend).*cos(THE_Psi_pend).^2.*sin(THE_Theta))./6.0+(Ly_pend.^2.*THE_Phi_D.*m_pend.*cos(THE_Phi_pend).^2.*cos(THE_Theta_pend).*sin(THE_Theta_pend))./1.2e+1-(Ly_pend.^2.*THE_Phi_pend_D.*m_pend.*cos(THE_Phi_pend).*cos(THE_Theta_pend).^2.*sin(THE_Theta))./6.0+Lz_pend.^2.*THE_Theta_D.*m_pend.*cos(THE_Theta).*cos(THE_Psi_pend).^2.*sin(THE_Phi_pend).*(2.0./3.0)+Lz_pend.^2.*THE_Phi_pend_D.*m_pend.*cos(THE_Phi_pend).*cos(THE_Psi_pend).^2.*sin(THE_Theta).*(2.0./3.0)+(Lx_pend.^2.*THE_Psi_D.*m_pend.*cos(THE_Psi).*cos(THE_Theta).*cos(THE_Phi_pend))./6.0+(Ly_pend.^2.*THE_Psi_pend_D.*m_pend.*cos(THE_Psi).*cos(THE_Theta).*cos(THE_Theta_pend))./6.0-Lz_pend.*THE_Psi_D.*Tv_Z_pend.*m_pend.*cos(THE_Psi_pend).*sin(THE_Theta).*sin(THE_Theta_pend);
    et79 = Lx_pend.^2.*THE_Psi_D.*m_pend.*cos(THE_Psi).*cos(THE_Theta).*cos(THE_Phi_pend).*cos(THE_Theta_pend).^2.*(-1.0./6.0)+(Ly_pend.^2.*THE_Psi_D.*m_pend.*cos(THE_Psi).*cos(THE_Theta).*cos(THE_Phi_pend).*cos(THE_Theta_pend).^2)./6.0-(Ly_pend.^2.*THE_Psi_pend_D.*m_pend.*cos(THE_Psi).*cos(THE_Theta).*cos(THE_Psi_pend).^2.*cos(THE_Theta_pend))./6.0+Lz_pend.^2.*THE_Psi_pend_D.*m_pend.*cos(THE_Psi).*cos(THE_Theta).*cos(THE_Psi_pend).^2.*cos(THE_Theta_pend).*(2.0./3.0)+(Lx_pend.^2.*THE_Phi_D.*m_pend.*cos(THE_Psi).*cos(THE_Theta).^2.*sin(THE_Psi).*sin(THE_Phi_pend))./1.2e+1-(Lx_pend.^2.*THE_Theta_D.*m_pend.*cos(THE_Phi_pend).*cos(THE_Theta_pend).^2.*sin(THE_Psi).*sin(THE_Theta))./6.0-(Lx_pend.^2.*THE_Phi_pend_D.*m_pend.*cos(THE_Theta).*cos(THE_Theta_pend).^2.*sin(THE_Psi).*sin(THE_Phi_pend))./6.0+(Lx_pend.^2.*THE_Psi_D.*m_pend.*cos(THE_Phi_pend).^2.*cos(THE_Theta_pend).*sin(THE_Theta).*sin(THE_Theta_pend))./6.0-(Ly_pend.^2.*THE_Phi_D.*m_pend.*cos(THE_Psi).*cos(THE_Theta).^2.*sin(THE_Psi).*sin(THE_Phi_pend))./1.2e+1+(Ly_pend.^2.*THE_Theta_D.*m_pend.*cos(THE_Phi_pend).*cos(THE_Psi_pend).^2.*sin(THE_Psi).*sin(THE_Theta))./6.0;
    et80 = (Ly_pend.^2.*THE_Theta_D.*m_pend.*cos(THE_Phi_pend).*cos(THE_Theta_pend).^2.*sin(THE_Psi).*sin(THE_Theta))./6.0+(Ly_pend.^2.*THE_Phi_pend_D.*m_pend.*cos(THE_Theta).*cos(THE_Psi_pend).^2.*sin(THE_Psi).*sin(THE_Phi_pend))./6.0+(Ly_pend.^2.*THE_Phi_pend_D.*m_pend.*cos(THE_Theta).*cos(THE_Theta_pend).^2.*sin(THE_Psi).*sin(THE_Phi_pend))./6.0-(Ly_pend.^2.*THE_Psi_D.*m_pend.*cos(THE_Phi_pend).^2.*cos(THE_Theta_pend).*sin(THE_Theta).*sin(THE_Theta_pend))./6.0+(Ly_pend.^2.*THE_Psi_pend_D.*m_pend.*cos(THE_Phi_pend).*cos(THE_Psi_pend).^2.*sin(THE_Theta).*sin(THE_Theta_pend))./6.0-Lz_pend.^2.*THE_Theta_D.*m_pend.*cos(THE_Phi_pend).*cos(THE_Psi_pend).^2.*sin(THE_Psi).*sin(THE_Theta).*(2.0./3.0)-Lz_pend.^2.*THE_Phi_pend_D.*m_pend.*cos(THE_Theta).*cos(THE_Psi_pend).^2.*sin(THE_Psi).*sin(THE_Phi_pend).*(2.0./3.0)-Lz_pend.^2.*THE_Psi_pend_D.*m_pend.*cos(THE_Phi_pend).*cos(THE_Psi_pend).^2.*sin(THE_Theta).*sin(THE_Theta_pend).*(2.0./3.0)+(Lx_pend.^2.*THE_Phi_D.*m_pend.*cos(THE_Psi).^2.*cos(THE_Theta).^2.*cos(THE_Theta_pend).*sin(THE_Theta_pend))./6.0-(Lx_pend.^2.*THE_Theta_D.*m_pend.*cos(THE_Psi).^2.*cos(THE_Theta).*cos(THE_Theta_pend).^2.*sin(THE_Phi_pend))./3.0;
    et81 = (Lx_pend.^2.*THE_Phi_D.*m_pend.*cos(THE_Theta).^2.*cos(THE_Phi_pend).^2.*cos(THE_Theta_pend).*sin(THE_Theta_pend))./6.0+(Ly_pend.^2.*THE_Theta_D.*m_pend.*cos(THE_Psi).^2.*cos(THE_Theta).*cos(THE_Psi_pend).^2.*sin(THE_Phi_pend))./6.0-(Ly_pend.^2.*THE_Phi_D.*m_pend.*cos(THE_Psi).^2.*cos(THE_Theta).^2.*cos(THE_Theta_pend).*sin(THE_Theta_pend))./6.0+(Ly_pend.^2.*THE_Theta_D.*m_pend.*cos(THE_Psi).^2.*cos(THE_Theta).*cos(THE_Theta_pend).^2.*sin(THE_Phi_pend))./3.0-(Ly_pend.^2.*THE_Phi_D.*m_pend.*cos(THE_Theta).^2.*cos(THE_Phi_pend).^2.*cos(THE_Theta_pend).*sin(THE_Theta_pend))./6.0-(Ly_pend.^2.*THE_Phi_D.*m_pend.*cos(THE_Theta).^2.*cos(THE_Psi_pend).^2.*cos(THE_Theta_pend).*sin(THE_Theta_pend))./1.2e+1+(Ly_pend.^2.*THE_Theta_D.*m_pend.*cos(THE_Theta).*cos(THE_Psi_pend).^2.*cos(THE_Theta_pend).^2.*sin(THE_Phi_pend))./6.0-(Ly_pend.^2.*THE_Phi_D.*m_pend.*cos(THE_Phi_pend).^2.*cos(THE_Psi_pend).^2.*cos(THE_Theta_pend).*sin(THE_Theta_pend))./1.2e+1+(Ly_pend.^2.*THE_Phi_pend_D.*m_pend.*cos(THE_Phi_pend).*cos(THE_Psi_pend).^2.*cos(THE_Theta_pend).^2.*sin(THE_Theta))./6.0;
    et82 = Lz_pend.^2.*THE_Theta_D.*m_pend.*cos(THE_Psi).^2.*cos(THE_Theta).*cos(THE_Psi_pend).^2.*sin(THE_Phi_pend).*(-2.0./3.0)+(Lz_pend.^2.*THE_Phi_D.*m_pend.*cos(THE_Theta).^2.*cos(THE_Psi_pend).^2.*cos(THE_Theta_pend).*sin(THE_Theta_pend))./3.0-Lz_pend.^2.*THE_Theta_D.*m_pend.*cos(THE_Theta).*cos(THE_Psi_pend).^2.*cos(THE_Theta_pend).^2.*sin(THE_Phi_pend).*(2.0./3.0)+(Lz_pend.^2.*THE_Phi_D.*m_pend.*cos(THE_Phi_pend).^2.*cos(THE_Psi_pend).^2.*cos(THE_Theta_pend).*sin(THE_Theta_pend))./3.0-Lz_pend.^2.*THE_Phi_pend_D.*m_pend.*cos(THE_Phi_pend).*cos(THE_Psi_pend).^2.*cos(THE_Theta_pend).^2.*sin(THE_Theta).*(2.0./3.0)-(Lx_pend.^2.*THE_Phi_D.*m_pend.*cos(THE_Psi).*cos(THE_Theta).*cos(THE_Phi_pend).*sin(THE_Theta))./1.2e+1+(Lx_pend.^2.*THE_Phi_pend_D.*m_pend.*cos(THE_Psi).*cos(THE_Theta).*cos(THE_Theta_pend).*sin(THE_Theta_pend))./6.0+(Ly_pend.^2.*THE_Phi_D.*m_pend.*cos(THE_Psi).*cos(THE_Theta).*cos(THE_Phi_pend).*sin(THE_Theta))./1.2e+1-(Ly_pend.^2.*THE_Phi_pend_D.*m_pend.*cos(THE_Psi).*cos(THE_Theta).*cos(THE_Theta_pend).*sin(THE_Theta_pend))./6.0+(Ly_pend.^2.*THE_Psi_pend_D.*m_pend.*cos(THE_Theta).*sin(THE_Psi).*sin(THE_Phi_pend).*sin(THE_Theta_pend))./6.0;
    et83 = (Ly_pend.^2.*THE_Psi_pend_D.*m_pend.*cos(THE_Psi_pend).*sin(THE_Theta).*sin(THE_Phi_pend).*sin(THE_Psi_pend))./6.0-Lz_pend.^2.*THE_Psi_pend_D.*m_pend.*cos(THE_Psi_pend).*sin(THE_Theta).*sin(THE_Phi_pend).*sin(THE_Psi_pend).*(2.0./3.0)-(Ly_pend.^2.*THE_Psi_D.*m_pend.*cos(THE_Psi).*cos(THE_Theta).*cos(THE_Phi_pend).*cos(THE_Psi_pend).^2.*cos(THE_Theta_pend).^2)./6.0+Lz_pend.^2.*THE_Psi_D.*m_pend.*cos(THE_Psi).*cos(THE_Theta).*cos(THE_Phi_pend).*cos(THE_Psi_pend).^2.*cos(THE_Theta_pend).^2.*(2.0./3.0)-(Lx_pend.^2.*THE_Phi_D.*m_pend.*cos(THE_Psi).*cos(THE_Theta).^2.*cos(THE_Theta_pend).^2.*sin(THE_Psi).*sin(THE_Phi_pend))./6.0+(Ly_pend.^2.*THE_Phi_D.*m_pend.*cos(THE_Psi).*cos(THE_Theta).^2.*cos(THE_Psi_pend).^2.*sin(THE_Psi).*sin(THE_Phi_pend))./1.2e+1+(Ly_pend.^2.*THE_Phi_D.*m_pend.*cos(THE_Psi).*cos(THE_Theta).^2.*cos(THE_Theta_pend).^2.*sin(THE_Psi).*sin(THE_Phi_pend))./6.0-(Ly_pend.^2.*THE_Theta_D.*m_pend.*cos(THE_Phi_pend).*cos(THE_Psi_pend).^2.*cos(THE_Theta_pend).^2.*sin(THE_Psi).*sin(THE_Theta))./6.0;
    et84 = Ly_pend.^2.*THE_Phi_pend_D.*m_pend.*cos(THE_Theta).*cos(THE_Psi_pend).^2.*cos(THE_Theta_pend).^2.*sin(THE_Psi).*sin(THE_Phi_pend).*(-1.0./6.0)+(Ly_pend.^2.*THE_Psi_D.*m_pend.*cos(THE_Phi_pend).^2.*cos(THE_Psi_pend).^2.*cos(THE_Theta_pend).*sin(THE_Theta).*sin(THE_Theta_pend))./6.0-(Lz_pend.^2.*THE_Phi_D.*m_pend.*cos(THE_Psi).*cos(THE_Theta).^2.*cos(THE_Psi_pend).^2.*sin(THE_Psi).*sin(THE_Phi_pend))./3.0+Lz_pend.^2.*THE_Theta_D.*m_pend.*cos(THE_Phi_pend).*cos(THE_Psi_pend).^2.*cos(THE_Theta_pend).^2.*sin(THE_Psi).*sin(THE_Theta).*(2.0./3.0)+Lz_pend.^2.*THE_Phi_pend_D.*m_pend.*cos(THE_Theta).*cos(THE_Psi_pend).^2.*cos(THE_Theta_pend).^2.*sin(THE_Psi).*sin(THE_Phi_pend).*(2.0./3.0)-Lz_pend.^2.*THE_Psi_D.*m_pend.*cos(THE_Phi_pend).^2.*cos(THE_Psi_pend).^2.*cos(THE_Theta_pend).*sin(THE_Theta).*sin(THE_Theta_pend).*(2.0./3.0)-(Lz_pend.*THE_Phi_D.*Tv_Z_pend.*m_pend.*cos(THE_Psi).^2.*cos(THE_Theta).^2.*cos(THE_Psi_pend).*sin(THE_Theta_pend))./2.0-(Lx_pend.^2.*THE_Theta_D.*m_pend.*cos(THE_Psi).*cos(THE_Theta).*cos(THE_Theta_pend).*sin(THE_Psi).*sin(THE_Theta_pend))./3.0;
    et85 = (Ly_pend.^2.*THE_Theta_D.*m_pend.*cos(THE_Psi).*cos(THE_Theta).*cos(THE_Theta_pend).*sin(THE_Psi).*sin(THE_Theta_pend))./3.0+(Ly_pend.^2.*THE_Theta_D.*m_pend.*cos(THE_Psi).*cos(THE_Psi_pend).*cos(THE_Theta_pend).*sin(THE_Theta).*sin(THE_Psi_pend))./6.0+(Ly_pend.^2.*THE_Psi_pend_D.*m_pend.*cos(THE_Theta).*cos(THE_Phi_pend).*cos(THE_Psi_pend).*sin(THE_Psi).*sin(THE_Psi_pend))./6.0+(Ly_pend.^2.*THE_Theta_D.*m_pend.*cos(THE_Theta).*cos(THE_Phi_pend).*cos(THE_Psi_pend).*sin(THE_Psi_pend).*sin(THE_Theta_pend))./6.0-(Ly_pend.^2.*THE_Phi_D.*m_pend.*cos(THE_Phi_pend).*cos(THE_Psi_pend).*cos(THE_Theta_pend).*sin(THE_Phi_pend).*sin(THE_Psi_pend))./1.2e+1-Lz_pend.^2.*THE_Theta_D.*m_pend.*cos(THE_Psi).*cos(THE_Psi_pend).*cos(THE_Theta_pend).*sin(THE_Theta).*sin(THE_Psi_pend).*(2.0./3.0)-Lz_pend.^2.*THE_Psi_pend_D.*m_pend.*cos(THE_Theta).*cos(THE_Phi_pend).*cos(THE_Psi_pend).*sin(THE_Psi).*sin(THE_Psi_pend).*(2.0./3.0)-Lz_pend.^2.*THE_Theta_D.*m_pend.*cos(THE_Theta).*cos(THE_Phi_pend).*cos(THE_Psi_pend).*sin(THE_Psi_pend).*sin(THE_Theta_pend).*(2.0./3.0)+(Lz_pend.^2.*THE_Phi_D.*m_pend.*cos(THE_Phi_pend).*cos(THE_Psi_pend).*cos(THE_Theta_pend).*sin(THE_Phi_pend).*sin(THE_Psi_pend))./3.0;
    et86 = Lx_pend.^2.*THE_Phi_D.*m_pend.*cos(THE_Psi).^2.*cos(THE_Theta).^2.*cos(THE_Phi_pend).^2.*cos(THE_Theta_pend).*sin(THE_Theta_pend).*(-1.0./1.2e+1)+(Ly_pend.^2.*THE_Phi_D.*m_pend.*cos(THE_Psi).^2.*cos(THE_Theta).^2.*cos(THE_Phi_pend).^2.*cos(THE_Theta_pend).*sin(THE_Theta_pend))./1.2e+1+(Ly_pend.^2.*THE_Phi_D.*m_pend.*cos(THE_Psi).^2.*cos(THE_Theta).^2.*cos(THE_Psi_pend).^2.*cos(THE_Theta_pend).*sin(THE_Theta_pend))./6.0-(Ly_pend.^2.*THE_Theta_D.*m_pend.*cos(THE_Psi).^2.*cos(THE_Theta).*cos(THE_Psi_pend).^2.*cos(THE_Theta_pend).^2.*sin(THE_Phi_pend))./3.0+(Ly_pend.^2.*THE_Phi_D.*m_pend.*cos(THE_Theta).^2.*cos(THE_Phi_pend).^2.*cos(THE_Psi_pend).^2.*cos(THE_Theta_pend).*sin(THE_Theta_pend))./6.0-Lz_pend.^2.*THE_Phi_D.*m_pend.*cos(THE_Psi).^2.*cos(THE_Theta).^2.*cos(THE_Psi_pend).^2.*cos(THE_Theta_pend).*sin(THE_Theta_pend).*(2.0./3.0)+Lz_pend.^2.*THE_Theta_D.*m_pend.*cos(THE_Psi).^2.*cos(THE_Theta).*cos(THE_Psi_pend).^2.*cos(THE_Theta_pend).^2.*sin(THE_Phi_pend).*(4.0./3.0);
    et87 = Lz_pend.^2.*THE_Phi_D.*m_pend.*cos(THE_Theta).^2.*cos(THE_Phi_pend).^2.*cos(THE_Psi_pend).^2.*cos(THE_Theta_pend).*sin(THE_Theta_pend).*(-2.0./3.0)-(Ly_pend.^2.*THE_Phi_pend_D.*m_pend.*cos(THE_Psi_pend).*sin(THE_Theta).*sin(THE_Phi_pend).*sin(THE_Psi_pend).*sin(THE_Theta_pend))./6.0+Lz_pend.^2.*THE_Phi_pend_D.*m_pend.*cos(THE_Psi_pend).*sin(THE_Theta).*sin(THE_Phi_pend).*sin(THE_Psi_pend).*sin(THE_Theta_pend).*(2.0./3.0)+(Lx_pend.^2.*THE_Phi_D.*m_pend.*cos(THE_Psi).*cos(THE_Theta).*cos(THE_Phi_pend).*cos(THE_Theta_pend).^2.*sin(THE_Theta))./6.0-(Ly_pend.^2.*THE_Phi_D.*m_pend.*cos(THE_Psi).*cos(THE_Theta).*cos(THE_Phi_pend).*cos(THE_Psi_pend).^2.*sin(THE_Theta))./1.2e+1-(Ly_pend.^2.*THE_Phi_D.*m_pend.*cos(THE_Psi).*cos(THE_Theta).*cos(THE_Phi_pend).*cos(THE_Theta_pend).^2.*sin(THE_Theta))./6.0+(Ly_pend.^2.*THE_Phi_pend_D.*m_pend.*cos(THE_Psi).*cos(THE_Theta).*cos(THE_Psi_pend).^2.*cos(THE_Theta_pend).*sin(THE_Theta_pend))./6.0+(Lz_pend.^2.*THE_Phi_D.*m_pend.*cos(THE_Psi).*cos(THE_Theta).*cos(THE_Phi_pend).*cos(THE_Psi_pend).^2.*sin(THE_Theta))./3.0-Lz_pend.^2.*THE_Phi_pend_D.*m_pend.*cos(THE_Psi).*cos(THE_Theta).*cos(THE_Psi_pend).^2.*cos(THE_Theta_pend).*sin(THE_Theta_pend).*(2.0./3.0);
    et88 = Ly_pend.^2.*THE_Psi_pend_D.*m_pend.*cos(THE_Theta).*cos(THE_Psi_pend).^2.*sin(THE_Psi).*sin(THE_Phi_pend).*sin(THE_Theta_pend).*(-1.0./6.0)+Lz_pend.^2.*THE_Psi_pend_D.*m_pend.*cos(THE_Theta).*cos(THE_Psi_pend).^2.*sin(THE_Psi).*sin(THE_Phi_pend).*sin(THE_Theta_pend).*(2.0./3.0)-(Lx_pend.^2.*THE_Psi_D.*m_pend.*cos(THE_Theta).*cos(THE_Phi_pend).*cos(THE_Theta_pend).*sin(THE_Psi).*sin(THE_Phi_pend).*sin(THE_Theta_pend))./6.0+(Lx_pend.^2.*THE_Theta_D.*m_pend.*cos(THE_Psi).*cos(THE_Phi_pend).*cos(THE_Theta_pend).*sin(THE_Theta).*sin(THE_Phi_pend).*sin(THE_Theta_pend))./6.0+(Ly_pend.^2.*THE_Phi_D.*m_pend.*cos(THE_Theta).*cos(THE_Psi_pend).*cos(THE_Theta_pend).*sin(THE_Psi).*sin(THE_Theta).*sin(THE_Psi_pend))./1.2e+1+(Ly_pend.^2.*THE_Psi_D.*m_pend.*cos(THE_Theta).*cos(THE_Phi_pend).*cos(THE_Theta_pend).*sin(THE_Psi).*sin(THE_Phi_pend).*sin(THE_Theta_pend))./6.0-(Ly_pend.^2.*THE_Theta_D.*m_pend.*cos(THE_Psi).*cos(THE_Phi_pend).*cos(THE_Theta_pend).*sin(THE_Theta).*sin(THE_Phi_pend).*sin(THE_Theta_pend))./6.0+(Ly_pend.^2.*THE_Psi_D.*m_pend.*cos(THE_Phi_pend).*cos(THE_Psi_pend).*cos(THE_Theta_pend).*sin(THE_Theta).*sin(THE_Phi_pend).*sin(THE_Psi_pend))./6.0-(Ly_pend.^2.*THE_Phi_pend_D.*m_pend.*cos(THE_Theta).*cos(THE_Phi_pend).*cos(THE_Psi_pend).*sin(THE_Psi).*sin(THE_Psi_pend).*sin(THE_Theta_pend))./6.0;
    et89 = Lz_pend.^2.*THE_Phi_D.*m_pend.*cos(THE_Theta).*cos(THE_Psi_pend).*cos(THE_Theta_pend).*sin(THE_Psi).*sin(THE_Theta).*sin(THE_Psi_pend).*(-1.0./3.0)-Lz_pend.^2.*THE_Psi_D.*m_pend.*cos(THE_Phi_pend).*cos(THE_Psi_pend).*cos(THE_Theta_pend).*sin(THE_Theta).*sin(THE_Phi_pend).*sin(THE_Psi_pend).*(2.0./3.0)+Lz_pend.^2.*THE_Phi_pend_D.*m_pend.*cos(THE_Theta).*cos(THE_Phi_pend).*cos(THE_Psi_pend).*sin(THE_Psi).*sin(THE_Psi_pend).*sin(THE_Theta_pend).*(2.0./3.0)+Lz_pend.*THE_Psi_D.*Tv_Z_pend.*m_pend.*cos(THE_Psi).*cos(THE_Theta).*cos(THE_Phi_pend).*cos(THE_Psi_pend).*cos(THE_Theta_pend)-(Ly_pend.^2.*THE_Phi_D.*m_pend.*cos(THE_Psi).*cos(THE_Theta).^2.*cos(THE_Psi_pend).^2.*cos(THE_Theta_pend).^2.*sin(THE_Psi).*sin(THE_Phi_pend))./6.0+Lz_pend.^2.*THE_Phi_D.*m_pend.*cos(THE_Psi).*cos(THE_Theta).^2.*cos(THE_Psi_pend).^2.*cos(THE_Theta_pend).^2.*sin(THE_Psi).*sin(THE_Phi_pend).*(2.0./3.0)+(Ly_pend.^2.*THE_Theta_D.*m_pend.*cos(THE_Psi_pend).*sin(THE_Psi).*sin(THE_Theta).*sin(THE_Phi_pend).*sin(THE_Psi_pend).*sin(THE_Theta_pend))./6.0-Lz_pend.^2.*THE_Theta_D.*m_pend.*cos(THE_Psi_pend).*sin(THE_Psi).*sin(THE_Theta).*sin(THE_Phi_pend).*sin(THE_Psi_pend).*sin(THE_Theta_pend).*(2.0./3.0)+Lz_pend.*THE_Theta_D.*Tv_Z_pend.*m_pend.*cos(THE_Psi).*cos(THE_Theta).*cos(THE_Psi_pend).*sin(THE_Psi).*sin(THE_Theta_pend);
    et90 = (Lx_pend.^2.*THE_Theta_D.*m_pend.*cos(THE_Psi).*cos(THE_Theta).*cos(THE_Phi_pend).^2.*cos(THE_Theta_pend).*sin(THE_Psi).*sin(THE_Theta_pend))./6.0-(Ly_pend.^2.*THE_Theta_D.*m_pend.*cos(THE_Psi).*cos(THE_Theta).*cos(THE_Phi_pend).^2.*cos(THE_Theta_pend).*sin(THE_Psi).*sin(THE_Theta_pend))./6.0-(Ly_pend.^2.*THE_Theta_D.*m_pend.*cos(THE_Psi).*cos(THE_Theta).*cos(THE_Psi_pend).^2.*cos(THE_Theta_pend).*sin(THE_Psi).*sin(THE_Theta_pend))./3.0+(Ly_pend.^2.*THE_Psi_D.*m_pend.*cos(THE_Theta).*cos(THE_Phi_pend).^2.*cos(THE_Psi_pend).*cos(THE_Theta_pend).*sin(THE_Psi).*sin(THE_Psi_pend))./6.0-(Ly_pend.^2.*THE_Theta_D.*m_pend.*cos(THE_Psi).*cos(THE_Phi_pend).^2.*cos(THE_Psi_pend).*cos(THE_Theta_pend).*sin(THE_Theta).*sin(THE_Psi_pend))./6.0-(Ly_pend.^2.*THE_Theta_D.*m_pend.*cos(THE_Psi).^2.*cos(THE_Theta).*cos(THE_Phi_pend).*cos(THE_Psi_pend).*sin(THE_Psi_pend).*sin(THE_Theta_pend))./6.0+(Ly_pend.^2.*THE_Phi_D.*m_pend.*cos(THE_Theta).^2.*cos(THE_Phi_pend).*cos(THE_Psi_pend).*cos(THE_Theta_pend).*sin(THE_Phi_pend).*sin(THE_Psi_pend))./6.0+Lz_pend.^2.*THE_Theta_D.*m_pend.*cos(THE_Psi).*cos(THE_Theta).*cos(THE_Psi_pend).^2.*cos(THE_Theta_pend).*sin(THE_Psi).*sin(THE_Theta_pend).*(4.0./3.0);
    et91 = Lz_pend.^2.*THE_Psi_D.*m_pend.*cos(THE_Theta).*cos(THE_Phi_pend).^2.*cos(THE_Psi_pend).*cos(THE_Theta_pend).*sin(THE_Psi).*sin(THE_Psi_pend).*(-2.0./3.0)+Lz_pend.^2.*THE_Theta_D.*m_pend.*cos(THE_Psi).*cos(THE_Phi_pend).^2.*cos(THE_Psi_pend).*cos(THE_Theta_pend).*sin(THE_Theta).*sin(THE_Psi_pend).*(2.0./3.0)+Lz_pend.^2.*THE_Theta_D.*m_pend.*cos(THE_Psi).^2.*cos(THE_Theta).*cos(THE_Phi_pend).*cos(THE_Psi_pend).*sin(THE_Psi_pend).*sin(THE_Theta_pend).*(2.0./3.0)-Lz_pend.^2.*THE_Phi_D.*m_pend.*cos(THE_Theta).^2.*cos(THE_Phi_pend).*cos(THE_Psi_pend).*cos(THE_Theta_pend).*sin(THE_Phi_pend).*sin(THE_Psi_pend).*(2.0./3.0)-(Ly_pend.^2.*THE_Phi_D.*m_pend.*cos(THE_Psi).^2.*cos(THE_Theta).^2.*cos(THE_Phi_pend).^2.*cos(THE_Psi_pend).^2.*cos(THE_Theta_pend).*sin(THE_Theta_pend))./1.2e+1+(Lz_pend.^2.*THE_Phi_D.*m_pend.*cos(THE_Psi).^2.*cos(THE_Theta).^2.*cos(THE_Phi_pend).^2.*cos(THE_Psi_pend).^2.*cos(THE_Theta_pend).*sin(THE_Theta_pend))./3.0+Lz_pend.*THE_Theta_D.*Tv_Z_pend.*m_pend.*cos(THE_Psi).^2.*cos(THE_Theta).*cos(THE_Psi_pend).*cos(THE_Theta_pend).*sin(THE_Phi_pend)+(Ly_pend.^2.*THE_Phi_D.*m_pend.*cos(THE_Psi).*cos(THE_Theta).*cos(THE_Phi_pend).*cos(THE_Psi_pend).^2.*cos(THE_Theta_pend).^2.*sin(THE_Theta))./6.0;
    et92 = Lz_pend.^2.*THE_Phi_D.*m_pend.*cos(THE_Psi).*cos(THE_Theta).*cos(THE_Phi_pend).*cos(THE_Psi_pend).^2.*cos(THE_Theta_pend).^2.*sin(THE_Theta).*(-2.0./3.0)+(Lx_pend.^2.*THE_Phi_D.*m_pend.*cos(THE_Theta).*cos(THE_Phi_pend).*cos(THE_Theta_pend).*sin(THE_Psi).*sin(THE_Theta).*sin(THE_Phi_pend).*sin(THE_Theta_pend))./6.0-(Ly_pend.^2.*THE_Phi_D.*m_pend.*cos(THE_Psi).*cos(THE_Theta).*cos(THE_Psi_pend).*sin(THE_Theta).*sin(THE_Phi_pend).*sin(THE_Psi_pend).*sin(THE_Theta_pend))./1.2e+1-(Ly_pend.^2.*THE_Phi_D.*m_pend.*cos(THE_Theta).*cos(THE_Phi_pend).*cos(THE_Theta_pend).*sin(THE_Psi).*sin(THE_Theta).*sin(THE_Phi_pend).*sin(THE_Theta_pend))./6.0+(Lz_pend.^2.*THE_Phi_D.*m_pend.*cos(THE_Psi).*cos(THE_Theta).*cos(THE_Psi_pend).*sin(THE_Theta).*sin(THE_Phi_pend).*sin(THE_Psi_pend).*sin(THE_Theta_pend))./3.0-(Lz_pend.*THE_Phi_D.*Tv_Z_pend.*m_pend.*cos(THE_Psi).*cos(THE_Theta).*cos(THE_Phi_pend).*cos(THE_Psi_pend).*cos(THE_Theta_pend).*sin(THE_Theta))./2.0-(Ly_pend.^2.*THE_Phi_D.*m_pend.*cos(THE_Psi).*cos(THE_Theta).^2.*cos(THE_Phi_pend).*cos(THE_Psi_pend).*sin(THE_Psi).*sin(THE_Psi_pend).*sin(THE_Theta_pend))./1.2e+1-(Ly_pend.^2.*THE_Phi_D.*m_pend.*cos(THE_Theta).*cos(THE_Phi_pend).^2.*cos(THE_Psi_pend).*cos(THE_Theta_pend).*sin(THE_Psi).*sin(THE_Theta).*sin(THE_Psi_pend))./6.0;
    et93 = Ly_pend.^2.*THE_Psi_D.*m_pend.*cos(THE_Theta).*cos(THE_Phi_pend).*cos(THE_Psi_pend).^2.*cos(THE_Theta_pend).*sin(THE_Psi).*sin(THE_Phi_pend).*sin(THE_Theta_pend).*(-1.0./6.0)+(Ly_pend.^2.*THE_Theta_D.*m_pend.*cos(THE_Psi).*cos(THE_Phi_pend).*cos(THE_Psi_pend).^2.*cos(THE_Theta_pend).*sin(THE_Theta).*sin(THE_Phi_pend).*sin(THE_Theta_pend))./6.0+(Lz_pend.^2.*THE_Phi_D.*m_pend.*cos(THE_Psi).*cos(THE_Theta).^2.*cos(THE_Phi_pend).*cos(THE_Psi_pend).*sin(THE_Psi).*sin(THE_Psi_pend).*sin(THE_Theta_pend))./3.0+Lz_pend.^2.*THE_Phi_D.*m_pend.*cos(THE_Theta).*cos(THE_Phi_pend).^2.*cos(THE_Psi_pend).*cos(THE_Theta_pend).*sin(THE_Psi).*sin(THE_Theta).*sin(THE_Psi_pend).*(2.0./3.0)+Lz_pend.^2.*THE_Psi_D.*m_pend.*cos(THE_Theta).*cos(THE_Phi_pend).*cos(THE_Psi_pend).^2.*cos(THE_Theta_pend).*sin(THE_Psi).*sin(THE_Phi_pend).*sin(THE_Theta_pend).*(2.0./3.0)-Lz_pend.^2.*THE_Theta_D.*m_pend.*cos(THE_Psi).*cos(THE_Phi_pend).*cos(THE_Psi_pend).^2.*cos(THE_Theta_pend).*sin(THE_Theta).*sin(THE_Phi_pend).*sin(THE_Theta_pend).*(2.0./3.0)+(Lz_pend.*THE_Phi_D.*Tv_Z_pend.*m_pend.*cos(THE_Psi).*cos(THE_Theta).^2.*cos(THE_Psi_pend).*cos(THE_Theta_pend).*sin(THE_Psi).*sin(THE_Phi_pend))./2.0;
    et94 = (Ly_pend.^2.*THE_Theta_D.*m_pend.*cos(THE_Psi).*cos(THE_Theta).*cos(THE_Phi_pend).^2.*cos(THE_Psi_pend).^2.*cos(THE_Theta_pend).*sin(THE_Psi).*sin(THE_Theta_pend))./6.0-(Ly_pend.^2.*THE_Phi_D.*m_pend.*cos(THE_Psi).^2.*cos(THE_Theta).^2.*cos(THE_Phi_pend).*cos(THE_Psi_pend).*cos(THE_Theta_pend).*sin(THE_Phi_pend).*sin(THE_Psi_pend))./1.2e+1-Lz_pend.^2.*THE_Theta_D.*m_pend.*cos(THE_Psi).*cos(THE_Theta).*cos(THE_Phi_pend).^2.*cos(THE_Psi_pend).^2.*cos(THE_Theta_pend).*sin(THE_Psi).*sin(THE_Theta_pend).*(2.0./3.0)+(Lz_pend.^2.*THE_Phi_D.*m_pend.*cos(THE_Psi).^2.*cos(THE_Theta).^2.*cos(THE_Phi_pend).*cos(THE_Psi_pend).*cos(THE_Theta_pend).*sin(THE_Phi_pend).*sin(THE_Psi_pend))./3.0+(Ly_pend.^2.*THE_Phi_D.*m_pend.*cos(THE_Theta).*cos(THE_Phi_pend).*cos(THE_Psi_pend).^2.*cos(THE_Theta_pend).*sin(THE_Psi).*sin(THE_Theta).*sin(THE_Phi_pend).*sin(THE_Theta_pend))./6.0-Lz_pend.^2.*THE_Phi_D.*m_pend.*cos(THE_Theta).*cos(THE_Phi_pend).*cos(THE_Psi_pend).^2.*cos(THE_Theta_pend).*sin(THE_Psi).*sin(THE_Theta).*sin(THE_Phi_pend).*sin(THE_Theta_pend).*(2.0./3.0)+(Ly_pend.^2.*THE_Theta_D.*m_pend.*cos(THE_Psi).*cos(THE_Theta).*cos(THE_Phi_pend).*cos(THE_Psi_pend).*cos(THE_Theta_pend).*sin(THE_Psi).*sin(THE_Phi_pend).*sin(THE_Psi_pend))./6.0;
    et95 = Lz_pend.^2.*THE_Theta_D.*m_pend.*cos(THE_Psi).*cos(THE_Theta).*cos(THE_Phi_pend).*cos(THE_Psi_pend).*cos(THE_Theta_pend).*sin(THE_Psi).*sin(THE_Phi_pend).*sin(THE_Psi_pend).*(-2.0./3.0);
    et96 = Ly_pend.^2.*THE_Phi_D.*m_pend.*sin(THE_Phi_pend.*2.0).*(-1.0./2.4e+1)+(Lz_pend.^2.*THE_Phi_D.*m_pend.*sin(THE_Phi_pend.*2.0))./6.0-(Ly_pend.^2.*THE_Psi_D.*m_pend.*cos(THE_Theta).*sin(THE_Psi))./6.0-(Ly_pend.^2.*THE_Theta_pend_D.*m_pend.*cos(THE_Phi_pend).*sin(THE_Theta))./6.0-Lz_pend.^2.*THE_Theta_D.*m_pend.*cos(THE_Psi).*sin(THE_Theta).*(2.0./3.0)+(Ly_pend.^2.*THE_Phi_D.*m_pend.*cos(THE_Theta).*sin(THE_Psi).*sin(THE_Theta))./1.2e+1+(Ly_pend.^2.*THE_Psi_D.*m_pend.*cos(THE_Phi_pend).*sin(THE_Theta).*sin(THE_Phi_pend))./6.0+(Ly_pend.^2.*THE_Theta_pend_D.*m_pend.*cos(THE_Theta).*sin(THE_Psi).*sin(THE_Phi_pend))./6.0+(Ly_pend.^2.*THE_Phi_D.*m_pend.*cos(THE_Psi_pend).*sin(THE_Psi_pend).*sin(THE_Theta_pend))./1.2e+1-(Lz_pend.^2.*THE_Phi_D.*m_pend.*cos(THE_Theta).*sin(THE_Psi).*sin(THE_Theta))./3.0-Lz_pend.^2.*THE_Psi_D.*m_pend.*cos(THE_Phi_pend).*sin(THE_Theta).*sin(THE_Phi_pend).*(2.0./3.0)-(Lz_pend.^2.*THE_Phi_D.*m_pend.*cos(THE_Psi_pend).*sin(THE_Psi_pend).*sin(THE_Theta_pend))./3.0-Lz_pend.^2.*THE_Psi_pend_D.*m_pend.*cos(THE_Theta_pend).*sin(THE_Theta).*sin(THE_Phi_pend).*(2.0./3.0);
    et97 = Lx_pend.^2.*THE_Psi_D.*m_pend.*cos(THE_Theta).*cos(THE_Theta_pend).^2.*sin(THE_Psi).*(-1.0./6.0)-(Lx_pend.^2.*THE_Phi_D.*m_pend.*cos(THE_Phi_pend).*cos(THE_Theta_pend).^2.*sin(THE_Phi_pend))./1.2e+1-(Lx_pend.^2.*THE_Theta_pend_D.*m_pend.*cos(THE_Phi_pend).*cos(THE_Theta_pend).^2.*sin(THE_Theta))./6.0+(Ly_pend.^2.*THE_Psi_D.*m_pend.*cos(THE_Theta).*cos(THE_Phi_pend).^2.*sin(THE_Psi))./6.0+(Ly_pend.^2.*THE_Psi_D.*m_pend.*cos(THE_Theta).*cos(THE_Psi_pend).^2.*sin(THE_Psi))./6.0-(Ly_pend.^2.*THE_Theta_D.*m_pend.*cos(THE_Psi).*cos(THE_Phi_pend).^2.*sin(THE_Theta))./6.0+(Ly_pend.^2.*THE_Psi_D.*m_pend.*cos(THE_Theta).*cos(THE_Theta_pend).^2.*sin(THE_Psi))./6.0-(Ly_pend.^2.*THE_Theta_D.*m_pend.*cos(THE_Psi).*cos(THE_Psi_pend).^2.*sin(THE_Theta))./6.0+(Ly_pend.^2.*THE_Phi_D.*m_pend.*cos(THE_Theta).^2.*cos(THE_Phi_pend).*sin(THE_Phi_pend))./6.0+(Ly_pend.^2.*THE_Phi_D.*m_pend.*cos(THE_Phi_pend).*cos(THE_Psi_pend).^2.*sin(THE_Phi_pend))./6.0+(Ly_pend.^2.*THE_Phi_D.*m_pend.*cos(THE_Phi_pend).*cos(THE_Theta_pend).^2.*sin(THE_Phi_pend))./1.2e+1;
    et98 = (Ly_pend.^2.*THE_Theta_pend_D.*m_pend.*cos(THE_Phi_pend).*cos(THE_Psi_pend).^2.*sin(THE_Theta))./6.0+(Ly_pend.^2.*THE_Theta_pend_D.*m_pend.*cos(THE_Phi_pend).*cos(THE_Theta_pend).^2.*sin(THE_Theta))./6.0-Lz_pend.^2.*THE_Psi_D.*m_pend.*cos(THE_Theta).*cos(THE_Phi_pend).^2.*sin(THE_Psi).*(2.0./3.0)-Lz_pend.^2.*THE_Psi_D.*m_pend.*cos(THE_Theta).*cos(THE_Psi_pend).^2.*sin(THE_Psi).*(2.0./3.0)+Lz_pend.^2.*THE_Theta_D.*m_pend.*cos(THE_Psi).*cos(THE_Phi_pend).^2.*sin(THE_Theta).*(2.0./3.0)+Lz_pend.^2.*THE_Theta_D.*m_pend.*cos(THE_Psi).*cos(THE_Psi_pend).^2.*sin(THE_Theta).*(2.0./3.0)-Lz_pend.^2.*THE_Phi_D.*m_pend.*cos(THE_Theta).^2.*cos(THE_Phi_pend).*sin(THE_Phi_pend).*(2.0./3.0)-Lz_pend.^2.*THE_Phi_D.*m_pend.*cos(THE_Phi_pend).*cos(THE_Psi_pend).^2.*sin(THE_Phi_pend).*(2.0./3.0)-Lz_pend.^2.*THE_Theta_pend_D.*m_pend.*cos(THE_Phi_pend).*cos(THE_Psi_pend).^2.*sin(THE_Theta).*(2.0./3.0)+(Lx_pend.^2.*THE_Phi_D.*m_pend.*cos(THE_Theta).*cos(THE_Theta_pend).^2.*sin(THE_Psi).*sin(THE_Theta))./1.2e+1+(Lx_pend.^2.*THE_Psi_D.*m_pend.*cos(THE_Phi_pend).*cos(THE_Theta_pend).^2.*sin(THE_Theta).*sin(THE_Phi_pend))./6.0;
    et99 = (Lx_pend.^2.*THE_Theta_pend_D.*m_pend.*cos(THE_Theta).*cos(THE_Theta_pend).^2.*sin(THE_Psi).*sin(THE_Phi_pend))./6.0-(Ly_pend.^2.*THE_Phi_D.*m_pend.*cos(THE_Theta).*cos(THE_Phi_pend).^2.*sin(THE_Psi).*sin(THE_Theta))./6.0-(Ly_pend.^2.*THE_Phi_D.*m_pend.*cos(THE_Theta).*cos(THE_Psi_pend).^2.*sin(THE_Psi).*sin(THE_Theta))./6.0-(Ly_pend.^2.*THE_Phi_D.*m_pend.*cos(THE_Theta).*cos(THE_Theta_pend).^2.*sin(THE_Psi).*sin(THE_Theta))./1.2e+1-(Ly_pend.^2.*THE_Psi_D.*m_pend.*cos(THE_Phi_pend).*cos(THE_Psi_pend).^2.*sin(THE_Theta).*sin(THE_Phi_pend))./3.0-(Ly_pend.^2.*THE_Psi_D.*m_pend.*cos(THE_Phi_pend).*cos(THE_Theta_pend).^2.*sin(THE_Theta).*sin(THE_Phi_pend))./6.0-(Ly_pend.^2.*THE_Phi_D.*m_pend.*cos(THE_Theta).^2.*cos(THE_Psi_pend).*sin(THE_Psi_pend).*sin(THE_Theta_pend))./6.0-(Ly_pend.^2.*THE_Theta_pend_D.*m_pend.*cos(THE_Theta).*cos(THE_Psi_pend).^2.*sin(THE_Psi).*sin(THE_Phi_pend))./6.0-(Ly_pend.^2.*THE_Theta_pend_D.*m_pend.*cos(THE_Theta).*cos(THE_Theta_pend).^2.*sin(THE_Psi).*sin(THE_Phi_pend))./6.0-(Ly_pend.^2.*THE_Phi_D.*m_pend.*cos(THE_Phi_pend).^2.*cos(THE_Psi_pend).*sin(THE_Psi_pend).*sin(THE_Theta_pend))./6.0;
    et100 = Ly_pend.^2.*THE_Psi_pend_D.*m_pend.*cos(THE_Psi_pend).^2.*cos(THE_Theta_pend).*sin(THE_Theta).*sin(THE_Phi_pend).*(-1.0./6.0)+Lz_pend.^2.*THE_Phi_D.*m_pend.*cos(THE_Theta).*cos(THE_Phi_pend).^2.*sin(THE_Psi).*sin(THE_Theta).*(2.0./3.0)+Lz_pend.^2.*THE_Phi_D.*m_pend.*cos(THE_Theta).*cos(THE_Psi_pend).^2.*sin(THE_Psi).*sin(THE_Theta).*(2.0./3.0)+Lz_pend.^2.*THE_Psi_D.*m_pend.*cos(THE_Phi_pend).*cos(THE_Psi_pend).^2.*sin(THE_Theta).*sin(THE_Phi_pend).*(4.0./3.0)+Lz_pend.^2.*THE_Phi_D.*m_pend.*cos(THE_Theta).^2.*cos(THE_Psi_pend).*sin(THE_Psi_pend).*sin(THE_Theta_pend).*(2.0./3.0)+Lz_pend.^2.*THE_Theta_pend_D.*m_pend.*cos(THE_Theta).*cos(THE_Psi_pend).^2.*sin(THE_Psi).*sin(THE_Phi_pend).*(2.0./3.0)+Lz_pend.^2.*THE_Phi_D.*m_pend.*cos(THE_Phi_pend).^2.*cos(THE_Psi_pend).*sin(THE_Psi_pend).*sin(THE_Theta_pend).*(2.0./3.0)+Lz_pend.^2.*THE_Psi_pend_D.*m_pend.*cos(THE_Psi_pend).^2.*cos(THE_Theta_pend).*sin(THE_Theta).*sin(THE_Phi_pend).*(2.0./3.0)+(Lx_pend.^2.*THE_Psi_D.*m_pend.*cos(THE_Theta).*cos(THE_Phi_pend).^2.*cos(THE_Theta_pend).^2.*sin(THE_Psi))./6.0-(Lx_pend.^2.*THE_Theta_D.*m_pend.*cos(THE_Psi).*cos(THE_Phi_pend).^2.*cos(THE_Theta_pend).^2.*sin(THE_Theta))./6.0;
    et101 = (Lx_pend.^2.*THE_Phi_D.*m_pend.*cos(THE_Theta).^2.*cos(THE_Phi_pend).*cos(THE_Theta_pend).^2.*sin(THE_Phi_pend))./6.0-(Ly_pend.^2.*THE_Phi_D.*m_pend.*cos(THE_Psi).^2.*cos(THE_Theta).^2.*cos(THE_Phi_pend).*sin(THE_Phi_pend))./1.2e+1-(Ly_pend.^2.*THE_Psi_D.*m_pend.*cos(THE_Theta).*cos(THE_Phi_pend).^2.*cos(THE_Psi_pend).^2.*sin(THE_Psi))./3.0-(Ly_pend.^2.*THE_Psi_D.*m_pend.*cos(THE_Theta).*cos(THE_Phi_pend).^2.*cos(THE_Theta_pend).^2.*sin(THE_Psi))./6.0+(Ly_pend.^2.*THE_Theta_D.*m_pend.*cos(THE_Psi).*cos(THE_Phi_pend).^2.*cos(THE_Psi_pend).^2.*sin(THE_Theta))./3.0-(Ly_pend.^2.*THE_Psi_D.*m_pend.*cos(THE_Theta).*cos(THE_Psi_pend).^2.*cos(THE_Theta_pend).^2.*sin(THE_Psi))./6.0+(Ly_pend.^2.*THE_Theta_D.*m_pend.*cos(THE_Psi).*cos(THE_Phi_pend).^2.*cos(THE_Theta_pend).^2.*sin(THE_Theta))./6.0-(Ly_pend.^2.*THE_Phi_D.*m_pend.*cos(THE_Theta).^2.*cos(THE_Phi_pend).*cos(THE_Psi_pend).^2.*sin(THE_Phi_pend))./3.0-(Ly_pend.^2.*THE_Phi_D.*m_pend.*cos(THE_Theta).^2.*cos(THE_Phi_pend).*cos(THE_Theta_pend).^2.*sin(THE_Phi_pend))./6.0;
    et102 = Ly_pend.^2.*THE_Phi_D.*m_pend.*cos(THE_Phi_pend).*cos(THE_Psi_pend).^2.*cos(THE_Theta_pend).^2.*sin(THE_Phi_pend).*(-1.0./1.2e+1)-(Ly_pend.^2.*THE_Theta_pend_D.*m_pend.*cos(THE_Phi_pend).*cos(THE_Psi_pend).^2.*cos(THE_Theta_pend).^2.*sin(THE_Theta))./6.0+(Lz_pend.^2.*THE_Phi_D.*m_pend.*cos(THE_Psi).^2.*cos(THE_Theta).^2.*cos(THE_Phi_pend).*sin(THE_Phi_pend))./3.0+Lz_pend.^2.*THE_Psi_D.*m_pend.*cos(THE_Theta).*cos(THE_Phi_pend).^2.*cos(THE_Psi_pend).^2.*sin(THE_Psi).*(4.0./3.0)-Lz_pend.^2.*THE_Theta_D.*m_pend.*cos(THE_Psi).*cos(THE_Phi_pend).^2.*cos(THE_Psi_pend).^2.*sin(THE_Theta).*(4.0./3.0)+Lz_pend.^2.*THE_Psi_D.*m_pend.*cos(THE_Theta).*cos(THE_Psi_pend).^2.*cos(THE_Theta_pend).^2.*sin(THE_Psi).*(2.0./3.0)+Lz_pend.^2.*THE_Phi_D.*m_pend.*cos(THE_Theta).^2.*cos(THE_Phi_pend).*cos(THE_Psi_pend).^2.*sin(THE_Phi_pend).*(4.0./3.0)+(Lz_pend.^2.*THE_Phi_D.*m_pend.*cos(THE_Phi_pend).*cos(THE_Psi_pend).^2.*cos(THE_Theta_pend).^2.*sin(THE_Phi_pend))./3.0+Lz_pend.^2.*THE_Theta_pend_D.*m_pend.*cos(THE_Phi_pend).*cos(THE_Psi_pend).^2.*cos(THE_Theta_pend).^2.*sin(THE_Theta).*(2.0./3.0);
    et103 = Lx_pend.^2.*THE_Theta_pend_D.*m_pend.*cos(THE_Psi).*cos(THE_Theta).*cos(THE_Theta_pend).*sin(THE_Theta_pend).*(-1.0./6.0)+(Ly_pend.^2.*THE_Theta_pend_D.*m_pend.*cos(THE_Psi).*cos(THE_Theta).*cos(THE_Theta_pend).*sin(THE_Theta_pend))./6.0-Lz_pend.^2.*THE_Psi_pend_D.*m_pend.*cos(THE_Theta).*cos(THE_Phi_pend).*cos(THE_Theta_pend).*sin(THE_Psi).*(2.0./3.0)-(Ly_pend.^2.*THE_Psi_D.*m_pend.*cos(THE_Psi_pend).*sin(THE_Theta).*sin(THE_Psi_pend).*sin(THE_Theta_pend))./6.0+Lz_pend.^2.*THE_Psi_D.*m_pend.*cos(THE_Psi_pend).*sin(THE_Theta).*sin(THE_Psi_pend).*sin(THE_Theta_pend).*(2.0./3.0)+Lz_pend.*THE_Theta_D.*Tv_Z_pend.*m_pend.*cos(THE_Psi).^2.*cos(THE_Theta).*sin(THE_Phi_pend).*sin(THE_Psi_pend)-(Lx_pend.^2.*THE_Phi_D.*m_pend.*cos(THE_Theta).*cos(THE_Phi_pend).^2.*cos(THE_Theta_pend).^2.*sin(THE_Psi).*sin(THE_Theta))./6.0+(Ly_pend.^2.*THE_Phi_D.*m_pend.*cos(THE_Theta).*cos(THE_Phi_pend).^2.*cos(THE_Psi_pend).^2.*sin(THE_Psi).*sin(THE_Theta))./3.0+(Ly_pend.^2.*THE_Phi_D.*m_pend.*cos(THE_Theta).*cos(THE_Phi_pend).^2.*cos(THE_Theta_pend).^2.*sin(THE_Psi).*sin(THE_Theta))./6.0+(Ly_pend.^2.*THE_Phi_D.*m_pend.*cos(THE_Theta).*cos(THE_Psi_pend).^2.*cos(THE_Theta_pend).^2.*sin(THE_Psi).*sin(THE_Theta))./1.2e+1;
    et104 = (Ly_pend.^2.*THE_Phi_D.*m_pend.*cos(THE_Psi).^2.*cos(THE_Theta).^2.*cos(THE_Psi_pend).*sin(THE_Psi_pend).*sin(THE_Theta_pend))./1.2e+1+(Ly_pend.^2.*THE_Phi_D.*m_pend.*cos(THE_Theta).^2.*cos(THE_Phi_pend).^2.*cos(THE_Psi_pend).*sin(THE_Psi_pend).*sin(THE_Theta_pend))./3.0+(Ly_pend.^2.*THE_Psi_D.*m_pend.*cos(THE_Phi_pend).*cos(THE_Psi_pend).^2.*cos(THE_Theta_pend).^2.*sin(THE_Theta).*sin(THE_Phi_pend))./6.0+(Ly_pend.^2.*THE_Theta_pend_D.*m_pend.*cos(THE_Theta).*cos(THE_Psi_pend).^2.*cos(THE_Theta_pend).^2.*sin(THE_Psi).*sin(THE_Phi_pend))./6.0-Lz_pend.^2.*THE_Phi_D.*m_pend.*cos(THE_Theta).*cos(THE_Phi_pend).^2.*cos(THE_Psi_pend).^2.*sin(THE_Psi).*sin(THE_Theta).*(4.0./3.0)-(Lz_pend.^2.*THE_Phi_D.*m_pend.*cos(THE_Theta).*cos(THE_Psi_pend).^2.*cos(THE_Theta_pend).^2.*sin(THE_Psi).*sin(THE_Theta))./3.0-(Lz_pend.^2.*THE_Phi_D.*m_pend.*cos(THE_Psi).^2.*cos(THE_Theta).^2.*cos(THE_Psi_pend).*sin(THE_Psi_pend).*sin(THE_Theta_pend))./3.0-Lz_pend.^2.*THE_Phi_D.*m_pend.*cos(THE_Theta).^2.*cos(THE_Phi_pend).^2.*cos(THE_Psi_pend).*sin(THE_Psi_pend).*sin(THE_Theta_pend).*(4.0./3.0);
    et105 = Lz_pend.^2.*THE_Psi_D.*m_pend.*cos(THE_Phi_pend).*cos(THE_Psi_pend).^2.*cos(THE_Theta_pend).^2.*sin(THE_Theta).*sin(THE_Phi_pend).*(-2.0./3.0)-Lz_pend.^2.*THE_Theta_pend_D.*m_pend.*cos(THE_Theta).*cos(THE_Psi_pend).^2.*cos(THE_Theta_pend).^2.*sin(THE_Psi).*sin(THE_Phi_pend).*(2.0./3.0)+(Lx_pend.^2.*THE_Psi_D.*m_pend.*cos(THE_Psi).*cos(THE_Theta).*cos(THE_Theta_pend).*sin(THE_Phi_pend).*sin(THE_Theta_pend))./6.0+(Ly_pend.^2.*THE_Theta_D.*m_pend.*cos(THE_Psi).*cos(THE_Theta).*cos(THE_Phi_pend).*sin(THE_Psi).*sin(THE_Phi_pend))./6.0-(Ly_pend.^2.*THE_Psi_D.*m_pend.*cos(THE_Psi).*cos(THE_Theta).*cos(THE_Theta_pend).*sin(THE_Phi_pend).*sin(THE_Theta_pend))./6.0-Lz_pend.^2.*THE_Theta_D.*m_pend.*cos(THE_Psi).*cos(THE_Theta).*cos(THE_Phi_pend).*sin(THE_Psi).*sin(THE_Phi_pend).*(2.0./3.0)-(Lx_pend.^2.*THE_Phi_D.*m_pend.*cos(THE_Psi).^2.*cos(THE_Theta).^2.*cos(THE_Phi_pend).*cos(THE_Theta_pend).^2.*sin(THE_Phi_pend))./1.2e+1+(Ly_pend.^2.*THE_Phi_D.*m_pend.*cos(THE_Psi).^2.*cos(THE_Theta).^2.*cos(THE_Phi_pend).*cos(THE_Psi_pend).^2.*sin(THE_Phi_pend))./6.0;
    et106 = (Ly_pend.^2.*THE_Phi_D.*m_pend.*cos(THE_Psi).^2.*cos(THE_Theta).^2.*cos(THE_Phi_pend).*cos(THE_Theta_pend).^2.*sin(THE_Phi_pend))./1.2e+1+(Ly_pend.^2.*THE_Psi_D.*m_pend.*cos(THE_Theta).*cos(THE_Phi_pend).^2.*cos(THE_Psi_pend).^2.*cos(THE_Theta_pend).^2.*sin(THE_Psi))./6.0-(Ly_pend.^2.*THE_Theta_D.*m_pend.*cos(THE_Psi).*cos(THE_Phi_pend).^2.*cos(THE_Psi_pend).^2.*cos(THE_Theta_pend).^2.*sin(THE_Theta))./6.0+(Ly_pend.^2.*THE_Phi_D.*m_pend.*cos(THE_Theta).^2.*cos(THE_Phi_pend).*cos(THE_Psi_pend).^2.*cos(THE_Theta_pend).^2.*sin(THE_Phi_pend))./6.0-Lz_pend.^2.*THE_Phi_D.*m_pend.*cos(THE_Psi).^2.*cos(THE_Theta).^2.*cos(THE_Phi_pend).*cos(THE_Psi_pend).^2.*sin(THE_Phi_pend).*(2.0./3.0)-Lz_pend.^2.*THE_Psi_D.*m_pend.*cos(THE_Theta).*cos(THE_Phi_pend).^2.*cos(THE_Psi_pend).^2.*cos(THE_Theta_pend).^2.*sin(THE_Psi).*(2.0./3.0)+Lz_pend.^2.*THE_Theta_D.*m_pend.*cos(THE_Psi).*cos(THE_Phi_pend).^2.*cos(THE_Psi_pend).^2.*cos(THE_Theta_pend).^2.*sin(THE_Theta).*(2.0./3.0);
    et107 = Lz_pend.^2.*THE_Phi_D.*m_pend.*cos(THE_Theta).^2.*cos(THE_Phi_pend).*cos(THE_Psi_pend).^2.*cos(THE_Theta_pend).^2.*sin(THE_Phi_pend).*(-2.0./3.0)+(Ly_pend.^2.*THE_Theta_pend_D.*m_pend.*cos(THE_Psi_pend).*sin(THE_Theta).*sin(THE_Phi_pend).*sin(THE_Psi_pend).*sin(THE_Theta_pend))./6.0-Lz_pend.^2.*THE_Theta_pend_D.*m_pend.*cos(THE_Psi_pend).*sin(THE_Theta).*sin(THE_Phi_pend).*sin(THE_Psi_pend).*sin(THE_Theta_pend).*(2.0./3.0)+Lz_pend.*THE_Psi_D.*Tv_Z_pend.*m_pend.*cos(THE_Psi).*cos(THE_Theta).*cos(THE_Phi_pend).*sin(THE_Psi_pend)-(Lx_pend.^2.*THE_Theta_D.*m_pend.*cos(THE_Psi).^2.*cos(THE_Theta).*cos(THE_Phi_pend).*cos(THE_Theta_pend).*sin(THE_Theta_pend))./6.0+(Ly_pend.^2.*THE_Theta_D.*m_pend.*cos(THE_Psi).^2.*cos(THE_Theta).*cos(THE_Phi_pend).*cos(THE_Theta_pend).*sin(THE_Theta_pend))./6.0-(Ly_pend.^2.*THE_Psi_pend_D.*m_pend.*cos(THE_Theta).*cos(THE_Phi_pend).*cos(THE_Psi_pend).^2.*cos(THE_Theta_pend).*sin(THE_Psi))./6.0-(Ly_pend.^2.*THE_Psi_pend_D.*m_pend.*cos(THE_Psi).*cos(THE_Theta).*cos(THE_Psi_pend).*cos(THE_Theta_pend).^2.*sin(THE_Psi_pend))./6.0-(Ly_pend.^2.*THE_Theta_pend_D.*m_pend.*cos(THE_Psi).*cos(THE_Theta).*cos(THE_Psi_pend).^2.*cos(THE_Theta_pend).*sin(THE_Theta_pend))./6.0;
